simulink model "Dinamica_numerica_MPC"  (R2024b)
settings: Solver=ode4  StartTime=0.0  StopTime=Durata_sim  FixedStep=step_num  RelTol=1e-6
values from neighbouring files (symbols this model uses):
  a_c0 = 6771    [Propagation_outofplane_transfer.m]
  B_c = C_Dc*S_c/mass_c    (= 0)    [Propagation_outofplane_transfer.m]
  B_d = C_Dd*S_d/mass_d    (= 1.05e-08)    [Propagation_outofplane_transfer.m]
  D = zeros(ny,3)    [final_controller_1deputy2.m]
  delta_a0 = 0    [Propagation_outofplane_transfer.m]
  delta_B = (B_d-B_c)/B_d    (= 1)    [Propagation_outofplane_transfer.m]
  delta_e_x0 = 0    [Propagation_outofplane_transfer.m]
  delta_e_y0 = 0.2/a_c0    (= 2.95377344558e-05)    [Propagation_outofplane_transfer.m]
  delta_i_x0 = 0    [Propagation_outofplane_transfer.m]
  delta_i_y0 = 0.18/a_c0    (= 2.65839610102e-05)    [Propagation_outofplane_transfer.m]
  delta_lambda0 = 0    [Propagation_outofplane_transfer.m]
  e_c0 = 0.001    [Propagation_outofplane_transfer.m]
  i_c0 = 97.05 * pi/180    (= 1.69384203906)    [Propagation_outofplane_transfer.m]
  J_2 = 1.08263e-3    (= 0.00108263)    [Propagation_outofplane_transfer.m]
  M_c0 = 0 * pi/180    (= 0)    [Propagation_outofplane_transfer.m]
  mu = 3.986e5    (= 398600)    [Propagation_outofplane_transfer.m]
  OM_c0 = 30 * pi/180    (= 0.523598775598)    [Propagation_outofplane_transfer.m]
  om_c0 = 90 * pi/180    (= 1.57079632679)    [Propagation_outofplane_transfer.m]
  R_E = 6378    [Propagation_outofplane_transfer.m]
  rho = 1.05259630795205e-3    (= 0.00105259630795)    [Propagation_outofplane_transfer.m]
  ROE_T = [delta_aT,delta_lambdaT,delta_e_xT,delta_e_yT, delta_i_xT, delta_i_yT, delta_B]'    [Propagation_outofplane_transfer.m]
  S_c = 0.1*(1e-3)^2    (= 1e-07)    [Propagation_outofplane_transfer.m]
  S_d = 0.1*(1e-3)^2    (= 1e-07)    [Propagation_outofplane_transfer.m]
  T_orbit = 2*pi/n_c0    [Propagation_outofplane_transfer.m]
  Ts = 100    [Propagation_outofplane_transfer.m]
  u_max = max_thrust/mass_d    (= 3.25e-08)    [Propagation_outofplane_transfer.m]    (also in final_controller_1deputy2.m = 0.0325)
  u_min = min_thrust/mass_d    (= 1.75e-08)    [Propagation_outofplane_transfer.m]    (also in final_controller_1deputy2.m = 0.0175)
undefined symbols (not defined in the file or in its folder): final_controller_1deputy2, inputs4JB2008, JB2008, M_0, OMEGA_c0, omega_c0
libraries: spsMeanLib x6, simulink x3, simulink_extras x2
(part 2 of 4)

== matlab function Dinamica_numerica_MPC/Linearized ROE computing ==
  settings: updateMethod=DISCRETE
  data: ROE input; J_2 input; rho input; A output; OE_c input; B_c input; B_d input; B output
function [A,B] = matrices_comput(ROE, J_2, rho, OE_c, B_c, B_d)
%%%%%%%%%%%%%%%%%%%%%%%%%%%%%%%%%%%%%%%%%%%%%%%%%%%%%%%%%%%%%%%%%%%%%%
% DOCUMENTATION:
% The following function propagate the Relative Orbital Elements (ROE)
% of a Deputy satellite wrt a Chief satellite with known chief OE.
% The orbit dynamics is expressed in linearized form such that the
% dynamics of chief-deputy system can be expressed by the following:
% -     dx = (A_kep + A_J2 + A_drag) * x + B * u
% where A_kep is the State Transition Matrix (STM) representing the EoM
% of a keplerian two-body system, A_J2 is the STM embedding the J2
% effect, and A_drag is the STM that take into account the approximated
% drag model. Note that the perturbation STM are time-varying matricies, thus the model
% can be updated with a certain externally defined period
% 
% INPUTS:
% - x       -> ROE of Deputy satellite wrt Chief
% - u       -> Input thrust dor the Deputy satellite
% - trg     -> Trigger signal for STM update
% - pert_flg-> Perturbation flags: (1) J2, (2) Drag
% - OEc     -> Chief orbit element organized
% 
% OUTPUTS:
% - dx      -> ROE derivate
% 
% REFEREBCES:           %TO BE ADDED
% []
% []
% []

%%%%%%%%%%%%%%%%%%%%%%%%%%%%%%%%%%%%%%%%%%%%%%%%%%%%%%%%%%%%%%%%%%%%%%


mu  = 3.986e5;
R_E = 6378;

a_c  = OE_c(1);
e_c  = OE_c(2);
i_c  = OE_c(3);

i_c = mod(i_c, 2*pi);        % assicura che i sia tra 0 e 2π
if i_c > pi
    i_c = 2*pi - i_c;             % lo porta nel range [0, π]
end

OM_c = OE_c(4);
OM_c = mod(OM_c, 2*pi);
om_c = OE_c(5);
om_c = mod(om_c, 2*pi);
M_c  = OE_c(6);
M_c = mod(M_c, 2*pi);





% nu_c= mean2true(M_c,e_c);
% Io invece farei:
nu_c = Tempo_inverso_aggiustato(M_c, a_c, e_c);
n_c = sqrt(mu/a_c^3);
u_c = om_c + M_c;
p_c   = a_c*(1-e_c^2);
v_c = sqrt(mu/p_c)*sqrt(2*(1+e_c*cos(nu_c))-(1-e_c^2));

% Keplerian EoM STM

A_kep = zeros(7);
A_kep(2,1) = -3/2 * n_c;


eta  = sqrt(1-e_c^2);
k_J2 = 3/4*J_2*R_E^2*sqrt(mu)/(a_c^3.5*eta^4);
e_xc  = e_c*cos(om_c);
e_yc  = e_c*sin(om_c);
E    = 1 + eta;
F    = 4 + 3*eta;
G    = 1/eta^2;
P    = 3*cos(i_c)^2 - 1;
Q    = 5*cos(i_c)^2 - 1;
S    = sin(2*i_c);
T    = sin(i_c)^2;

%%%%%%%%%%%%%%%%%%%%%%%%%%%%%%%%%%%%%%%%%%%%%%%%%%%%%%%%%%%%%%%%%%%%%%%%%%%%%%%%%%%%%%%%%%%%%%%%%%%%%%%%%%%%%%%%%%%%%%%%%%%
% J2 plant matrix computation

% Versione del paper di Guffanti (e anche tesi di Belloni, tranne per un
% errore di copiatura, secondo me, che ho aggiustato)
%(è quella che sto usando al momento)
A_J2 = k_J2.*[zeros(1,7);
              -7/2*E*P, 0, e_xc*G*F*P, e_yc*G*F*P, -F*S, 0, 0;
              7/2*e_yc*Q, 0, -4*e_xc*e_yc*G*Q, -(1+4*G*e_yc^2)*Q, 5*e_yc*S, 0, 0;
              -7/2*e_xc*Q, 0, (1+4*G*e_xc^2)*Q, 4*e_xc*e_yc*G*Q, -5*e_xc*S, 0, 0;
              zeros(1,7);
              7/2*S, 0, -4*e_xc*G*S, -4*e_yc*G*S, 2*T, 0, 0;
              zeros(1,7)];


delta_a = ROE(1);
delta_lambda = ROE(2);
delta_e_x = ROE(3);
delta_e_y=ROE(4);
delta_i_x=ROE(5);
delta_i_y=ROE(6);

%%%%%%%%%%%%%%%%%%%%%%%%%%%%%%%%%%%%%%%%%%%%%%%%%%%%%%%%%%%%%%%%%%%%%%%%%%%%%%%%%%%%%%%%%%%%%%%%%%%%%%%%%%%%%%%%%%%%%%%%%%%%%%%%%%%%%%%%%%%%%%%%%%%%%%%%%%%%%%%%%%%%%%%%%%%%%%%%%

% Drag plant matrix


a_d   = a_c*(delta_a+1);
e_xd = e_xc+delta_e_x;
e_yd = e_yc+delta_e_y;
e_d = sqrt(e_xd^2+e_yd^2);
om_d  = atan2(e_yd,e_xd);
om_d = mod(om_d, 2*pi);
i_d = i_c + delta_i_x;
i_d = mod(i_d, 2*pi);        % assicura che i sia tra 0 e 2π
if i_d > pi
    i_d = 2*pi - i_d;             % lo porta nel range [0, π]
end

OM_d = OM_c + delta_i_y/sin(i_c);
OM_d = mod(OM_d, 2*pi);
u_d = u_c - delta_i_y/tan(i_c) + delta_lambda;
u_d = mod(u_d, 2*pi);
M_d = u_d - om_d;
M_d = mod(M_d, 2*pi);



nu_d = Tempo_inverso_aggiustato(M_d, a_d, e_d);
p_d   = a_d*(1-e_d^2);
v_d = sqrt(mu/p_d)*sqrt(2*(1+e_d*cos(nu_d))-(1-e_d^2));
b_d = a_d*sqrt(1-e_d^2); % semiasse minore dell'orbita del deputy
r_d = p_d/(1+e_d*cos(nu_d));

A_drag = zeros(7,7);
delta_M = M_d - M_c;
delta_e = e_d - e_c;
delta_om = om_d - om_c;
delta_i = i_d - i_c;
delta_OM = OM_d - OM_c;

u_drag = 0.5*B_d*rho*v_d^2; % accelerazione dovuta alla resistenza in valore assoluto



%-----------------------------------------------------------------------------------------

% Quella che ho ricavato io NON NINEARIZZANDO, considerando anche delta_lambda_dot, è:
% (è quella che sto usando al momento e che ho usato per ottenere i risultati mostrati a Thales)
% NON CAMBIA NULLA A LIVELLO DI RISULTATI SE USI QUELLA MESSA NELLA TESI,
% PER QUESTO AL MOMENTO USO QUESTA.

delta_B = (B_d-B_c)/B_d; % definizione usata nella tesi di Belloni
A_drag(1:4,7) = - u_drag.*[2*a_d^2 * v_d/(mu*a_c);
                           2/(e_d*v_d)*sin(nu_d)*(1-b_d/a_d*(1+e_d^2*r_d/p_d));
                           2/v_d*((e_d+cos(nu_d))*cos(om_d)-sin(nu_d)*sin(om_d));
                           2/v_d*((e_d+cos(nu_d))*sin(om_d)+sin(nu_d)*cos(om_d))];



%------------------------------------------------------------------------------
% versione linearizzata con definizione di delta_B di Guffanti (cioè quella
% che ho inserito nella tesi)
% 

% delta_B = B_d - B_c; % definizione del paper di Guffanti
% A_drag(1,1) = 0;
% A_drag(1,2) = 0;
% A_drag(1,3) = 0;
% A_drag(1,4) = 0;
% A_drag(1,5) = 0;
% A_drag(1,6) = 0;
% A_drag(1,7) = -(a_c*rho*v_c^3)/mu;
% A_drag(2,1) = 0;
% A_drag(2,2) = 0;
% A_drag(2,3) = 0;
% A_drag(2,4) = 0;
% A_drag(2,5) = 0;
% A_drag(2,6) = 0;
% A_drag(2,7) = 0;
% A_drag(3,1) = 0;
% A_drag(3,2) = 0;
% A_drag(3,3) = 0;
% A_drag(3,4) = 0;
% A_drag(3,5) = 0;
% A_drag(3,6) = 0;
% A_drag(3,7) = rho*v_c*(sin(nu_c)*sin(om_c) - cos(om_c)*(e_c + cos(nu_c)));
% A_drag(4,1) = 0;
% A_drag(4,2) = 0;
% A_drag(4,3) = 0;
% A_drag(4,4) = 0;
% A_drag(4,5) = 0;
% A_drag(4,6) = 0;
% A_drag(4,7) = -rho*v_c*(cos(om_c)*sin(nu_c) + sin(om_c)*(e_c + cos(nu_c)));
% A_drag(5,1) = 0;
% A_drag(5,2) = 0;
% A_drag(5,3) = 0;
% A_drag(5,4) = 0;
% A_drag(5,5) = 0;
% A_drag(5,6) = 0;
% A_drag(5,7) = 0;
% A_drag(6,1) = 0;
% A_drag(6,2) = 0;
% A_drag(6,3) = 0;
% A_drag(6,4) = 0;
% A_drag(6,5) = 0;
% A_drag(6,6) = 0;
% A_drag(6,7) = 0;
% A_drag(7,1) = 0;
% A_drag(7,2) = 0;
% A_drag(7,3) = 0;
% A_drag(7,4) = 0;
% A_drag(7,5) = 0;
% A_drag(7,6) = 0;
% A_drag(7,7) = 0;


%------------------------------------------------------------------------
% versione linearizzata con definizione di delta_B di Koenig

% delta_B = (B_d-B_c)/B_c; % definizione di Koenig
% A_drag(1,1) = ((B_c*a_c*rho*(delta_B + 1)*(-mu/(a_c*(e_xc^2 + e_yc^2 - 1)))^(1/2)*(2*cos(u_c - atan2(e_yc, e_xc) + (13*sin(3*u_c - 3*atan2(e_yc, e_xc))*(e_xc^2 + e_yc^2)^(3/2))/12 + sin(u_c - atan2(e_yc, e_xc))*(2*(e_xc^2 + e_yc^2)^(1/2) - (e_xc^2 + e_yc^2)^(3/2)/4) + sin(2*u_c - 2*atan2(e_yc, e_xc))*((5*e_xc^2)/4 + (5*e_yc^2)/4))*(e_xc^2 + e_yc^2)^(1/2) + e_xc^2 + e_yc^2 + 1)^(3/2))/(e_xc^2 + e_yc^2 - 1) + (B_c*mu*rho*(delta_B + 1)*(2*cos(u_c - atan2(e_yc, e_xc) + (13*sin(3*u_c - 3*atan2(e_yc, e_xc))*(e_xc^2 + e_yc^2)^(3/2))/12 + sin(u_c - atan2(e_yc, e_xc))*(2*(e_xc^2 + e_yc^2)^(1/2) - (e_xc^2 + e_yc^2)^(3/2)/4) + sin(2*u_c - 2*atan2(e_yc, e_xc))*((5*e_xc^2)/4 + (5*e_yc^2)/4))*(e_xc^2 + e_yc^2)^(1/2) + e_xc^2 + e_yc^2 + 1)^(3/2))/(2*(-mu/(a_c*(e_xc^2 + e_yc^2 - 1)))^(1/2)*(e_xc^2 + e_yc^2 - 1)^2))/a_c - (B_c*rho*(-mu/(a_c*(e_c^2 - 1)))^(1/2)*(e_c^2 + 2*e_c*cos(M_c + (5*e_c^2*sin(2*M_c))/4 + (13*e_c^3*sin(3*M_c))/12 + sin(M_c)*(2*e_c - e_c^3/4)) + 1)^(3/2))/(e_c^2 - 1);
% A_drag(1,2) = -(3*B_c*rho*sin(u_c - atan2(e_yc, e_xc) + (13*sin(3*u_c - 3*atan2(e_yc, e_xc))*(e_xc^2 + e_yc^2)^(3/2))/12 + sin(u_c - atan2(e_yc, e_xc))*(2*(e_xc^2 + e_yc^2)^(1/2) - (e_xc^2 + e_yc^2)^(3/2)/4) + sin(2*u_c - 2*atan2(e_yc, e_xc))*((5*e_xc^2)/4 + (5*e_yc^2)/4))*(delta_B + 1)*(e_xc^2 + e_yc^2)^(1/2)*(-mu/(a_c*(e_xc^2 + e_yc^2 - 1)))^(1/2)*(2*cos(u_c - atan2(e_yc, e_xc) + (13*sin(3*u_c - 3*atan2(e_yc, e_xc))*(e_xc^2 + e_yc^2)^(3/2))/12 + sin(u_c - atan2(e_yc, e_xc))*(2*(e_xc^2 + e_yc^2)^(1/2) - (e_xc^2 + e_yc^2)^(3/2)/4) + sin(2*u_c - 2*atan2(e_yc, e_xc))*((5*e_xc^2)/4 + (5*e_yc^2)/4))*(e_xc^2 + e_yc^2)^(1/2) + e_xc^2 + e_yc^2 + 1)^(1/2)*((13*cos(3*u_c - 3*atan2(e_yc, e_xc))*(e_xc^2 + e_yc^2)^(3/2))/4 + cos(u_c - atan2(e_yc, e_xc))*(2*(e_xc^2 + e_yc^2)^(1/2) - (e_xc^2 + e_yc^2)^(3/2)/4) + 2*cos(2*u_c - 2*atan2(e_yc, e_xc))*((5*e_xc^2)/4 + (5*e_yc^2)/4) + 1))/(e_xc^2 + e_yc^2 - 1);
% A_drag(1,3) = ((3*B_c*a_c*rho*(delta_B + 1)*(2*e_xc + (2*e_xc*cos(u_c - atan2(e_yc, e_xc) + (13*sin(3*u_c - 3*atan2(e_yc, e_xc))*(e_xc^2 + e_yc^2)^(3/2))/12 + sin(u_c - atan2(e_yc, e_xc))*(2*(e_xc^2 + e_yc^2)^(1/2) - (e_xc^2 + e_yc^2)^(3/2)/4) + sin(2*u_c - 2*atan2(e_yc, e_xc))*((5*e_xc^2)/4 + (5*e_yc^2)/4)))/(e_xc^2 + e_yc^2)^(1/2) - 2*sin(u_c - atan2(e_yc, e_xc) + (13*sin(3*u_c - 3*atan2(e_yc, e_xc))*(e_xc^2 + e_yc^2)^(3/2))/12 + sin(u_c - atan2(e_yc, e_xc))*(2*(e_xc^2 + e_yc^2)^(1/2) - (e_xc^2 + e_yc^2)^(3/2)/4) + sin(2*u_c - 2*atan2(e_yc, e_xc))*((5*e_xc^2)/4 + (5*e_yc^2)/4))*(e_xc^2 + e_yc^2)^(1/2)*(e_yc/(e_xc^2 + e_yc^2) + sin(u_c - atan2(e_yc, e_xc))*((2*e_xc)/(e_xc^2 + e_yc^2)^(1/2) - (3*e_xc*(e_xc^2 + e_yc^2)^(1/2))/4) + (5*e_xc*sin(2*u_c - 2*atan2(e_yc, e_xc)))/2 + (13*e_yc*cos(3*u_c - 3*atan2(e_yc, e_xc))*(e_xc^2 + e_yc^2)^(1/2))/4 + (13*e_xc*sin(3*u_c - 3*atan2(e_yc, e_xc))*(e_xc^2 + e_yc^2)^(1/2))/4 + (e_yc*cos(u_c - atan2(e_yc, e_xc))*(2*(e_xc^2 + e_yc^2)^(1/2) - (e_xc^2 + e_yc^2)^(3/2)/4))/(e_xc^2 + e_yc^2) + (2*e_yc*cos(2*u_c - 2*atan2(e_yc, e_xc))*((5*e_xc^2)/4 + (5*e_yc^2)/4))/(e_xc^2 + e_yc^2)))*(-mu/(a_c*(e_xc^2 + e_yc^2 - 1)))^(1/2)*(2*cos(u_c - atan2(e_yc, e_xc) + (13*sin(3*u_c - 3*atan2(e_yc, e_xc))*(e_xc^2 + e_yc^2)^(3/2))/12 + sin(u_c - atan2(e_yc, e_xc))*(2*(e_xc^2 + e_yc^2)^(1/2) - (e_xc^2 + e_yc^2)^(3/2)/4) + sin(2*u_c - 2*atan2(e_yc, e_xc))*((5*e_xc^2)/4 + (5*e_yc^2)/4))*(e_xc^2 + e_yc^2)^(1/2) + e_xc^2 + e_yc^2 + 1)^(1/2))/(2*(e_xc^2 + e_yc^2 - 1)) - (2*B_c*a_c*e_xc*rho*(delta_B + 1)*(-mu/(a_c*(e_xc^2 + e_yc^2 - 1)))^(1/2)*(2*cos(u_c - atan2(e_yc, e_xc) + (13*sin(3*u_c - 3*atan2(e_yc, e_xc))*(e_xc^2 + e_yc^2)^(3/2))/12 + sin(u_c - atan2(e_yc, e_xc))*(2*(e_xc^2 + e_yc^2)^(1/2) - (e_xc^2 + e_yc^2)^(3/2)/4) + sin(2*u_c - 2*atan2(e_yc, e_xc))*((5*e_xc^2)/4 + (5*e_yc^2)/4))*(e_xc^2 + e_yc^2)^(1/2) + e_xc^2 + e_yc^2 + 1)^(3/2))/(e_xc^2 + e_yc^2 - 1)^2 + (B_c*e_xc*mu*rho*(delta_B + 1)*(2*cos(u_c - atan2(e_yc, e_xc) + (13*sin(3*u_c - 3*atan2(e_yc, e_xc))*(e_xc^2 + e_yc^2)^(3/2))/12 + sin(u_c - atan2(e_yc, e_xc))*(2*(e_xc^2 + e_yc^2)^(1/2) - (e_xc^2 + e_yc^2)^(3/2)/4) + sin(2*u_c - 2*atan2(e_yc, e_xc))*((5*e_xc^2)/4 + (5*e_yc^2)/4))*(e_xc^2 + e_yc^2)^(1/2) + e_xc^2 + e_yc^2 + 1)^(3/2))/((-mu/(a_c*(e_xc^2 + e_yc^2 - 1)))^(1/2)*(e_xc^2 + e_yc^2 - 1)^3))/a_c;
% A_drag(1,4) = ((3*B_c*a_c*rho*(delta_B + 1)*(2*e_yc + (2*e_yc*cos(u_c - atan2(e_yc, e_xc) + (13*sin(3*u_c - 3*atan2(e_yc, e_xc))*(e_xc^2 + e_yc^2)^(3/2))/12 + sin(u_c - atan2(e_yc, e_xc))*(2*(e_xc^2 + e_yc^2)^(1/2) - (e_xc^2 + e_yc^2)^(3/2)/4) + sin(2*u_c - 2*atan2(e_yc, e_xc))*((5*e_xc^2)/4 + (5*e_yc^2)/4)))/(e_xc^2 + e_yc^2)^(1/2) + 2*sin(u_c - atan2(e_yc, e_xc) + (13*sin(3*u_c - 3*atan2(e_yc, e_xc))*(e_xc^2 + e_yc^2)^(3/2))/12 + sin(u_c - atan2(e_yc, e_xc))*(2*(e_xc^2 + e_yc^2)^(1/2) - (e_xc^2 + e_yc^2)^(3/2)/4) + sin(2*u_c - 2*atan2(e_yc, e_xc))*((5*e_xc^2)/4 + (5*e_yc^2)/4))*(e_xc^2 + e_yc^2)^(1/2)*(e_xc/(e_xc^2 + e_yc^2) - sin(u_c - atan2(e_yc, e_xc))*((2*e_yc)/(e_xc^2 + e_yc^2)^(1/2) - (3*e_yc*(e_xc^2 + e_yc^2)^(1/2))/4) - (5*e_yc*sin(2*u_c - 2*atan2(e_yc, e_xc)))/2 + (13*e_xc*cos(3*u_c - 3*atan2(e_yc, e_xc))*(e_xc^2 + e_yc^2)^(1/2))/4 - (13*e_yc*sin(3*u_c - 3*atan2(e_yc, e_xc))*(e_xc^2 + e_yc^2)^(1/2))/4 + (e_xc*cos(u_c - atan2(e_yc, e_xc))*(2*(e_xc^2 + e_yc^2)^(1/2) - (e_xc^2 + e_yc^2)^(3/2)/4))/(e_xc^2 + e_yc^2) + (2*e_xc*cos(2*u_c - 2*atan2(e_yc, e_xc))*((5*e_xc^2)/4 + (5*e_yc^2)/4))/(e_xc^2 + e_yc^2)))*(-mu/(a_c*(e_xc^2 + e_yc^2 - 1)))^(1/2)*(2*cos(u_c - atan2(e_yc, e_xc) + (13*sin(3*u_c - 3*atan2(e_yc, e_xc))*(e_xc^2 + e_yc^2)^(3/2))/12 + sin(u_c - atan2(e_yc, e_xc))*(2*(e_xc^2 + e_yc^2)^(1/2) - (e_xc^2 + e_yc^2)^(3/2)/4) + sin(2*u_c - 2*atan2(e_yc, e_xc))*((5*e_xc^2)/4 + (5*e_yc^2)/4))*(e_xc^2 + e_yc^2)^(1/2) + e_xc^2 + e_yc^2 + 1)^(1/2))/(2*(e_xc^2 + e_yc^2 - 1)) - (2*B_c*a_c*e_yc*rho*(delta_B + 1)*(-mu/(a_c*(e_xc^2 + e_yc^2 - 1)))^(1/2)*(2*cos(u_c - atan2(e_yc, e_xc) + (13*sin(3*u_c - 3*atan2(e_yc, e_xc))*(e_xc^2 + e_yc^2)^(3/2))/12 + sin(u_c - atan2(e_yc, e_xc))*(2*(e_xc^2 + e_yc^2)^(1/2) - (e_xc^2 + e_yc^2)^(3/2)/4) + sin(2*u_c - 2*atan2(e_yc, e_xc))*((5*e_xc^2)/4 + (5*e_yc^2)/4))*(e_xc^2 + e_yc^2)^(1/2) + e_xc^2 + e_yc^2 + 1)^(3/2))/(e_xc^2 + e_yc^2 - 1)^2 + (B_c*e_yc*mu*rho*(delta_B + 1)*(2*cos(u_c - atan2(e_yc, e_xc) + (13*sin(3*u_c - 3*atan2(e_yc, e_xc))*(e_xc^2 + e_yc^2)^(3/2))/12 + sin(u_c - atan2(e_yc, e_xc))*(2*(e_xc^2 + e_yc^2)^(1/2) - (e_xc^2 + e_yc^2)^(3/2)/4) + sin(2*u_c - 2*atan2(e_yc, e_xc))*((5*e_xc^2)/4 + (5*e_yc^2)/4))*(e_xc^2 + e_yc^2)^(1/2) + e_xc^2 + e_yc^2 + 1)^(3/2))/((-mu/(a_c*(e_xc^2 + e_yc^2 - 1)))^(1/2)*(e_xc^2 + e_yc^2 - 1)^3))/a_c;
% A_drag(1,5) = 0;
% A_drag(1,6) = (3*B_c*rho*sin(u_c - atan2(e_yc, e_xc) + (13*sin(3*u_c - 3*atan2(e_yc, e_xc))*(e_xc^2 + e_yc^2)^(3/2))/12 + sin(u_c - atan2(e_yc, e_xc))*(2*(e_xc^2 + e_yc^2)^(1/2) - (e_xc^2 + e_yc^2)^(3/2)/4) + sin(2*u_c - 2*atan2(e_yc, e_xc))*((5*e_xc^2)/4 + (5*e_yc^2)/4))*(delta_B + 1)*(e_xc^2 + e_yc^2)^(1/2)*(-mu/(a_c*(e_xc^2 + e_yc^2 - 1)))^(1/2)*(2*cos(u_c - atan2(e_yc, e_xc) + (13*sin(3*u_c - 3*atan2(e_yc, e_xc))*(e_xc^2 + e_yc^2)^(3/2))/12 + sin(u_c - atan2(e_yc, e_xc))*(2*(e_xc^2 + e_yc^2)^(1/2) - (e_xc^2 + e_yc^2)^(3/2)/4) + sin(2*u_c - 2*atan2(e_yc, e_xc))*((5*e_xc^2)/4 + (5*e_yc^2)/4))*(e_xc^2 + e_yc^2)^(1/2) + e_xc^2 + e_yc^2 + 1)^(1/2)*(1/tan(i_c) + (2*cos(2*u_c - 2*atan2(e_yc, e_xc))*((5*e_xc^2)/4 + (5*e_yc^2)/4))/tan(i_c) + (13*cos(3*u_c - 3*atan2(e_yc, e_xc))*(e_xc^2 + e_yc^2)^(3/2))/(4*tan(i_c)) + (cos(u_c - atan2(e_yc, e_xc))*(2*(e_xc^2 + e_yc^2)^(1/2) - (e_xc^2 + e_yc^2)^(3/2)/4))/tan(i_c)))/(e_xc^2 + e_yc^2 - 1);
% A_drag(1,7) = (B_c*rho*(-mu/(a_c*(e_xc^2 + e_yc^2 - 1)))^(1/2)*(2*cos(u_c - atan2(e_yc, e_xc) + (13*sin(3*u_c - 3*atan2(e_yc, e_xc))*(e_xc^2 + e_yc^2)^(3/2))/12 + sin(u_c - atan2(e_yc, e_xc))*(2*(e_xc^2 + e_yc^2)^(1/2) - (e_xc^2 + e_yc^2)^(3/2)/4) + sin(2*u_c - 2*atan2(e_yc, e_xc))*((5*e_xc^2)/4 + (5*e_yc^2)/4))*(e_xc^2 + e_yc^2)^(1/2) + e_xc^2 + e_yc^2 + 1)^(3/2))/(e_xc^2 + e_yc^2 - 1);
% A_drag(2,1) = (B_c*mu^2*rho*sin(u_c - atan2(e_yc, e_xc) + (13*sin(3*u_c - 3*atan2(e_yc, e_xc))*(e_xc^2 + e_yc^2)^(3/2))/12 + sin(u_c - atan2(e_yc, e_xc))*(2*(e_xc^2 + e_yc^2)^(1/2) - (e_xc^2 + e_yc^2)^(3/2)/4) + sin(2*u_c - 2*atan2(e_yc, e_xc))*((5*e_xc^2)/4 + (5*e_yc^2)/4))*(delta_B + 1)*((e_xc^2 + e_yc^2)/(cos(u_c - atan2(e_yc, e_xc) + (13*sin(3*u_c - 3*atan2(e_yc, e_xc))*(e_xc^2 + e_yc^2)^(3/2))/12 + sin(u_c - atan2(e_yc, e_xc))*(2*(e_xc^2 + e_yc^2)^(1/2) - (e_xc^2 + e_yc^2)^(3/2)/4) + sin(2*u_c - 2*atan2(e_yc, e_xc))*((5*e_xc^2)/4 + (5*e_yc^2)/4))*(e_xc^2 + e_yc^2)^(1/2) + 1) + 1)*(2*cos(u_c - atan2(e_yc, e_xc) + (13*sin(3*u_c - 3*atan2(e_yc, e_xc))*(e_xc^2 + e_yc^2)^(3/2))/12 + sin(u_c - atan2(e_yc, e_xc))*(2*(e_xc^2 + e_yc^2)^(1/2) - (e_xc^2 + e_yc^2)^(3/2)/4) + sin(2*u_c - 2*atan2(e_yc, e_xc))*((5*e_xc^2)/4 + (5*e_yc^2)/4))*(e_xc^2 + e_yc^2)^(1/2) + e_xc^2 + e_yc^2 + 1)^(1/2))/(2*a_c^2*(e_xc^2 + e_yc^2)^(1/2)*(-mu/(a_c*(e_xc^2 + e_yc^2 - 1)))^(3/2)*(1 - e_yc^2 - e_xc^2)^(3/2)) - (B_c*mu^2*rho*sin(u_c - atan2(e_yc, e_xc) + (13*sin(3*u_c - 3*atan2(e_yc, e_xc))*(e_xc^2 + e_yc^2)^(3/2))/12 + sin(u_c - atan2(e_yc, e_xc))*(2*(e_xc^2 + e_yc^2)^(1/2) - (e_xc^2 + e_yc^2)^(3/2)/4) + sin(2*u_c - 2*atan2(e_yc, e_xc))*((5*e_xc^2)/4 + (5*e_yc^2)/4))*(delta_B + 1)*(2*cos(u_c - atan2(e_yc, e_xc) + (13*sin(3*u_c - 3*atan2(e_yc, e_xc))*(e_xc^2 + e_yc^2)^(3/2))/12 + sin(u_c - atan2(e_yc, e_xc))*(2*(e_xc^2 + e_yc^2)^(1/2) - (e_xc^2 + e_yc^2)^(3/2)/4) + sin(2*u_c - 2*atan2(e_yc, e_xc))*((5*e_xc^2)/4 + (5*e_yc^2)/4))*(e_xc^2 + e_yc^2)^(1/2) + e_xc^2 + e_yc^2 + 1)^(1/2))/(2*a_c^2*(e_xc^2 + e_yc^2)^(1/2)*(-mu/(a_c*(e_xc^2 + e_yc^2 - 1)))^(3/2)*(e_xc^2 + e_yc^2 - 1)^2) - (B_c*mu*rho*sin(u_c - atan2(e_yc, e_xc) + (13*sin(3*u_c - 3*atan2(e_yc, e_xc))*(e_xc^2 + e_yc^2)^(3/2))/12 + sin(u_c - atan2(e_yc, e_xc))*(2*(e_xc^2 + e_yc^2)^(1/2) - (e_xc^2 + e_yc^2)^(3/2)/4) + sin(2*u_c - 2*atan2(e_yc, e_xc))*((5*e_xc^2)/4 + (5*e_yc^2)/4))*(delta_B + 1)*(2*cos(u_c - atan2(e_yc, e_xc) + (13*sin(3*u_c - 3*atan2(e_yc, e_xc))*(e_xc^2 + e_yc^2)^(3/2))/12 + sin(u_c - atan2(e_yc, e_xc))*(2*(e_xc^2 + e_yc^2)^(1/2) - (e_xc^2 + e_yc^2)^(3/2)/4) + sin(2*u_c - 2*atan2(e_yc, e_xc))*((5*e_xc^2)/4 + (5*e_yc^2)/4))*(e_xc^2 + e_yc^2)^(1/2) + e_xc^2 + e_yc^2 + 1)^(1/2))/(a_c*(e_xc^2 + e_yc^2)^(1/2)*(-mu/(a_c*(e_xc^2 + e_yc^2 - 1)))^(1/2)*(e_xc^2 + e_yc^2 - 1)) - (B_c*mu*rho*sin(u_c - atan2(e_yc, e_xc) + (13*sin(3*u_c - 3*atan2(e_yc, e_xc))*(e_xc^2 + e_yc^2)^(3/2))/12 + sin(u_c - atan2(e_yc, e_xc))*(2*(e_xc^2 + e_yc^2)^(1/2) - (e_xc^2 + e_yc^2)^(3/2)/4) + sin(2*u_c - 2*atan2(e_yc, e_xc))*((5*e_xc^2)/4 + (5*e_yc^2)/4))*(delta_B + 1)*((e_xc^2 + e_yc^2)/(cos(u_c - atan2(e_yc, e_xc) + (13*sin(3*u_c - 3*atan2(e_yc, e_xc))*(e_xc^2 + e_yc^2)^(3/2))/12 + sin(u_c - atan2(e_yc, e_xc))*(2*(e_xc^2 + e_yc^2)^(1/2) - (e_xc^2 + e_yc^2)^(3/2)/4) + sin(2*u_c - 2*atan2(e_yc, e_xc))*((5*e_xc^2)/4 + (5*e_yc^2)/4))*(e_xc^2 + e_yc^2)^(1/2) + 1) + 1)*(2*cos(u_c - atan2(e_yc, e_xc) + (13*sin(3*u_c - 3*atan2(e_yc, e_xc))*(e_xc^2 + e_yc^2)^(3/2))/12 + sin(u_c - atan2(e_yc, e_xc))*(2*(e_xc^2 + e_yc^2)^(1/2) - (e_xc^2 + e_yc^2)^(3/2)/4) + sin(2*u_c - 2*atan2(e_yc, e_xc))*((5*e_xc^2)/4 + (5*e_yc^2)/4))*(e_xc^2 + e_yc^2)^(1/2) + e_xc^2 + e_yc^2 + 1)^(1/2))/(a_c*(e_xc^2 + e_yc^2)^(1/2)*(-mu/(a_c*(e_xc^2 + e_yc^2 - 1)))^(1/2)*(1 - e_yc^2 - e_xc^2)^(1/2));
% A_drag(2,2) = (B_c*mu*rho*sin(u_c - atan2(e_yc, e_xc) + (13*sin(3*u_c - 3*atan2(e_yc, e_xc))*(e_xc^2 + e_yc^2)^(3/2))/12 + sin(u_c - atan2(e_yc, e_xc))*(2*(e_xc^2 + e_yc^2)^(1/2) - (e_xc^2 + e_yc^2)^(3/2)/4) + sin(2*u_c - 2*atan2(e_yc, e_xc))*((5*e_xc^2)/4 + (5*e_yc^2)/4))^2*(delta_B + 1)*((13*cos(3*u_c - 3*atan2(e_yc, e_xc))*(e_xc^2 + e_yc^2)^(3/2))/4 + cos(u_c - atan2(e_yc, e_xc))*(2*(e_xc^2 + e_yc^2)^(1/2) - (e_xc^2 + e_yc^2)^(3/2)/4) + 2*cos(2*u_c - 2*atan2(e_yc, e_xc))*((5*e_xc^2)/4 + (5*e_yc^2)/4) + 1))/(a_c*(e_c^2 - 1)*(-mu/(a_c*(e_c^2 - 1)))^(1/2)*(2*e_c*cos(u_c - atan2(e_yc, e_xc) + (13*sin(3*u_c - 3*atan2(e_yc, e_xc))*(e_xc^2 + e_yc^2)^(3/2))/12 + sin(u_c - atan2(e_yc, e_xc))*(2*(e_xc^2 + e_yc^2)^(1/2) - (e_xc^2 + e_yc^2)^(3/2)/4) + sin(2*u_c - 2*atan2(e_yc, e_xc))*((5*e_xc^2)/4 + (5*e_yc^2)/4)) + e_c^2 + 1)^(1/2)) - (B_c*mu*rho*sin(u_c - atan2(e_yc, e_xc) + (13*sin(3*u_c - 3*atan2(e_yc, e_xc))*(e_xc^2 + e_yc^2)^(3/2))/12 + sin(u_c - atan2(e_yc, e_xc))*(2*(e_xc^2 + e_yc^2)^(1/2) - (e_xc^2 + e_yc^2)^(3/2)/4) + sin(2*u_c - 2*atan2(e_yc, e_xc))*((5*e_xc^2)/4 + (5*e_yc^2)/4))^2*(delta_B + 1)*((13*cos(3*u_c - 3*atan2(e_yc, e_xc))*(e_xc^2 + e_yc^2)^(3/2))/4 + cos(u_c - atan2(e_yc, e_xc))*(2*(e_xc^2 + e_yc^2)^(1/2) - (e_xc^2 + e_yc^2)^(3/2)/4) + 2*cos(2*u_c - 2*atan2(e_yc, e_xc))*((5*e_xc^2)/4 + (5*e_yc^2)/4) + 1))/(a_c*(-mu/(a_c*(e_xc^2 + e_yc^2 - 1)))^(1/2)*(e_xc^2 + e_yc^2 - 1)*(2*cos(u_c - atan2(e_yc, e_xc) + (13*sin(3*u_c - 3*atan2(e_yc, e_xc))*(e_xc^2 + e_yc^2)^(3/2))/12 + sin(u_c - atan2(e_yc, e_xc))*(2*(e_xc^2 + e_yc^2)^(1/2) - (e_xc^2 + e_yc^2)^(3/2)/4) + sin(2*u_c - 2*atan2(e_yc, e_xc))*((5*e_xc^2)/4 + (5*e_yc^2)/4))*(e_xc^2 + e_yc^2)^(1/2) + e_xc^2 + e_yc^2 + 1)^(1/2)) - (B_c*mu*rho*sin(u_c - atan2(e_yc, e_xc) + (13*sin(3*u_c - 3*atan2(e_yc, e_xc))*(e_xc^2 + e_yc^2)^(3/2))/12 + sin(u_c - atan2(e_yc, e_xc))*(2*(e_xc^2 + e_yc^2)^(1/2) - (e_xc^2 + e_yc^2)^(3/2)/4) + sin(2*u_c - 2*atan2(e_yc, e_xc))*((5*e_xc^2)/4 + (5*e_yc^2)/4))^2*(delta_B + 1)*((e_xc^2 + e_yc^2)/(cos(u_c - atan2(e_yc, e_xc) + (13*sin(3*u_c - 3*atan2(e_yc, e_xc))*(e_xc^2 + e_yc^2)^(3/2))/12 + sin(u_c - atan2(e_yc, e_xc))*(2*(e_xc^2 + e_yc^2)^(1/2) - (e_xc^2 + e_yc^2)^(3/2)/4) + sin(2*u_c - 2*atan2(e_yc, e_xc))*((5*e_xc^2)/4 + (5*e_yc^2)/4))*(e_xc^2 + e_yc^2)^(1/2) + 1) + 1)*((13*cos(3*u_c - 3*atan2(e_yc, e_xc))*(e_xc^2 + e_yc^2)^(3/2))/4 + cos(u_c - atan2(e_yc, e_xc))*(2*(e_xc^2 + e_yc^2)^(1/2) - (e_xc^2 + e_yc^2)^(3/2)/4) + 2*cos(2*u_c - 2*atan2(e_yc, e_xc))*((5*e_xc^2)/4 + (5*e_yc^2)/4) + 1))/(a_c*(-mu/(a_c*(e_xc^2 + e_yc^2 - 1)))^(1/2)*(1 - e_yc^2 - e_xc^2)^(1/2)*(2*cos(u_c - atan2(e_yc, e_xc) + (13*sin(3*u_c - 3*atan2(e_yc, e_xc))*(e_xc^2 + e_yc^2)^(3/2))/12 + sin(u_c - atan2(e_yc, e_xc))*(2*(e_xc^2 + e_yc^2)^(1/2) - (e_xc^2 + e_yc^2)^(3/2)/4) + sin(2*u_c - 2*atan2(e_yc, e_xc))*((5*e_xc^2)/4 + (5*e_yc^2)/4))*(e_xc^2 + e_yc^2)^(1/2) + e_xc^2 + e_yc^2 + 1)^(1/2)) + (B_c*mu*rho*cos(u_c - atan2(e_yc, e_xc) + (13*sin(3*u_c - 3*atan2(e_yc, e_xc))*(e_xc^2 + e_yc^2)^(3/2))/12 + sin(u_c - atan2(e_yc, e_xc))*(2*(e_xc^2 + e_yc^2)^(1/2) - (e_xc^2 + e_yc^2)^(3/2)/4) + sin(2*u_c - 2*atan2(e_yc, e_xc))*((5*e_xc^2)/4 + (5*e_yc^2)/4))*(delta_B + 1)*(2*cos(u_c - atan2(e_yc, e_xc) + (13*sin(3*u_c - 3*atan2(e_yc, e_xc))*(e_xc^2 + e_yc^2)^(3/2))/12 + sin(u_c - atan2(e_yc, e_xc))*(2*(e_xc^2 + e_yc^2)^(1/2) - (e_xc^2 + e_yc^2)^(3/2)/4) + sin(2*u_c - 2*atan2(e_yc, e_xc))*((5*e_xc^2)/4 + (5*e_yc^2)/4))*(e_xc^2 + e_yc^2)^(1/2) + e_xc^2 + e_yc^2 + 1)^(1/2)*((13*cos(3*u_c - 3*atan2(e_yc, e_xc))*(e_xc^2 + e_yc^2)^(3/2))/4 + cos(u_c - atan2(e_yc, e_xc))*(2*(e_xc^2 + e_yc^2)^(1/2) - (e_xc^2 + e_yc^2)^(3/2)/4) + 2*cos(2*u_c - 2*atan2(e_yc, e_xc))*((5*e_xc^2)/4 + (5*e_yc^2)/4) + 1))/(a_c*(e_xc^2 + e_yc^2)^(1/2)*(-mu/(a_c*(e_xc^2 + e_yc^2 - 1)))^(1/2)*(e_xc^2 + e_yc^2 - 1)) + (B_c*mu*rho*sin(u_c - atan2(e_yc, e_xc) + (13*sin(3*u_c - 3*atan2(e_yc, e_xc))*(e_xc^2 + e_yc^2)^(3/2))/12 + sin(u_c - atan2(e_yc, e_xc))*(2*(e_xc^2 + e_yc^2)^(1/2) - (e_xc^2 + e_yc^2)^(3/2)/4) + sin(2*u_c - 2*atan2(e_yc, e_xc))*((5*e_xc^2)/4 + (5*e_yc^2)/4))^2*(e_c^2/(e_c*cos(u_c - atan2(e_yc, e_xc) + (13*sin(3*u_c - 3*atan2(e_yc, e_xc))*(e_xc^2 + e_yc^2)^(3/2))/12 + sin(u_c - atan2(e_yc, e_xc))*(2*(e_xc^2 + e_yc^2)^(1/2) - (e_xc^2 + e_yc^2)^(3/2)/4) + sin(2*u_c - 2*atan2(e_yc, e_xc))*((5*e_xc^2)/4 + (5*e_yc^2)/4)) + 1) + 1)*(delta_B + 1)*((13*cos(3*u_c - 3*atan2(e_yc, e_xc))*(e_xc^2 + e_yc^2)^(3/2))/4 + cos(u_c - atan2(e_yc, e_xc))*(2*(e_xc^2 + e_yc^2)^(1/2) - (e_xc^2 + e_yc^2)^(3/2)/4) + 2*cos(2*u_c - 2*atan2(e_yc, e_xc))*((5*e_xc^2)/4 + (5*e_yc^2)/4) + 1))/(a_c*(1 - e_c^2)^(1/2)*(-mu/(a_c*(e_c^2 - 1)))^(1/2)*(2*e_c*cos(u_c - atan2(e_yc, e_xc) + (13*sin(3*u_c - 3*atan2(e_yc, e_xc))*(e_xc^2 + e_yc^2)^(3/2))/12 + sin(u_c - atan2(e_yc, e_xc))*(2*(e_xc^2 + e_yc^2)^(1/2) - (e_xc^2 + e_yc^2)^(3/2)/4) + sin(2*u_c - 2*atan2(e_yc, e_xc))*((5*e_xc^2)/4 + (5*e_yc^2)/4)) + e_c^2 + 1)^(1/2)) - (B_c*mu*rho*cos(u_c - atan2(e_yc, e_xc) + (13*sin(3*u_c - 3*atan2(e_yc, e_xc))*(e_xc^2 + e_yc^2)^(3/2))/12 + sin(u_c - atan2(e_yc, e_xc))*(2*(e_xc^2 + e_yc^2)^(1/2) - (e_xc^2 + e_yc^2)^(3/2)/4) + sin(2*u_c - 2*atan2(e_yc, e_xc))*((5*e_xc^2)/4 + (5*e_yc^2)/4))*(delta_B + 1)*(2*e_c*cos(u_c - atan2(e_yc, e_xc) + (13*sin(3*u_c - 3*atan2(e_yc, e_xc))*(e_xc^2 + e_yc^2)^(3/2))/12 + sin(u_c - atan2(e_yc, e_xc))*(2*(e_xc^2 + e_yc^2)^(1/2) - (e_xc^2 + e_yc^2)^(3/2)/4) + sin(2*u_c - 2*atan2(e_yc, e_xc))*((5*e_xc^2)/4 + (5*e_yc^2)/4)) + e_c^2 + 1)^(1/2)*((13*cos(3*u_c - 3*atan2(e_yc, e_xc))*(e_xc^2 + e_yc^2)^(3/2))/4 + cos(u_c - atan2(e_yc, e_xc))*(2*(e_xc^2 + e_yc^2)^(1/2) - (e_xc^2 + e_yc^2)^(3/2)/4) + 2*cos(2*u_c - 2*atan2(e_yc, e_xc))*((5*e_xc^2)/4 + (5*e_yc^2)/4) + 1))/(a_c*e_c*(e_c^2 - 1)*(-mu/(a_c*(e_c^2 - 1)))^(1/2)) + (B_c*mu*rho*cos(u_c - atan2(e_yc, e_xc) + (13*sin(3*u_c - 3*atan2(e_yc, e_xc))*(e_xc^2 + e_yc^2)^(3/2))/12 + sin(u_c - atan2(e_yc, e_xc))*(2*(e_xc^2 + e_yc^2)^(1/2) - (e_xc^2 + e_yc^2)^(3/2)/4) + sin(2*u_c - 2*atan2(e_yc, e_xc))*((5*e_xc^2)/4 + (5*e_yc^2)/4))*(delta_B + 1)*((e_xc^2 + e_yc^2)/(cos(u_c - atan2(e_yc, e_xc) + (13*sin(3*u_c - 3*atan2(e_yc, e_xc))*(e_xc^2 + e_yc^2)^(3/2))/12 + sin(u_c - atan2(e_yc, e_xc))*(2*(e_xc^2 + e_yc^2)^(1/2) - (e_xc^2 + e_yc^2)^(3/2)/4) + sin(2*u_c - 2*atan2(e_yc, e_xc))*((5*e_xc^2)/4 + (5*e_yc^2)/4))*(e_xc^2 + e_yc^2)^(1/2) + 1) + 1)*(2*cos(u_c - atan2(e_yc, e_xc) + (13*sin(3*u_c - 3*atan2(e_yc, e_xc))*(e_xc^2 + e_yc^2)^(3/2))/12 + sin(u_c - atan2(e_yc, e_xc))*(2*(e_xc^2 + e_yc^2)^(1/2) - (e_xc^2 + e_yc^2)^(3/2)/4) + sin(2*u_c - 2*atan2(e_yc, e_xc))*((5*e_xc^2)/4 + (5*e_yc^2)/4))*(e_xc^2 + e_yc^2)^(1/2) + e_xc^2 + e_yc^2 + 1)^(1/2)*((13*cos(3*u_c - 3*atan2(e_yc, e_xc))*(e_xc^2 + e_yc^2)^(3/2))/4 + cos(u_c - atan2(e_yc, e_xc))*(2*(e_xc^2 + e_yc^2)^(1/2) - (e_xc^2 + e_yc^2)^(3/2)/4) + 2*cos(2*u_c - 2*atan2(e_yc, e_xc))*((5*e_xc^2)/4 + (5*e_yc^2)/4) + 1))/(a_c*(e_xc^2 + e_yc^2)^(1/2)*(-mu/(a_c*(e_xc^2 + e_yc^2 - 1)))^(1/2)*(1 - e_yc^2 - e_xc^2)^(1/2)) + (B_c*mu*rho*sin(u_c - atan2(e_yc, e_xc) + (13*sin(3*u_c - 3*atan2(e_yc, e_xc))*(e_xc^2 + e_yc^2)^(3/2))/12 + sin(u_c - atan2(e_yc, e_xc))*(2*(e_xc^2 + e_yc^2)^(1/2) - (e_xc^2 + e_yc^2)^(3/2)/4) + sin(2*u_c - 2*atan2(e_yc, e_xc))*((5*e_xc^2)/4 + (5*e_yc^2)/4))^2*(delta_B + 1)*(e_xc^2 + e_yc^2)*(2*cos(u_c - atan2(e_yc, e_xc) + (13*sin(3*u_c - 3*atan2(e_yc, e_xc))*(e_xc^2 + e_yc^2)^(3/2))/12 + sin(u_c - atan2(e_yc, e_xc))*(2*(e_xc^2 + e_yc^2)^(1/2) - (e_xc^2 + e_yc^2)^(3/2)/4) + sin(2*u_c - 2*atan2(e_yc, e_xc))*((5*e_xc^2)/4 + (5*e_yc^2)/4))*(e_xc^2 + e_yc^2)^(1/2) + e_xc^2 + e_yc^2 + 1)^(1/2)*((13*cos(3*u_c - 3*atan2(e_yc, e_xc))*(e_xc^2 + e_yc^2)^(3/2))/4 + cos(u_c - atan2(e_yc, e_xc))*(2*(e_xc^2 + e_yc^2)^(1/2) - (e_xc^2 + e_yc^2)^(3/2)/4) + 2*cos(2*u_c - 2*atan2(e_yc, e_xc))*((5*e_xc^2)/4 + (5*e_yc^2)/4) + 1))/(a_c*(cos(u_c - atan2(e_yc, e_xc) + (13*sin(3*u_c - 3*atan2(e_yc, e_xc))*(e_xc^2 + e_yc^2)^(3/2))/12 + sin(u_c - atan2(e_yc, e_xc))*(2*(e_xc^2 + e_yc^2)^(1/2) - (e_xc^2 + e_yc^2)^(3/2)/4) + sin(2*u_c - 2*atan2(e_yc, e_xc))*((5*e_xc^2)/4 + (5*e_yc^2)/4))*(e_xc^2 + e_yc^2)^(1/2) + 1)^2*(-mu/(a_c*(e_xc^2 + e_yc^2 - 1)))^(1/2)*(1 - e_yc^2 - e_xc^2)^(1/2)) - (B_c*e_c^2*mu*rho*sin(u_c - atan2(e_yc, e_xc) + (13*sin(3*u_c - 3*atan2(e_yc, e_xc))*(e_xc^2 + e_yc^2)^(3/2))/12 + sin(u_c - atan2(e_yc, e_xc))*(2*(e_xc^2 + e_yc^2)^(1/2) - (e_xc^2 + e_yc^2)^(3/2)/4) + sin(2*u_c - 2*atan2(e_yc, e_xc))*((5*e_xc^2)/4 + (5*e_yc^2)/4))^2*(delta_B + 1)*(2*e_c*cos(u_c - atan2(e_yc, e_xc) + (13*sin(3*u_c - 3*atan2(e_yc, e_xc))*(e_xc^2 + e_yc^2)^(3/2))/12 + sin(u_c - atan2(e_yc, e_xc))*(2*(e_xc^2 + e_yc^2)^(1/2) - (e_xc^2 + e_yc^2)^(3/2)/4) + sin(2*u_c - 2*atan2(e_yc, e_xc))*((5*e_xc^2)/4 + (5*e_yc^2)/4)) + e_c^2 + 1)^(1/2)*((13*cos(3*u_c - 3*atan2(e_yc, e_xc))*(e_xc^2 + e_yc^2)^(3/2))/4 + cos(u_c - atan2(e_yc, e_xc))*(2*(e_xc^2 + e_yc^2)^(1/2) - (e_xc^2 + e_yc^2)^(3/2)/4) + 2*cos(2*u_c - 2*atan2(e_yc, e_xc))*((5*e_xc^2)/4 + (5*e_yc^2)/4) + 1))/(a_c*(1 - e_c^2)^(1/2)*(e_c*cos(u_c - atan2(e_yc, e_xc) + (13*sin(3*u_c - 3*atan2(e_yc, e_xc))*(e_xc^2 + e_yc^2)^(3/2))/12 + sin(u_c - atan2(e_yc, e_xc))*(2*(e_xc^2 + e_yc^2)^(1/2) - (e_xc^2 + e_yc^2)^(3/2)/4) + sin(2*u_c - 2*atan2(e_yc, e_xc))*((5*e_xc^2)/4 + (5*e_yc^2)/4)) + 1)^2*(-mu/(a_c*(e_c^2 - 1)))^(1/2)) - (B_c*mu*rho*cos(u_c - atan2(e_yc, e_xc) + (13*sin(3*u_c - 3*atan2(e_yc, e_xc))*(e_xc^2 + e_yc^2)^(3/2))/12 + sin(u_c - atan2(e_yc, e_xc))*(2*(e_xc^2 + e_yc^2)^(1/2) - (e_xc^2 + e_yc^2)^(3/2)/4) + sin(2*u_c - 2*atan2(e_yc, e_xc))*((5*e_xc^2)/4 + (5*e_yc^2)/4))*(e_c^2/(e_c*cos(u_c - atan2(e_yc, e_xc) + (13*sin(3*u_c - 3*atan2(e_yc, e_xc))*(e_xc^2 + e_yc^2)^(3/2))/12 + sin(u_c - atan2(e_yc, e_xc))*(2*(e_xc^2 + e_yc^2)^(1/2) - (e_xc^2 + e_yc^2)^(3/2)/4) + sin(2*u_c - 2*atan2(e_yc, e_xc))*((5*e_xc^2)/4 + (5*e_yc^2)/4)) + 1) + 1)*(delta_B + 1)*(2*e_c*cos(u_c - atan2(e_yc, e_xc) + (13*sin(3*u_c - 3*atan2(e_yc, e_xc))*(e_xc^2 + e_yc^2)^(3/2))/12 + sin(u_c - atan2(e_yc, e_xc))*(2*(e_xc^2 + e_yc^2)^(1/2) - (e_xc^2 + e_yc^2)^(3/2)/4) + sin(2*u_c - 2*atan2(e_yc, e_xc))*((5*e_xc^2)/4 + (5*e_yc^2)/4)) + e_c^2 + 1)^(1/2)*((13*cos(3*u_c - 3*atan2(e_yc, e_xc))*(e_xc^2 + e_yc^2)^(3/2))/4 + cos(u_c - atan2(e_yc, e_xc))*(2*(e_xc^2 + e_yc^2)^(1/2) - (e_xc^2 + e_yc^2)^(3/2)/4) + 2*cos(2*u_c - 2*atan2(e_yc, e_xc))*((5*e_xc^2)/4 + (5*e_yc^2)/4) + 1))/(a_c*e_c*(1 - e_c^2)^(1/2)*(-mu/(a_c*(e_c^2 - 1)))^(1/2));
% A_drag(2,3) = (B_c*mu*rho*sin(u_c - atan2(e_yc, e_xc) + (13*sin(3*u_c - 3*atan2(e_yc, e_xc))*(e_xc^2 + e_yc^2)^(3/2))/12 + sin(u_c - atan2(e_yc, e_xc))*(2*(e_xc^2 + e_yc^2)^(1/2) - (e_xc^2 + e_yc^2)^(3/2)/4) + sin(2*u_c - 2*atan2(e_yc, e_xc))*((5*e_xc^2)/4 + (5*e_yc^2)/4))^2*(delta_B + 1)*(e_yc/(e_xc^2 + e_yc^2) + sin(u_c - atan2(e_yc, e_xc))*((2*e_xc)/(e_xc^2 + e_yc^2)^(1/2) - (3*e_xc*(e_xc^2 + e_yc^2)^(1/2))/4) + (5*e_xc*sin(2*u_c - 2*atan2(e_yc, e_xc)))/2 + (13*e_yc*cos(3*u_c - 3*atan2(e_yc, e_xc))*(e_xc^2 + e_yc^2)^(1/2))/4 + (13*e_xc*sin(3*u_c - 3*atan2(e_yc, e_xc))*(e_xc^2 + e_yc^2)^(1/2))/4 + (e_yc*cos(u_c - atan2(e_yc, e_xc))*(2*(e_xc^2 + e_yc^2)^(1/2) - (e_xc^2 + e_yc^2)^(3/2)/4))/(e_xc^2 + e_yc^2) + (2*e_yc*cos(2*u_c - 2*atan2(e_yc, e_xc))*((5*e_xc^2)/4 + (5*e_yc^2)/4))/(e_xc^2 + e_yc^2)))/(a_c*(e_c^2 - 1)*(-mu/(a_c*(e_c^2 - 1)))^(1/2)*(2*e_c*cos(u_c - atan2(e_yc, e_xc) + (13*sin(3*u_c - 3*atan2(e_yc, e_xc))*(e_xc^2 + e_yc^2)^(3/2))/12 + sin(u_c - atan2(e_yc, e_xc))*(2*(e_xc^2 + e_yc^2)^(1/2) - (e_xc^2 + e_yc^2)^(3/2)/4) + sin(2*u_c - 2*atan2(e_yc, e_xc))*((5*e_xc^2)/4 + (5*e_yc^2)/4)) + e_c^2 + 1)^(1/2)) - (B_c*e_xc*mu^2*rho*sin(u_c - atan2(e_yc, e_xc) + (13*sin(3*u_c - 3*atan2(e_yc, e_xc))*(e_xc^2 + e_yc^2)^(3/2))/12 + sin(u_c - atan2(e_yc, e_xc))*(2*(e_xc^2 + e_yc^2)^(1/2) - (e_xc^2 + e_yc^2)^(3/2)/4) + sin(2*u_c - 2*atan2(e_yc, e_xc))*((5*e_xc^2)/4 + (5*e_yc^2)/4))*(delta_B + 1)*(2*cos(u_c - atan2(e_yc, e_xc) + (13*sin(3*u_c - 3*atan2(e_yc, e_xc))*(e_xc^2 + e_yc^2)^(3/2))/12 + sin(u_c - atan2(e_yc, e_xc))*(2*(e_xc^2 + e_yc^2)^(1/2) - (e_xc^2 + e_yc^2)^(3/2)/4) + sin(2*u_c - 2*atan2(e_yc, e_xc))*((5*e_xc^2)/4 + (5*e_yc^2)/4))*(e_xc^2 + e_yc^2)^(1/2) + e_xc^2 + e_yc^2 + 1)^(1/2))/(a_c^2*(e_xc^2 + e_yc^2)^(1/2)*(-mu/(a_c*(e_xc^2 + e_yc^2 - 1)))^(3/2)*(e_xc^2 + e_yc^2 - 1)^3) + (B_c*mu*rho*cos(u_c - atan2(e_yc, e_xc) + (13*sin(3*u_c - 3*atan2(e_yc, e_xc))*(e_xc^2 + e_yc^2)^(3/2))/12 + sin(u_c - atan2(e_yc, e_xc))*(2*(e_xc^2 + e_yc^2)^(1/2) - (e_xc^2 + e_yc^2)^(3/2)/4) + sin(2*u_c - 2*atan2(e_yc, e_xc))*((5*e_xc^2)/4 + (5*e_yc^2)/4))*(delta_B + 1)*(2*cos(u_c - atan2(e_yc, e_xc) + (13*sin(3*u_c - 3*atan2(e_yc, e_xc))*(e_xc^2 + e_yc^2)^(3/2))/12 + sin(u_c - atan2(e_yc, e_xc))*(2*(e_xc^2 + e_yc^2)^(1/2) - (e_xc^2 + e_yc^2)^(3/2)/4) + sin(2*u_c - 2*atan2(e_yc, e_xc))*((5*e_xc^2)/4 + (5*e_yc^2)/4))*(e_xc^2 + e_yc^2)^(1/2) + e_xc^2 + e_yc^2 + 1)^(1/2)*(e_yc/(e_xc^2 + e_yc^2) + sin(u_c - atan2(e_yc, e_xc))*((2*e_xc)/(e_xc^2 + e_yc^2)^(1/2) - (3*e_xc*(e_xc^2 + e_yc^2)^(1/2))/4) + (5*e_xc*sin(2*u_c - 2*atan2(e_yc, e_xc)))/2 + (13*e_yc*cos(3*u_c - 3*atan2(e_yc, e_xc))*(e_xc^2 + e_yc^2)^(1/2))/4 + (13*e_xc*sin(3*u_c - 3*atan2(e_yc, e_xc))*(e_xc^2 + e_yc^2)^(1/2))/4 + (e_yc*cos(u_c - atan2(e_yc, e_xc))*(2*(e_xc^2 + e_yc^2)^(1/2) - (e_xc^2 + e_yc^2)^(3/2)/4))/(e_xc^2 + e_yc^2) + (2*e_yc*cos(2*u_c - 2*atan2(e_yc, e_xc))*((5*e_xc^2)/4 + (5*e_yc^2)/4))/(e_xc^2 + e_yc^2)))/(a_c*(e_xc^2 + e_yc^2)^(1/2)*(-mu/(a_c*(e_xc^2 + e_yc^2 - 1)))^(1/2)*(e_xc^2 + e_yc^2 - 1)) + (B_c*mu*rho*sin(u_c - atan2(e_yc, e_xc) + (13*sin(3*u_c - 3*atan2(e_yc, e_xc))*(e_xc^2 + e_yc^2)^(3/2))/12 + sin(u_c - atan2(e_yc, e_xc))*(2*(e_xc^2 + e_yc^2)^(1/2) - (e_xc^2 + e_yc^2)^(3/2)/4) + sin(2*u_c - 2*atan2(e_yc, e_xc))*((5*e_xc^2)/4 + (5*e_yc^2)/4))*((2*e_xc)/(cos(u_c - atan2(e_yc, e_xc) + (13*sin(3*u_c - 3*atan2(e_yc, e_xc))*(e_xc^2 + e_yc^2)^(3/2))/12 + sin(u_c - atan2(e_yc, e_xc))*(2*(e_xc^2 + e_yc^2)^(1/2) - (e_xc^2 + e_yc^2)^(3/2)/4) + sin(2*u_c - 2*atan2(e_yc, e_xc))*((5*e_xc^2)/4 + (5*e_yc^2)/4))*(e_xc^2 + e_yc^2)^(1/2) + 1) - ((e_xc^2 + e_yc^2)*((e_xc*cos(u_c - atan2(e_yc, e_xc) + (13*sin(3*u_c - 3*atan2(e_yc, e_xc))*(e_xc^2 + e_yc^2)^(3/2))/12 + sin(u_c - atan2(e_yc, e_xc))*(2*(e_xc^2 + e_yc^2)^(1/2) - (e_xc^2 + e_yc^2)^(3/2)/4) + sin(2*u_c - 2*atan2(e_yc, e_xc))*((5*e_xc^2)/4 + (5*e_yc^2)/4)))/(e_xc^2 + e_yc^2)^(1/2) - sin(u_c - atan2(e_yc, e_xc) + (13*sin(3*u_c - 3*atan2(e_yc, e_xc))*(e_xc^2 + e_yc^2)^(3/2))/12 + sin(u_c - atan2(e_yc, e_xc))*(2*(e_xc^2 + e_yc^2)^(1/2) - (e_xc^2 + e_yc^2)^(3/2)/4) + sin(2*u_c - 2*atan2(e_yc, e_xc))*((5*e_xc^2)/4 + (5*e_yc^2)/4))*(e_xc^2 + e_yc^2)^(1/2)*(e_yc/(e_xc^2 + e_yc^2) + sin(u_c - atan2(e_yc, e_xc))*((2*e_xc)/(e_xc^2 + e_yc^2)^(1/2) - (3*e_xc*(e_xc^2 + e_yc^2)^(1/2))/4) + (5*e_xc*sin(2*u_c - 2*atan2(e_yc, e_xc)))/2 + (13*e_yc*cos(3*u_c - 3*atan2(e_yc, e_xc))*(e_xc^2 + e_yc^2)^(1/2))/4 + (13*e_xc*sin(3*u_c - 3*atan2(e_yc, e_xc))*(e_xc^2 + e_yc^2)^(1/2))/4 + (e_yc*cos(u_c - atan2(e_yc, e_xc))*(2*(e_xc^2 + e_yc^2)^(1/2) - (e_xc^2 + e_yc^2)^(3/2)/4))/(e_xc^2 + e_yc^2) + (2*e_yc*cos(2*u_c - 2*atan2(e_yc, e_xc))*((5*e_xc^2)/4 + (5*e_yc^2)/4))/(e_xc^2 + e_yc^2))))/(cos(u_c - atan2(e_yc, e_xc) + (13*sin(3*u_c - 3*atan2(e_yc, e_xc))*(e_xc^2 + e_yc^2)^(3/2))/12 + sin(u_c - atan2(e_yc, e_xc))*(2*(e_xc^2 + e_yc^2)^(1/2) - (e_xc^2 + e_yc^2)^(3/2)/4) + sin(2*u_c - 2*atan2(e_yc, e_xc))*((5*e_xc^2)/4 + (5*e_yc^2)/4))*(e_xc^2 + e_yc^2)^(1/2) + 1)^2)*(delta_B + 1)*(2*cos(u_c - atan2(e_yc, e_xc) + (13*sin(3*u_c - 3*atan2(e_yc, e_xc))*(e_xc^2 + e_yc^2)^(3/2))/12 + sin(u_c - atan2(e_yc, e_xc))*(2*(e_xc^2 + e_yc^2)^(1/2) - (e_xc^2 + e_yc^2)^(3/2)/4) + sin(2*u_c - 2*atan2(e_yc, e_xc))*((5*e_xc^2)/4 + (5*e_yc^2)/4))*(e_xc^2 + e_yc^2)^(1/2) + e_xc^2 + e_yc^2 + 1)^(1/2))/(a_c*(e_xc^2 + e_yc^2)^(1/2)*(-mu/(a_c*(e_xc^2 + e_yc^2 - 1)))^(1/2)*(1 - e_yc^2 - e_xc^2)^(1/2)) + (B_c*mu*rho*sin(u_c - atan2(e_yc, e_xc) + (13*sin(3*u_c - 3*atan2(e_yc, e_xc))*(e_xc^2 + e_yc^2)^(3/2))/12 + sin(u_c - atan2(e_yc, e_xc))*(2*(e_xc^2 + e_yc^2)^(1/2) - (e_xc^2 + e_yc^2)^(3/2)/4) + sin(2*u_c - 2*atan2(e_yc, e_xc))*((5*e_xc^2)/4 + (5*e_yc^2)/4))^2*(e_c^2/(e_c*cos(u_c - atan2(e_yc, e_xc) + (13*sin(3*u_c - 3*atan2(e_yc, e_xc))*(e_xc^2 + e_yc^2)^(3/2))/12 + sin(u_c - atan2(e_yc, e_xc))*(2*(e_xc^2 + e_yc^2)^(1/2) - (e_xc^2 + e_yc^2)^(3/2)/4) + sin(2*u_c - 2*atan2(e_yc, e_xc))*((5*e_xc^2)/4 + (5*e_yc^2)/4)) + 1) + 1)*(delta_B + 1)*(e_yc/(e_xc^2 + e_yc^2) + sin(u_c - atan2(e_yc, e_xc))*((2*e_xc)/(e_xc^2 + e_yc^2)^(1/2) - (3*e_xc*(e_xc^2 + e_yc^2)^(1/2))/4) + (5*e_xc*sin(2*u_c - 2*atan2(e_yc, e_xc)))/2 + (13*e_yc*cos(3*u_c - 3*atan2(e_yc, e_xc))*(e_xc^2 + e_yc^2)^(1/2))/4 + (13*e_xc*sin(3*u_c - 3*atan2(e_yc, e_xc))*(e_xc^2 + e_yc^2)^(1/2))/4 + (e_yc*cos(u_c - atan2(e_yc, e_xc))*(2*(e_xc^2 + e_yc^2)^(1/2) - (e_xc^2 + e_yc^2)^(3/2)/4))/(e_xc^2 + e_yc^2) + (2*e_yc*cos(2*u_c - 2*atan2(e_yc, e_xc))*((5*e_xc^2)/4 + (5*e_yc^2)/4))/(e_xc^2 + e_yc^2)))/(a_c*(1 - e_c^2)^(1/2)*(-mu/(a_c*(e_c^2 - 1)))^(1/2)*(2*e_c*cos(u_c - atan2(e_yc, e_xc) + (13*sin(3*u_c - 3*atan2(e_yc, e_xc))*(e_xc^2 + e_yc^2)^(3/2))/12 + sin(u_c - atan2(e_yc, e_xc))*(2*(e_xc^2 + e_yc^2)^(1/2) - (e_xc^2 + e_yc^2)^(3/2)/4) + sin(2*u_c - 2*atan2(e_yc, e_xc))*((5*e_xc^2)/4 + (5*e_yc^2)/4)) + e_c^2 + 1)^(1/2)) - (2*B_c*e_xc*mu*rho*sin(u_c - atan2(e_yc, e_xc) + (13*sin(3*u_c - 3*atan2(e_yc, e_xc))*(e_xc^2 + e_yc^2)^(3/2))/12 + sin(u_c - atan2(e_yc, e_xc))*(2*(e_xc^2 + e_yc^2)^(1/2) - (e_xc^2 + e_yc^2)^(3/2)/4) + sin(2*u_c - 2*atan2(e_yc, e_xc))*((5*e_xc^2)/4 + (5*e_yc^2)/4))*(delta_B + 1)*(2*cos(u_c - atan2(e_yc, e_xc) + (13*sin(3*u_c - 3*atan2(e_yc, e_xc))*(e_xc^2 + e_yc^2)^(3/2))/12 + sin(u_c - atan2(e_yc, e_xc))*(2*(e_xc^2 + e_yc^2)^(1/2) - (e_xc^2 + e_yc^2)^(3/2)/4) + sin(2*u_c - 2*atan2(e_yc, e_xc))*((5*e_xc^2)/4 + (5*e_yc^2)/4))*(e_xc^2 + e_yc^2)^(1/2) + e_xc^2 + e_yc^2 + 1)^(1/2))/(a_c*(e_xc^2 + e_yc^2)^(1/2)*(-mu/(a_c*(e_xc^2 + e_yc^2 - 1)))^(1/2)*(e_xc^2 + e_yc^2 - 1)^2) - (B_c*e_xc*mu*rho*sin(u_c - atan2(e_yc, e_xc) + (13*sin(3*u_c - 3*atan2(e_yc, e_xc))*(e_xc^2 + e_yc^2)^(3/2))/12 + sin(u_c - atan2(e_yc, e_xc))*(2*(e_xc^2 + e_yc^2)^(1/2) - (e_xc^2 + e_yc^2)^(3/2)/4) + sin(2*u_c - 2*atan2(e_yc, e_xc))*((5*e_xc^2)/4 + (5*e_yc^2)/4))*(delta_B + 1)*(2*cos(u_c - atan2(e_yc, e_xc) + (13*sin(3*u_c - 3*atan2(e_yc, e_xc))*(e_xc^2 + e_yc^2)^(3/2))/12 + sin(u_c - atan2(e_yc, e_xc))*(2*(e_xc^2 + e_yc^2)^(1/2) - (e_xc^2 + e_yc^2)^(3/2)/4) + sin(2*u_c - 2*atan2(e_yc, e_xc))*((5*e_xc^2)/4 + (5*e_yc^2)/4))*(e_xc^2 + e_yc^2)^(1/2) + e_xc^2 + e_yc^2 + 1)^(1/2))/(a_c*(e_xc^2 + e_yc^2)^(3/2)*(-mu/(a_c*(e_xc^2 + e_yc^2 - 1)))^(1/2)*(e_xc^2 + e_yc^2 - 1)) - (B_c*mu*rho*cos(u_c - atan2(e_yc, e_xc) + (13*sin(3*u_c - 3*atan2(e_yc, e_xc))*(e_xc^2 + e_yc^2)^(3/2))/12 + sin(u_c - atan2(e_yc, e_xc))*(2*(e_xc^2 + e_yc^2)^(1/2) - (e_xc^2 + e_yc^2)^(3/2)/4) + sin(2*u_c - 2*atan2(e_yc, e_xc))*((5*e_xc^2)/4 + (5*e_yc^2)/4))*(delta_B + 1)*(2*e_c*cos(u_c - atan2(e_yc, e_xc) + (13*sin(3*u_c - 3*atan2(e_yc, e_xc))*(e_xc^2 + e_yc^2)^(3/2))/12 + sin(u_c - atan2(e_yc, e_xc))*(2*(e_xc^2 + e_yc^2)^(1/2) - (e_xc^2 + e_yc^2)^(3/2)/4) + sin(2*u_c - 2*atan2(e_yc, e_xc))*((5*e_xc^2)/4 + (5*e_yc^2)/4)) + e_c^2 + 1)^(1/2)*(e_yc/(e_xc^2 + e_yc^2) + sin(u_c - atan2(e_yc, e_xc))*((2*e_xc)/(e_xc^2 + e_yc^2)^(1/2) - (3*e_xc*(e_xc^2 + e_yc^2)^(1/2))/4) + (5*e_xc*sin(2*u_c - 2*atan2(e_yc, e_xc)))/2 + (13*e_yc*cos(3*u_c - 3*atan2(e_yc, e_xc))*(e_xc^2 + e_yc^2)^(1/2))/4 + (13*e_xc*sin(3*u_c - 3*atan2(e_yc, e_xc))*(e_xc^2 + e_yc^2)^(1/2))/4 + (e_yc*cos(u_c - atan2(e_yc, e_xc))*(2*(e_xc^2 + e_yc^2)^(1/2) - (e_xc^2 + e_yc^2)^(3/2)/4))/(e_xc^2 + e_yc^2) + (2*e_yc*cos(2*u_c - 2*atan2(e_yc, e_xc))*((5*e_xc^2)/4 + (5*e_yc^2)/4))/(e_xc^2 + e_yc^2)))/(a_c*e_c*(e_c^2 - 1)*(-mu/(a_c*(e_c^2 - 1)))^(1/2)) + (B_c*mu*rho*sin(u_c - atan2(e_yc, e_xc) + (13*sin(3*u_c - 3*atan2(e_yc, e_xc))*(e_xc^2 + e_yc^2)^(3/2))/12 + sin(u_c - atan2(e_yc, e_xc))*(2*(e_xc^2 + e_yc^2)^(1/2) - (e_xc^2 + e_yc^2)^(3/2)/4) + sin(2*u_c - 2*atan2(e_yc, e_xc))*((5*e_xc^2)/4 + (5*e_yc^2)/4))*(delta_B + 1)*(2*e_xc + (2*e_xc*cos(u_c - atan2(e_yc, e_xc) + (13*sin(3*u_c - 3*atan2(e_yc, e_xc))*(e_xc^2 + e_yc^2)^(3/2))/12 + sin(u_c - atan2(e_yc, e_xc))*(2*(e_xc^2 + e_yc^2)^(1/2) - (e_xc^2 + e_yc^2)^(3/2)/4) + sin(2*u_c - 2*atan2(e_yc, e_xc))*((5*e_xc^2)/4 + (5*e_yc^2)/4)))/(e_xc^2 + e_yc^2)^(1/2) - 2*sin(u_c - atan2(e_yc, e_xc) + (13*sin(3*u_c - 3*atan2(e_yc, e_xc))*(e_xc^2 + e_yc^2)^(3/2))/12 + sin(u_c - atan2(e_yc, e_xc))*(2*(e_xc^2 + e_yc^2)^(1/2) - (e_xc^2 + e_yc^2)^(3/2)/4) + sin(2*u_c - 2*atan2(e_yc, e_xc))*((5*e_xc^2)/4 + (5*e_yc^2)/4))*(e_xc^2 + e_yc^2)^(1/2)*(e_yc/(e_xc^2 + e_yc^2) + sin(u_c - atan2(e_yc, e_xc))*((2*e_xc)/(e_xc^2 + e_yc^2)^(1/2) - (3*e_xc*(e_xc^2 + e_yc^2)^(1/2))/4) + (5*e_xc*sin(2*u_c - 2*atan2(e_yc, e_xc)))/2 + (13*e_yc*cos(3*u_c - 3*atan2(e_yc, e_xc))*(e_xc^2 + e_yc^2)^(1/2))/4 + (13*e_xc*sin(3*u_c - 3*atan2(e_yc, e_xc))*(e_xc^2 + e_yc^2)^(1/2))/4 + (e_yc*cos(u_c - atan2(e_yc, e_xc))*(2*(e_xc^2 + e_yc^2)^(1/2) - (e_xc^2 + e_yc^2)^(3/2)/4))/(e_xc^2 + e_yc^2) + (2*e_yc*cos(2*u_c - 2*atan2(e_yc, e_xc))*((5*e_xc^2)/4 + (5*e_yc^2)/4))/(e_xc^2 + e_yc^2))))/(2*a_c*(e_xc^2 + e_yc^2)^(1/2)*(-mu/(a_c*(e_xc^2 + e_yc^2 - 1)))^(1/2)*(e_xc^2 + e_yc^2 - 1)*(2*cos(u_c - atan2(e_yc, e_xc) + (13*sin(3*u_c - 3*atan2(e_yc, e_xc))*(e_xc^2 + e_yc^2)^(3/2))/12 + sin(u_c - atan2(e_yc, e_xc))*(2*(e_xc^2 + e_yc^2)^(1/2) - (e_xc^2 + e_yc^2)^(3/2)/4) + sin(2*u_c - 2*atan2(e_yc, e_xc))*((5*e_xc^2)/4 + (5*e_yc^2)/4))*(e_xc^2 + e_yc^2)^(1/2) + e_xc^2 + e_yc^2 + 1)^(1/2)) + (B_c*mu*rho*cos(u_c - atan2(e_yc, e_xc) + (13*sin(3*u_c - 3*atan2(e_yc, e_xc))*(e_xc^2 + e_yc^2)^(3/2))/12 + sin(u_c - atan2(e_yc, e_xc))*(2*(e_xc^2 + e_yc^2)^(1/2) - (e_xc^2 + e_yc^2)^(3/2)/4) + sin(2*u_c - 2*atan2(e_yc, e_xc))*((5*e_xc^2)/4 + (5*e_yc^2)/4))*(delta_B + 1)*((e_xc^2 + e_yc^2)/(cos(u_c - atan2(e_yc, e_xc) + (13*sin(3*u_c - 3*atan2(e_yc, e_xc))*(e_xc^2 + e_yc^2)^(3/2))/12 + sin(u_c - atan2(e_yc, e_xc))*(2*(e_xc^2 + e_yc^2)^(1/2) - (e_xc^2 + e_yc^2)^(3/2)/4) + sin(2*u_c - 2*atan2(e_yc, e_xc))*((5*e_xc^2)/4 + (5*e_yc^2)/4))*(e_xc^2 + e_yc^2)^(1/2) + 1) + 1)*(2*cos(u_c - atan2(e_yc, e_xc) + (13*sin(3*u_c - 3*atan2(e_yc, e_xc))*(e_xc^2 + e_yc^2)^(3/2))/12 + sin(u_c - atan2(e_yc, e_xc))*(2*(e_xc^2 + e_yc^2)^(1/2) - (e_xc^2 + e_yc^2)^(3/2)/4) + sin(2*u_c - 2*atan2(e_yc, e_xc))*((5*e_xc^2)/4 + (5*e_yc^2)/4))*(e_xc^2 + e_yc^2)^(1/2) + e_xc^2 + e_yc^2 + 1)^(1/2)*(e_yc/(e_xc^2 + e_yc^2) + sin(u_c - atan2(e_yc, e_xc))*((2*e_xc)/(e_xc^2 + e_yc^2)^(1/2) - (3*e_xc*(e_xc^2 + e_yc^2)^(1/2))/4) + (5*e_xc*sin(2*u_c - 2*atan2(e_yc, e_xc)))/2 + (13*e_yc*cos(3*u_c - 3*atan2(e_yc, e_xc))*(e_xc^2 + e_yc^2)^(1/2))/4 + (13*e_xc*sin(3*u_c - 3*atan2(e_yc, e_xc))*(e_xc^2 + e_yc^2)^(1/2))/4 + (e_yc*cos(u_c - atan2(e_yc, e_xc))*(2*(e_xc^2 + e_yc^2)^(1/2) - (e_xc^2 + e_yc^2)^(3/2)/4))/(e_xc^2 + e_yc^2) + (2*e_yc*cos(2*u_c - 2*atan2(e_yc, e_xc))*((5*e_xc^2)/4 + (5*e_yc^2)/4))/(e_xc^2 + e_yc^2)))/(a_c*(e_xc^2 + e_yc^2)^(1/2)*(-mu/(a_c*(e_xc^2 + e_yc^2 - 1)))^(1/2)*(1 - e_yc^2 - e_xc^2)^(1/2)) + (B_c*e_xc*mu*rho*sin(u_c - atan2(e_yc, e_xc) + (13*sin(3*u_c - 3*atan2(e_yc, e_xc))*(e_xc^2 + e_yc^2)^(3/2))/12 + sin(u_c - atan2(e_yc, e_xc))*(2*(e_xc^2 + e_yc^2)^(1/2) - (e_xc^2 + e_yc^2)^(3/2)/4) + sin(2*u_c - 2*atan2(e_yc, e_xc))*((5*e_xc^2)/4 + (5*e_yc^2)/4))*(delta_B + 1)*((e_xc^2 + e_yc^2)/(cos(u_c - atan2(e_yc, e_xc) + (13*sin(3*u_c - 3*atan2(e_yc, e_xc))*(e_xc^2 + e_yc^2)^(3/2))/12 + sin(u_c - atan2(e_yc, e_xc))*(2*(e_xc^2 + e_yc^2)^(1/2) - (e_xc^2 + e_yc^2)^(3/2)/4) + sin(2*u_c - 2*atan2(e_yc, e_xc))*((5*e_xc^2)/4 + (5*e_yc^2)/4))*(e_xc^2 + e_yc^2)^(1/2) + 1) + 1)*(2*cos(u_c - atan2(e_yc, e_xc) + (13*sin(3*u_c - 3*atan2(e_yc, e_xc))*(e_xc^2 + e_yc^2)^(3/2))/12 + sin(u_c - atan2(e_yc, e_xc))*(2*(e_xc^2 + e_yc^2)^(1/2) - (e_xc^2 + e_yc^2)^(3/2)/4) + sin(2*u_c - 2*atan2(e_yc, e_xc))*((5*e_xc^2)/4 + (5*e_yc^2)/4))*(e_xc^2 + e_yc^2)^(1/2) + e_xc^2 + e_yc^2 + 1)^(1/2))/(a_c*(e_xc^2 + e_yc^2)^(1/2)*(-mu/(a_c*(e_xc^2 + e_yc^2 - 1)))^(1/2)*(1 - e_yc^2 - e_xc^2)^(3/2)) - (B_c*e_xc*mu*rho*sin(u_c - atan2(e_yc, e_xc) + (13*sin(3*u_c - 3*atan2(e_yc, e_xc))*(e_xc^2 + e_yc^2)^(3/2))/12 + sin(u_c - atan2(e_yc, e_xc))*(2*(e_xc^2 + e_yc^2)^(1/2) - (e_xc^2 + e_yc^2)^(3/2)/4) + sin(2*u_c - 2*atan2(e_yc, e_xc))*((5*e_xc^2)/4 + (5*e_yc^2)/4))*(delta_B + 1)*((e_xc^2 + e_yc^2)/(cos(u_c - atan2(e_yc, e_xc) + (13*sin(3*u_c - 3*atan2(e_yc, e_xc))*(e_xc^2 + e_yc^2)^(3/2))/12 + sin(u_c - atan2(e_yc, e_xc))*(2*(e_xc^2 + e_yc^2)^(1/2) - (e_xc^2 + e_yc^2)^(3/2)/4) + sin(2*u_c - 2*atan2(e_yc, e_xc))*((5*e_xc^2)/4 + (5*e_yc^2)/4))*(e_xc^2 + e_yc^2)^(1/2) + 1) + 1)*(2*cos(u_c - atan2(e_yc, e_xc) + (13*sin(3*u_c - 3*atan2(e_yc, e_xc))*(e_xc^2 + e_yc^2)^(3/2))/12 + sin(u_c - atan2(e_yc, e_xc))*(2*(e_xc^2 + e_yc^2)^(1/2) - (e_xc^2 + e_yc^2)^(3/2)/4) + sin(2*u_c - 2*atan2(e_yc, e_xc))*((5*e_xc^2)/4 + (5*e_yc^2)/4))*(e_xc^2 + e_yc^2)^(1/2) + e_xc^2 + e_yc^2 + 1)^(1/2))/(a_c*(e_xc^2 + e_yc^2)^(3/2)*(-mu/(a_c*(e_xc^2 + e_yc^2 - 1)))^(1/2)*(1 - e_yc^2 - e_xc^2)^(1/2)) + (B_c*mu*rho*sin(u_c - atan2(e_yc, e_xc) + (13*sin(3*u_c - 3*atan2(e_yc, e_xc))*(e_xc^2 + e_yc^2)^(3/2))/12 + sin(u_c - atan2(e_yc, e_xc))*(2*(e_xc^2 + e_yc^2)^(1/2) - (e_xc^2 + e_yc^2)^(3/2)/4) + sin(2*u_c - 2*atan2(e_yc, e_xc))*((5*e_xc^2)/4 + (5*e_yc^2)/4))*(delta_B + 1)*((e_xc^2 + e_yc^2)/(cos(u_c - atan2(e_yc, e_xc) + (13*sin(3*u_c - 3*atan2(e_yc, e_xc))*(e_xc^2 + e_yc^2)^(3/2))/12 + sin(u_c - atan2(e_yc, e_xc))*(2*(e_xc^2 + e_yc^2)^(1/2) - (e_xc^2 + e_yc^2)^(3/2)/4) + sin(2*u_c - 2*atan2(e_yc, e_xc))*((5*e_xc^2)/4 + (5*e_yc^2)/4))*(e_xc^2 + e_yc^2)^(1/2) + 1) + 1)*(2*e_xc + (2*e_xc*cos(u_c - atan2(e_yc, e_xc) + (13*sin(3*u_c - 3*atan2(e_yc, e_xc))*(e_xc^2 + e_yc^2)^(3/2))/12 + sin(u_c - atan2(e_yc, e_xc))*(2*(e_xc^2 + e_yc^2)^(1/2) - (e_xc^2 + e_yc^2)^(3/2)/4) + sin(2*u_c - 2*atan2(e_yc, e_xc))*((5*e_xc^2)/4 + (5*e_yc^2)/4)))/(e_xc^2 + e_yc^2)^(1/2) - 2*sin(u_c - atan2(e_yc, e_xc) + (13*sin(3*u_c - 3*atan2(e_yc, e_xc))*(e_xc^2 + e_yc^2)^(3/2))/12 + sin(u_c - atan2(e_yc, e_xc))*(2*(e_xc^2 + e_yc^2)^(1/2) - (e_xc^2 + e_yc^2)^(3/2)/4) + sin(2*u_c - 2*atan2(e_yc, e_xc))*((5*e_xc^2)/4 + (5*e_yc^2)/4))*(e_xc^2 + e_yc^2)^(1/2)*(e_yc/(e_xc^2 + e_yc^2) + sin(u_c - atan2(e_yc, e_xc))*((2*e_xc)/(e_xc^2 + e_yc^2)^(1/2) - (3*e_xc*(e_xc^2 + e_yc^2)^(1/2))/4) + (5*e_xc*sin(2*u_c - 2*atan2(e_yc, e_xc)))/2 + (13*e_yc*cos(3*u_c - 3*atan2(e_yc, e_xc))*(e_xc^2 + e_yc^2)^(1/2))/4 + (13*e_xc*sin(3*u_c - 3*atan2(e_yc, e_xc))*(e_xc^2 + e_yc^2)^(1/2))/4 + (e_yc*cos(u_c - atan2(e_yc, e_xc))*(2*(e_xc^2 + e_yc^2)^(1/2) - (e_xc^2 + e_yc^2)^(3/2)/4))/(e_xc^2 + e_yc^2) + (2*e_yc*cos(2*u_c - 2*atan2(e_yc, e_xc))*((5*e_xc^2)/4 + (5*e_yc^2)/4))/(e_xc^2 + e_yc^2))))/(2*a_c*(e_xc^2 + e_yc^2)^(1/2)*(-mu/(a_c*(e_xc^2 + e_yc^2 - 1)))^(1/2)*(1 - e_yc^2 - e_xc^2)^(1/2)*(2*cos(u_c - atan2(e_yc, e_xc) + (13*sin(3*u_c - 3*atan2(e_yc, e_xc))*(e_xc^2 + e_yc^2)^(3/2))/12 + sin(u_c - atan2(e_yc, e_xc))*(2*(e_xc^2 + e_yc^2)^(1/2) - (e_xc^2 + e_yc^2)^(3/2)/4) + sin(2*u_c - 2*atan2(e_yc, e_xc))*((5*e_xc^2)/4 + (5*e_yc^2)/4))*(e_xc^2 + e_yc^2)^(1/2) + e_xc^2 + e_yc^2 + 1)^(1/2)) - (B_c*e_xc*mu^2*rho*sin(u_c - atan2(e_yc, e_xc) + (13*sin(3*u_c - 3*atan2(e_yc, e_xc))*(e_xc^2 + e_yc^2)^(3/2))/12 + sin(u_c - atan2(e_yc, e_xc))*(2*(e_xc^2 + e_yc^2)^(1/2) - (e_xc^2 + e_yc^2)^(3/2)/4) + sin(2*u_c - 2*atan2(e_yc, e_xc))*((5*e_xc^2)/4 + (5*e_yc^2)/4))*(delta_B + 1)*((e_xc^2 + e_yc^2)/(cos(u_c - atan2(e_yc, e_xc) + (13*sin(3*u_c - 3*atan2(e_yc, e_xc))*(e_xc^2 + e_yc^2)^(3/2))/12 + sin(u_c - atan2(e_yc, e_xc))*(2*(e_xc^2 + e_yc^2)^(1/2) - (e_xc^2 + e_yc^2)^(3/2)/4) + sin(2*u_c - 2*atan2(e_yc, e_xc))*((5*e_xc^2)/4 + (5*e_yc^2)/4))*(e_xc^2 + e_yc^2)^(1/2) + 1) + 1)*(2*cos(u_c - atan2(e_yc, e_xc) + (13*sin(3*u_c - 3*atan2(e_yc, e_xc))*(e_xc^2 + e_yc^2)^(3/2))/12 + sin(u_c - atan2(e_yc, e_xc))*(2*(e_xc^2 + e_yc^2)^(1/2) - (e_xc^2 + e_yc^2)^(3/2)/4) + sin(2*u_c - 2*atan2(e_yc, e_xc))*((5*e_xc^2)/4 + (5*e_yc^2)/4))*(e_xc^2 + e_yc^2)^(1/2) + e_xc^2 + e_yc^2 + 1)^(1/2))/(a_c^2*(e_xc^2 + e_yc^2)^(1/2)*(-mu/(a_c*(e_xc^2 + e_yc^2 - 1)))^(3/2)*(1 - e_yc^2 - e_xc^2)^(5/2)) - (B_c*e_c^2*mu*rho*sin(u_c - atan2(e_yc, e_xc) + (13*sin(3*u_c - 3*atan2(e_yc, e_xc))*(e_xc^2 + e_yc^2)^(3/2))/12 + sin(u_c - atan2(e_yc, e_xc))*(2*(e_xc^2 + e_yc^2)^(1/2) - (e_xc^2 + e_yc^2)^(3/2)/4) + sin(2*u_c - 2*atan2(e_yc, e_xc))*((5*e_xc^2)/4 + (5*e_yc^2)/4))^2*(delta_B + 1)*(2*e_c*cos(u_c - atan2(e_yc, e_xc) + (13*sin(3*u_c - 3*atan2(e_yc, e_xc))*(e_xc^2 + e_yc^2)^(3/2))/12 + sin(u_c - atan2(e_yc, e_xc))*(2*(e_xc^2 + e_yc^2)^(1/2) - (e_xc^2 + e_yc^2)^(3/2)/4) + sin(2*u_c - 2*atan2(e_yc, e_xc))*((5*e_xc^2)/4 + (5*e_yc^2)/4)) + e_c^2 + 1)^(1/2)*(e_yc/(e_xc^2 + e_yc^2) + sin(u_c - atan2(e_yc, e_xc))*((2*e_xc)/(e_xc^2 + e_yc^2)^(1/2) - (3*e_xc*(e_xc^2 + e_yc^2)^(1/2))/4) + (5*e_xc*sin(2*u_c - 2*atan2(e_yc, e_xc)))/2 + (13*e_yc*cos(3*u_c - 3*atan2(e_yc, e_xc))*(e_xc^2 + e_yc^2)^(1/2))/4 + (13*e_xc*sin(3*u_c - 3*atan2(e_yc, e_xc))*(e_xc^2 + e_yc^2)^(1/2))/4 + (e_yc*cos(u_c - atan2(e_yc, e_xc))*(2*(e_xc^2 + e_yc^2)^(1/2) - (e_xc^2 + e_yc^2)^(3/2)/4))/(e_xc^2 + e_yc^2) + (2*e_yc*cos(2*u_c - 2*atan2(e_yc, e_xc))*((5*e_xc^2)/4 + (5*e_yc^2)/4))/(e_xc^2 + e_yc^2)))/(a_c*(1 - e_c^2)^(1/2)*(e_c*cos(u_c - atan2(e_yc, e_xc) + (13*sin(3*u_c - 3*atan2(e_yc, e_xc))*(e_xc^2 + e_yc^2)^(3/2))/12 + sin(u_c - atan2(e_yc, e_xc))*(2*(e_xc^2 + e_yc^2)^(1/2) - (e_xc^2 + e_yc^2)^(3/2)/4) + sin(2*u_c - 2*atan2(e_yc, e_xc))*((5*e_xc^2)/4 + (5*e_yc^2)/4)) + 1)^2*(-mu/(a_c*(e_c^2 - 1)))^(1/2)) - (B_c*mu*rho*cos(u_c - atan2(e_yc, e_xc) + (13*sin(3*u_c - 3*atan2(e_yc, e_xc))*(e_xc^2 + e_yc^2)^(3/2))/12 + sin(u_c - atan2(e_yc, e_xc))*(2*(e_xc^2 + e_yc^2)^(1/2) - (e_xc^2 + e_yc^2)^(3/2)/4) + sin(2*u_c - 2*atan2(e_yc, e_xc))*((5*e_xc^2)/4 + (5*e_yc^2)/4))*(e_c^2/(e_c*cos(u_c - atan2(e_yc, e_xc) + (13*sin(3*u_c - 3*atan2(e_yc, e_xc))*(e_xc^2 + e_yc^2)^(3/2))/12 + sin(u_c - atan2(e_yc, e_xc))*(2*(e_xc^2 + e_yc^2)^(1/2) - (e_xc^2 + e_yc^2)^(3/2)/4) + sin(2*u_c - 2*atan2(e_yc, e_xc))*((5*e_xc^2)/4 + (5*e_yc^2)/4)) + 1) + 1)*(delta_B + 1)*(2*e_c*cos(u_c - atan2(e_yc, e_xc) + (13*sin(3*u_c - 3*atan2(e_yc, e_xc))*(e_xc^2 + e_yc^2)^(3/2))/12 + sin(u_c - atan2(e_yc, e_xc))*(2*(e_xc^2 + e_yc^2)^(1/2) - (e_xc^2 + e_yc^2)^(3/2)/4) + sin(2*u_c - 2*atan2(e_yc, e_xc))*((5*e_xc^2)/4 + (5*e_yc^2)/4)) + e_c^2 + 1)^(1/2)*(e_yc/(e_xc^2 + e_yc^2) + sin(u_c - atan2(e_yc, e_xc))*((2*e_xc)/(e_xc^2 + e_yc^2)^(1/2) - (3*e_xc*(e_xc^2 + e_yc^2)^(1/2))/4) + (5*e_xc*sin(2*u_c - 2*atan2(e_yc, e_xc)))/2 + (13*e_yc*cos(3*u_c - 3*atan2(e_yc, e_xc))*(e_xc^2 + e_yc^2)^(1/2))/4 + (13*e_xc*sin(3*u_c - 3*atan2(e_yc, e_xc))*(e_xc^2 + e_yc^2)^(1/2))/4 + (e_yc*cos(u_c - atan2(e_yc, e_xc))*(2*(e_xc^2 + e_yc^2)^(1/2) - (e_xc^2 + e_yc^2)^(3/2)/4))/(e_xc^2 + e_yc^2) + (2*e_yc*cos(2*u_c - 2*atan2(e_yc, e_xc))*((5*e_xc^2)/4 + (5*e_yc^2)/4))/(e_xc^2 + e_yc^2)))/(a_c*e_c*(1 - e_c^2)^(1/2)*(-mu/(a_c*(e_c^2 - 1)))^(1/2));
% A_drag(2,4) = (B_c*mu*rho*sin(u_c - atan2(e_yc, e_xc) + (13*sin(3*u_c - 3*atan2(e_yc, e_xc))*(e_xc^2 + e_yc^2)^(3/2))/12 + sin(u_c - atan2(e_yc, e_xc))*(2*(e_xc^2 + e_yc^2)^(1/2) - (e_xc^2 + e_yc^2)^(3/2)/4) + sin(2*u_c - 2*atan2(e_yc, e_xc))*((5*e_xc^2)/4 + (5*e_yc^2)/4))*((2*e_yc)/(cos(u_c - atan2(e_yc, e_xc) + (13*sin(3*u_c - 3*atan2(e_yc, e_xc))*(e_xc^2 + e_yc^2)^(3/2))/12 + sin(u_c - atan2(e_yc, e_xc))*(2*(e_xc^2 + e_yc^2)^(1/2) - (e_xc^2 + e_yc^2)^(3/2)/4) + sin(2*u_c - 2*atan2(e_yc, e_xc))*((5*e_xc^2)/4 + (5*e_yc^2)/4))*(e_xc^2 + e_yc^2)^(1/2) + 1) - ((e_xc^2 + e_yc^2)*((e_yc*cos(u_c - atan2(e_yc, e_xc) + (13*sin(3*u_c - 3*atan2(e_yc, e_xc))*(e_xc^2 + e_yc^2)^(3/2))/12 + sin(u_c - atan2(e_yc, e_xc))*(2*(e_xc^2 + e_yc^2)^(1/2) - (e_xc^2 + e_yc^2)^(3/2)/4) + sin(2*u_c - 2*atan2(e_yc, e_xc))*((5*e_xc^2)/4 + (5*e_yc^2)/4)))/(e_xc^2 + e_yc^2)^(1/2) + sin(u_c - atan2(e_yc, e_xc) + (13*sin(3*u_c - 3*atan2(e_yc, e_xc))*(e_xc^2 + e_yc^2)^(3/2))/12 + sin(u_c - atan2(e_yc, e_xc))*(2*(e_xc^2 + e_yc^2)^(1/2) - (e_xc^2 + e_yc^2)^(3/2)/4) + sin(2*u_c - 2*atan2(e_yc, e_xc))*((5*e_xc^2)/4 + (5*e_yc^2)/4))*(e_xc^2 + e_yc^2)^(1/2)*(e_xc/(e_xc^2 + e_yc^2) - sin(u_c - atan2(e_yc, e_xc))*((2*e_yc)/(e_xc^2 + e_yc^2)^(1/2) - (3*e_yc*(e_xc^2 + e_yc^2)^(1/2))/4) - (5*e_yc*sin(2*u_c - 2*atan2(e_yc, e_xc)))/2 + (13*e_xc*cos(3*u_c - 3*atan2(e_yc, e_xc))*(e_xc^2 + e_yc^2)^(1/2))/4 - (13*e_yc*sin(3*u_c - 3*atan2(e_yc, e_xc))*(e_xc^2 + e_yc^2)^(1/2))/4 + (e_xc*cos(u_c - atan2(e_yc, e_xc))*(2*(e_xc^2 + e_yc^2)^(1/2) - (e_xc^2 + e_yc^2)^(3/2)/4))/(e_xc^2 + e_yc^2) + (2*e_xc*cos(2*u_c - 2*atan2(e_yc, e_xc))*((5*e_xc^2)/4 + (5*e_yc^2)/4))/(e_xc^2 + e_yc^2))))/(cos(u_c - atan2(e_yc, e_xc) + (13*sin(3*u_c - 3*atan2(e_yc, e_xc))*(e_xc^2 + e_yc^2)^(3/2))/12 + sin(u_c - atan2(e_yc, e_xc))*(2*(e_xc^2 + e_yc^2)^(1/2) - (e_xc^2 + e_yc^2)^(3/2)/4) + sin(2*u_c - 2*atan2(e_yc, e_xc))*((5*e_xc^2)/4 + (5*e_yc^2)/4))*(e_xc^2 + e_yc^2)^(1/2) + 1)^2)*(delta_B + 1)*(2*cos(u_c - atan2(e_yc, e_xc) + (13*sin(3*u_c - 3*atan2(e_yc, e_xc))*(e_xc^2 + e_yc^2)^(3/2))/12 + sin(u_c - atan2(e_yc, e_xc))*(2*(e_xc^2 + e_yc^2)^(1/2) - (e_xc^2 + e_yc^2)^(3/2)/4) + sin(2*u_c - 2*atan2(e_yc, e_xc))*((5*e_xc^2)/4 + (5*e_yc^2)/4))*(e_xc^2 + e_yc^2)^(1/2) + e_xc^2 + e_yc^2 + 1)^(1/2))/(a_c*(e_xc^2 + e_yc^2)^(1/2)*(-mu/(a_c*(e_xc^2 + e_yc^2 - 1)))^(1/2)*(1 - e_yc^2 - e_xc^2)^(1/2)) - (B_c*e_yc*mu^2*rho*sin(u_c - atan2(e_yc, e_xc) + (13*sin(3*u_c - 3*atan2(e_yc, e_xc))*(e_xc^2 + e_yc^2)^(3/2))/12 + sin(u_c - atan2(e_yc, e_xc))*(2*(e_xc^2 + e_yc^2)^(1/2) - (e_xc^2 + e_yc^2)^(3/2)/4) + sin(2*u_c - 2*atan2(e_yc, e_xc))*((5*e_xc^2)/4 + (5*e_yc^2)/4))*(delta_B + 1)*(2*cos(u_c - atan2(e_yc, e_xc) + (13*sin(3*u_c - 3*atan2(e_yc, e_xc))*(e_xc^2 + e_yc^2)^(3/2))/12 + sin(u_c - atan2(e_yc, e_xc))*(2*(e_xc^2 + e_yc^2)^(1/2) - (e_xc^2 + e_yc^2)^(3/2)/4) + sin(2*u_c - 2*atan2(e_yc, e_xc))*((5*e_xc^2)/4 + (5*e_yc^2)/4))*(e_xc^2 + e_yc^2)^(1/2) + e_xc^2 + e_yc^2 + 1)^(1/2))/(a_c^2*(e_xc^2 + e_yc^2)^(1/2)*(-mu/(a_c*(e_xc^2 + e_yc^2 - 1)))^(3/2)*(e_xc^2 + e_yc^2 - 1)^3) - (B_c*mu*rho*cos(u_c - atan2(e_yc, e_xc) + (13*sin(3*u_c - 3*atan2(e_yc, e_xc))*(e_xc^2 + e_yc^2)^(3/2))/12 + sin(u_c - atan2(e_yc, e_xc))*(2*(e_xc^2 + e_yc^2)^(1/2) - (e_xc^2 + e_yc^2)^(3/2)/4) + sin(2*u_c - 2*atan2(e_yc, e_xc))*((5*e_xc^2)/4 + (5*e_yc^2)/4))*(delta_B + 1)*(2*cos(u_c - atan2(e_yc, e_xc) + (13*sin(3*u_c - 3*atan2(e_yc, e_xc))*(e_xc^2 + e_yc^2)^(3/2))/12 + sin(u_c - atan2(e_yc, e_xc))*(2*(e_xc^2 + e_yc^2)^(1/2) - (e_xc^2 + e_yc^2)^(3/2)/4) + sin(2*u_c - 2*atan2(e_yc, e_xc))*((5*e_xc^2)/4 + (5*e_yc^2)/4))*(e_xc^2 + e_yc^2)^(1/2) + e_xc^2 + e_yc^2 + 1)^(1/2)*(e_xc/(e_xc^2 + e_yc^2) - sin(u_c - atan2(e_yc, e_xc))*((2*e_yc)/(e_xc^2 + e_yc^2)^(1/2) - (3*e_yc*(e_xc^2 + e_yc^2)^(1/2))/4) - (5*e_yc*sin(2*u_c - 2*atan2(e_yc, e_xc)))/2 + (13*e_xc*cos(3*u_c - 3*atan2(e_yc, e_xc))*(e_xc^2 + e_yc^2)^(1/2))/4 - (13*e_yc*sin(3*u_c - 3*atan2(e_yc, e_xc))*(e_xc^2 + e_yc^2)^(1/2))/4 + (e_xc*cos(u_c - atan2(e_yc, e_xc))*(2*(e_xc^2 + e_yc^2)^(1/2) - (e_xc^2 + e_yc^2)^(3/2)/4))/(e_xc^2 + e_yc^2) + (2*e_xc*cos(2*u_c - 2*atan2(e_yc, e_xc))*((5*e_xc^2)/4 + (5*e_yc^2)/4))/(e_xc^2 + e_yc^2)))/(a_c*(e_xc^2 + e_yc^2)^(1/2)*(-mu/(a_c*(e_xc^2 + e_yc^2 - 1)))^(1/2)*(e_xc^2 + e_yc^2 - 1)) - (B_c*mu*rho*sin(u_c - atan2(e_yc, e_xc) + (13*sin(3*u_c - 3*atan2(e_yc, e_xc))*(e_xc^2 + e_yc^2)^(3/2))/12 + sin(u_c - atan2(e_yc, e_xc))*(2*(e_xc^2 + e_yc^2)^(1/2) - (e_xc^2 + e_yc^2)^(3/2)/4) + sin(2*u_c - 2*atan2(e_yc, e_xc))*((5*e_xc^2)/4 + (5*e_yc^2)/4))^2*(delta_B + 1)*(e_xc/(e_xc^2 + e_yc^2) - sin(u_c - atan2(e_yc, e_xc))*((2*e_yc)/(e_xc^2 + e_yc^2)^(1/2) - (3*e_yc*(e_xc^2 + e_yc^2)^(1/2))/4) - (5*e_yc*sin(2*u_c - 2*atan2(e_yc, e_xc)))/2 + (13*e_xc*cos(3*u_c - 3*atan2(e_yc, e_xc))*(e_xc^2 + e_yc^2)^(1/2))/4 - (13*e_yc*sin(3*u_c - 3*atan2(e_yc, e_xc))*(e_xc^2 + e_yc^2)^(1/2))/4 + (e_xc*cos(u_c - atan2(e_yc, e_xc))*(2*(e_xc^2 + e_yc^2)^(1/2) - (e_xc^2 + e_yc^2)^(3/2)/4))/(e_xc^2 + e_yc^2) + (2*e_xc*cos(2*u_c - 2*atan2(e_yc, e_xc))*((5*e_xc^2)/4 + (5*e_yc^2)/4))/(e_xc^2 + e_yc^2)))/(a_c*(e_c^2 - 1)*(-mu/(a_c*(e_c^2 - 1)))^(1/2)*(2*e_c*cos(u_c - atan2(e_yc, e_xc) + (13*sin(3*u_c - 3*atan2(e_yc, e_xc))*(e_xc^2 + e_yc^2)^(3/2))/12 + sin(u_c - atan2(e_yc, e_xc))*(2*(e_xc^2 + e_yc^2)^(1/2) - (e_xc^2 + e_yc^2)^(3/2)/4) + sin(2*u_c - 2*atan2(e_yc, e_xc))*((5*e_xc^2)/4 + (5*e_yc^2)/4)) + e_c^2 + 1)^(1/2)) - (B_c*mu*rho*sin(u_c - atan2(e_yc, e_xc) + (13*sin(3*u_c - 3*atan2(e_yc, e_xc))*(e_xc^2 + e_yc^2)^(3/2))/12 + sin(u_c - atan2(e_yc, e_xc))*(2*(e_xc^2 + e_yc^2)^(1/2) - (e_xc^2 + e_yc^2)^(3/2)/4) + sin(2*u_c - 2*atan2(e_yc, e_xc))*((5*e_xc^2)/4 + (5*e_yc^2)/4))^2*(e_c^2/(e_c*cos(u_c - atan2(e_yc, e_xc) + (13*sin(3*u_c - 3*atan2(e_yc, e_xc))*(e_xc^2 + e_yc^2)^(3/2))/12 + sin(u_c - atan2(e_yc, e_xc))*(2*(e_xc^2 + e_yc^2)^(1/2) - (e_xc^2 + e_yc^2)^(3/2)/4) + sin(2*u_c - 2*atan2(e_yc, e_xc))*((5*e_xc^2)/4 + (5*e_yc^2)/4)) + 1) + 1)*(delta_B + 1)*(e_xc/(e_xc^2 + e_yc^2) - sin(u_c - atan2(e_yc, e_xc))*((2*e_yc)/(e_xc^2 + e_yc^2)^(1/2) - (3*e_yc*(e_xc^2 + e_yc^2)^(1/2))/4) - (5*e_yc*sin(2*u_c - 2*atan2(e_yc, e_xc)))/2 + (13*e_xc*cos(3*u_c - 3*atan2(e_yc, e_xc))*(e_xc^2 + e_yc^2)^(1/2))/4 - (13*e_yc*sin(3*u_c - 3*atan2(e_yc, e_xc))*(e_xc^2 + e_yc^2)^(1/2))/4 + (e_xc*cos(u_c - atan2(e_yc, e_xc))*(2*(e_xc^2 + e_yc^2)^(1/2) - (e_xc^2 + e_yc^2)^(3/2)/4))/(e_xc^2 + e_yc^2) + (2*e_xc*cos(2*u_c - 2*atan2(e_yc, e_xc))*((5*e_xc^2)/4 + (5*e_yc^2)/4))/(e_xc^2 + e_yc^2)))/(a_c*(1 - e_c^2)^(1/2)*(-mu/(a_c*(e_c^2 - 1)))^(1/2)*(2*e_c*cos(u_c - atan2(e_yc, e_xc) + (13*sin(3*u_c - 3*atan2(e_yc, e_xc))*(e_xc^2 + e_yc^2)^(3/2))/12 + sin(u_c - atan2(e_yc, e_xc))*(2*(e_xc^2 + e_yc^2)^(1/2) - (e_xc^2 + e_yc^2)^(3/2)/4) + sin(2*u_c - 2*atan2(e_yc, e_xc))*((5*e_xc^2)/4 + (5*e_yc^2)/4)) + e_c^2 + 1)^(1/2)) - (2*B_c*e_yc*mu*rho*sin(u_c - atan2(e_yc, e_xc) + (13*sin(3*u_c - 3*atan2(e_yc, e_xc))*(e_xc^2 + e_yc^2)^(3/2))/12 + sin(u_c - atan2(e_yc, e_xc))*(2*(e_xc^2 + e_yc^2)^(1/2) - (e_xc^2 + e_yc^2)^(3/2)/4) + sin(2*u_c - 2*atan2(e_yc, e_xc))*((5*e_xc^2)/4 + (5*e_yc^2)/4))*(delta_B + 1)*(2*cos(u_c - atan2(e_yc, e_xc) + (13*sin(3*u_c - 3*atan2(e_yc, e_xc))*(e_xc^2 + e_yc^2)^(3/2))/12 + sin(u_c - atan2(e_yc, e_xc))*(2*(e_xc^2 + e_yc^2)^(1/2) - (e_xc^2 + e_yc^2)^(3/2)/4) + sin(2*u_c - 2*atan2(e_yc, e_xc))*((5*e_xc^2)/4 + (5*e_yc^2)/4))*(e_xc^2 + e_yc^2)^(1/2) + e_xc^2 + e_yc^2 + 1)^(1/2))/(a_c*(e_xc^2 + e_yc^2)^(1/2)*(-mu/(a_c*(e_xc^2 + e_yc^2 - 1)))^(1/2)*(e_xc^2 + e_yc^2 - 1)^2) - (B_c*e_yc*mu*rho*sin(u_c - atan2(e_yc, e_xc) + (13*sin(3*u_c - 3*atan2(e_yc, e_xc))*(e_xc^2 + e_yc^2)^(3/2))/12 + sin(u_c - atan2(e_yc, e_xc))*(2*(e_xc^2 + e_yc^2)^(1/2) - (e_xc^2 + e_yc^2)^(3/2)/4) + sin(2*u_c - 2*atan2(e_yc, e_xc))*((5*e_xc^2)/4 + (5*e_yc^2)/4))*(delta_B + 1)*(2*cos(u_c - atan2(e_yc, e_xc) + (13*sin(3*u_c - 3*atan2(e_yc, e_xc))*(e_xc^2 + e_yc^2)^(3/2))/12 + sin(u_c - atan2(e_yc, e_xc))*(2*(e_xc^2 + e_yc^2)^(1/2) - (e_xc^2 + e_yc^2)^(3/2)/4) + sin(2*u_c - 2*atan2(e_yc, e_xc))*((5*e_xc^2)/4 + (5*e_yc^2)/4))*(e_xc^2 + e_yc^2)^(1/2) + e_xc^2 + e_yc^2 + 1)^(1/2))/(a_c*(e_xc^2 + e_yc^2)^(3/2)*(-mu/(a_c*(e_xc^2 + e_yc^2 - 1)))^(1/2)*(e_xc^2 + e_yc^2 - 1)) + (B_c*mu*rho*cos(u_c - atan2(e_yc, e_xc) + (13*sin(3*u_c - 3*atan2(e_yc, e_xc))*(e_xc^2 + e_yc^2)^(3/2))/12 + sin(u_c - atan2(e_yc, e_xc))*(2*(e_xc^2 + e_yc^2)^(1/2) - (e_xc^2 + e_yc^2)^(3/2)/4) + sin(2*u_c - 2*atan2(e_yc, e_xc))*((5*e_xc^2)/4 + (5*e_yc^2)/4))*(delta_B + 1)*(2*e_c*cos(u_c - atan2(e_yc, e_xc) + (13*sin(3*u_c - 3*atan2(e_yc, e_xc))*(e_xc^2 + e_yc^2)^(3/2))/12 + sin(u_c - atan2(e_yc, e_xc))*(2*(e_xc^2 + e_yc^2)^(1/2) - (e_xc^2 + e_yc^2)^(3/2)/4) + sin(2*u_c - 2*atan2(e_yc, e_xc))*((5*e_xc^2)/4 + (5*e_yc^2)/4)) + e_c^2 + 1)^(1/2)*(e_xc/(e_xc^2 + e_yc^2) - sin(u_c - atan2(e_yc, e_xc))*((2*e_yc)/(e_xc^2 + e_yc^2)^(1/2) - (3*e_yc*(e_xc^2 + e_yc^2)^(1/2))/4) - (5*e_yc*sin(2*u_c - 2*atan2(e_yc, e_xc)))/2 + (13*e_xc*cos(3*u_c - 3*atan2(e_yc, e_xc))*(e_xc^2 + e_yc^2)^(1/2))/4 - (13*e_yc*sin(3*u_c - 3*atan2(e_yc, e_xc))*(e_xc^2 + e_yc^2)^(1/2))/4 + (e_xc*cos(u_c - atan2(e_yc, e_xc))*(2*(e_xc^2 + e_yc^2)^(1/2) - (e_xc^2 + e_yc^2)^(3/2)/4))/(e_xc^2 + e_yc^2) + (2*e_xc*cos(2*u_c - 2*atan2(e_yc, e_xc))*((5*e_xc^2)/4 + (5*e_yc^2)/4))/(e_xc^2 + e_yc^2)))/(a_c*e_c*(e_c^2 - 1)*(-mu/(a_c*(e_c^2 - 1)))^(1/2)) + (B_c*mu*rho*sin(u_c - atan2(e_yc, e_xc) + (13*sin(3*u_c - 3*atan2(e_yc, e_xc))*(e_xc^2 + e_yc^2)^(3/2))/12 + sin(u_c - atan2(e_yc, e_xc))*(2*(e_xc^2 + e_yc^2)^(1/2) - (e_xc^2 + e_yc^2)^(3/2)/4) + sin(2*u_c - 2*atan2(e_yc, e_xc))*((5*e_xc^2)/4 + (5*e_yc^2)/4))*(delta_B + 1)*(2*e_yc + (2*e_yc*cos(u_c - atan2(e_yc, e_xc) + (13*sin(3*u_c - 3*atan2(e_yc, e_xc))*(e_xc^2 + e_yc^2)^(3/2))/12 + sin(u_c - atan2(e_yc, e_xc))*(2*(e_xc^2 + e_yc^2)^(1/2) - (e_xc^2 + e_yc^2)^(3/2)/4) + sin(2*u_c - 2*atan2(e_yc, e_xc))*((5*e_xc^2)/4 + (5*e_yc^2)/4)))/(e_xc^2 + e_yc^2)^(1/2) + 2*sin(u_c - atan2(e_yc, e_xc) + (13*sin(3*u_c - 3*atan2(e_yc, e_xc))*(e_xc^2 + e_yc^2)^(3/2))/12 + sin(u_c - atan2(e_yc, e_xc))*(2*(e_xc^2 + e_yc^2)^(1/2) - (e_xc^2 + e_yc^2)^(3/2)/4) + sin(2*u_c - 2*atan2(e_yc, e_xc))*((5*e_xc^2)/4 + (5*e_yc^2)/4))*(e_xc^2 + e_yc^2)^(1/2)*(e_xc/(e_xc^2 + e_yc^2) - sin(u_c - atan2(e_yc, e_xc))*((2*e_yc)/(e_xc^2 + e_yc^2)^(1/2) - (3*e_yc*(e_xc^2 + e_yc^2)^(1/2))/4) - (5*e_yc*sin(2*u_c - 2*atan2(e_yc, e_xc)))/2 + (13*e_xc*cos(3*u_c - 3*atan2(e_yc, e_xc))*(e_xc^2 + e_yc^2)^(1/2))/4 - (13*e_yc*sin(3*u_c - 3*atan2(e_yc, e_xc))*(e_xc^2 + e_yc^2)^(1/2))/4 + (e_xc*cos(u_c - atan2(e_yc, e_xc))*(2*(e_xc^2 + e_yc^2)^(1/2) - (e_xc^2 + e_yc^2)^(3/2)/4))/(e_xc^2 + e_yc^2) + (2*e_xc*cos(2*u_c - 2*atan2(e_yc, e_xc))*((5*e_xc^2)/4 + (5*e_yc^2)/4))/(e_xc^2 + e_yc^2))))/(2*a_c*(e_xc^2 + e_yc^2)^(1/2)*(-mu/(a_c*(e_xc^2 + e_yc^2 - 1)))^(1/2)*(e_xc^2 + e_yc^2 - 1)*(2*cos(u_c - atan2(e_yc, e_xc) + (13*sin(3*u_c - 3*atan2(e_yc, e_xc))*(e_xc^2 + e_yc^2)^(3/2))/12 + sin(u_c - atan2(e_yc, e_xc))*(2*(e_xc^2 + e_yc^2)^(1/2) - (e_xc^2 + e_yc^2)^(3/2)/4) + sin(2*u_c - 2*atan2(e_yc, e_xc))*((5*e_xc^2)/4 + (5*e_yc^2)/4))*(e_xc^2 + e_yc^2)^(1/2) + e_xc^2 + e_yc^2 + 1)^(1/2)) - (B_c*mu*rho*cos(u_c - atan2(e_yc, e_xc) + (13*sin(3*u_c - 3*atan2(e_yc, e_xc))*(e_xc^2 + e_yc^2)^(3/2))/12 + sin(u_c - atan2(e_yc, e_xc))*(2*(e_xc^2 + e_yc^2)^(1/2) - (e_xc^2 + e_yc^2)^(3/2)/4) + sin(2*u_c - 2*atan2(e_yc, e_xc))*((5*e_xc^2)/4 + (5*e_yc^2)/4))*(delta_B + 1)*((e_xc^2 + e_yc^2)/(cos(u_c - atan2(e_yc, e_xc) + (13*sin(3*u_c - 3*atan2(e_yc, e_xc))*(e_xc^2 + e_yc^2)^(3/2))/12 + sin(u_c - atan2(e_yc, e_xc))*(2*(e_xc^2 + e_yc^2)^(1/2) - (e_xc^2 + e_yc^2)^(3/2)/4) + sin(2*u_c - 2*atan2(e_yc, e_xc))*((5*e_xc^2)/4 + (5*e_yc^2)/4))*(e_xc^2 + e_yc^2)^(1/2) + 1) + 1)*(2*cos(u_c - atan2(e_yc, e_xc) + (13*sin(3*u_c - 3*atan2(e_yc, e_xc))*(e_xc^2 + e_yc^2)^(3/2))/12 + sin(u_c - atan2(e_yc, e_xc))*(2*(e_xc^2 + e_yc^2)^(1/2) - (e_xc^2 + e_yc^2)^(3/2)/4) + sin(2*u_c - 2*atan2(e_yc, e_xc))*((5*e_xc^2)/4 + (5*e_yc^2)/4))*(e_xc^2 + e_yc^2)^(1/2) + e_xc^2 + e_yc^2 + 1)^(1/2)*(e_xc/(e_xc^2 + e_yc^2) - sin(u_c - atan2(e_yc, e_xc))*((2*e_yc)/(e_xc^2 + e_yc^2)^(1/2) - (3*e_yc*(e_xc^2 + e_yc^2)^(1/2))/4) - (5*e_yc*sin(2*u_c - 2*atan2(e_yc, e_xc)))/2 + (13*e_xc*cos(3*u_c - 3*atan2(e_yc, e_xc))*(e_xc^2 + e_yc^2)^(1/2))/4 - (13*e_yc*sin(3*u_c - 3*atan2(e_yc, e_xc))*(e_xc^2 + e_yc^2)^(1/2))/4 + (e_xc*cos(u_c - atan2(e_yc, e_xc))*(2*(e_xc^2 + e_yc^2)^(1/2) - (e_xc^2 + e_yc^2)^(3/2)/4))/(e_xc^2 + e_yc^2) + (2*e_xc*cos(2*u_c - 2*atan2(e_yc, e_xc))*((5*e_xc^2)/4 + (5*e_yc^2)/4))/(e_xc^2 + e_yc^2)))/(a_c*(e_xc^2 + e_yc^2)^(1/2)*(-mu/(a_c*(e_xc^2 + e_yc^2 - 1)))^(1/2)*(1 - e_yc^2 - e_xc^2)^(1/2)) + (B_c*e_yc*mu*rho*sin(u_c - atan2(e_yc, e_xc) + (13*sin(3*u_c - 3*atan2(e_yc, e_xc))*(e_xc^2 + e_yc^2)^(3/2))/12 + sin(u_c - atan2(e_yc, e_xc))*(2*(e_xc^2 + e_yc^2)^(1/2) - (e_xc^2 + e_yc^2)^(3/2)/4) + sin(2*u_c - 2*atan2(e_yc, e_xc))*((5*e_xc^2)/4 + (5*e_yc^2)/4))*(delta_B + 1)*((e_xc^2 + e_yc^2)/(cos(u_c - atan2(e_yc, e_xc) + (13*sin(3*u_c - 3*atan2(e_yc, e_xc))*(e_xc^2 + e_yc^2)^(3/2))/12 + sin(u_c - atan2(e_yc, e_xc))*(2*(e_xc^2 + e_yc^2)^(1/2) - (e_xc^2 + e_yc^2)^(3/2)/4) + sin(2*u_c - 2*atan2(e_yc, e_xc))*((5*e_xc^2)/4 + (5*e_yc^2)/4))*(e_xc^2 + e_yc^2)^(1/2) + 1) + 1)*(2*cos(u_c - atan2(e_yc, e_xc) + (13*sin(3*u_c - 3*atan2(e_yc, e_xc))*(e_xc^2 + e_yc^2)^(3/2))/12 + sin(u_c - atan2(e_yc, e_xc))*(2*(e_xc^2 + e_yc^2)^(1/2) - (e_xc^2 + e_yc^2)^(3/2)/4) + sin(2*u_c - 2*atan2(e_yc, e_xc))*((5*e_xc^2)/4 + (5*e_yc^2)/4))*(e_xc^2 + e_yc^2)^(1/2) + e_xc^2 + e_yc^2 + 1)^(1/2))/(a_c*(e_xc^2 + e_yc^2)^(1/2)*(-mu/(a_c*(e_xc^2 + e_yc^2 - 1)))^(1/2)*(1 - e_yc^2 - e_xc^2)^(3/2)) - (B_c*e_yc*mu*rho*sin(u_c - atan2(e_yc, e_xc) + (13*sin(3*u_c - 3*atan2(e_yc, e_xc))*(e_xc^2 + e_yc^2)^(3/2))/12 + sin(u_c - atan2(e_yc, e_xc))*(2*(e_xc^2 + e_yc^2)^(1/2) - (e_xc^2 + e_yc^2)^(3/2)/4) + sin(2*u_c - 2*atan2(e_yc, e_xc))*((5*e_xc^2)/4 + (5*e_yc^2)/4))*(delta_B + 1)*((e_xc^2 + e_yc^2)/(cos(u_c - atan2(e_yc, e_xc) + (13*sin(3*u_c - 3*atan2(e_yc, e_xc))*(e_xc^2 + e_yc^2)^(3/2))/12 + sin(u_c - atan2(e_yc, e_xc))*(2*(e_xc^2 + e_yc^2)^(1/2) - (e_xc^2 + e_yc^2)^(3/2)/4) + sin(2*u_c - 2*atan2(e_yc, e_xc))*((5*e_xc^2)/4 + (5*e_yc^2)/4))*(e_xc^2 + e_yc^2)^(1/2) + 1) + 1)*(2*cos(u_c - atan2(e_yc, e_xc) + (13*sin(3*u_c - 3*atan2(e_yc, e_xc))*(e_xc^2 + e_yc^2)^(3/2))/12 + sin(u_c - atan2(e_yc, e_xc))*(2*(e_xc^2 + e_yc^2)^(1/2) - (e_xc^2 + e_yc^2)^(3/2)/4) + sin(2*u_c - 2*atan2(e_yc, e_xc))*((5*e_xc^2)/4 + (5*e_yc^2)/4))*(e_xc^2 + e_yc^2)^(1/2) + e_xc^2 + e_yc^2 + 1)^(1/2))/(a_c*(e_xc^2 + e_yc^2)^(3/2)*(-mu/(a_c*(e_xc^2 + e_yc^2 - 1)))^(1/2)*(1 - e_yc^2 - e_xc^2)^(1/2)) + (B_c*mu*rho*sin(u_c - atan2(e_yc, e_xc) + (13*sin(3*u_c - 3*atan2(e_yc, e_xc))*(e_xc^2 + e_yc^2)^(3/2))/12 + sin(u_c - atan2(e_yc, e_xc))*(2*(e_xc^2 + e_yc^2)^(1/2) - (e_xc^2 + e_yc^2)^(3/2)/4) + sin(2*u_c - 2*atan2(e_yc, e_xc))*((5*e_xc^2)/4 + (5*e_yc^2)/4))*(delta_B + 1)*((e_xc^2 + e_yc^2)/(cos(u_c - atan2(e_yc, e_xc) + (13*sin(3*u_c - 3*atan2(e_yc, e_xc))*(e_xc^2 + e_yc^2)^(3/2))/12 + sin(u_c - atan2(e_yc, e_xc))*(2*(e_xc^2 + e_yc^2)^(1/2) - (e_xc^2 + e_yc^2)^(3/2)/4) + sin(2*u_c - 2*atan2(e_yc, e_xc))*((5*e_xc^2)/4 + (5*e_yc^2)/4))*(e_xc^2 + e_yc^2)^(1/2) + 1) + 1)*(2*e_yc + (2*e_yc*cos(u_c - atan2(e_yc, e_xc) + (13*sin(3*u_c - 3*atan2(e_yc, e_xc))*(e_xc^2 + e_yc^2)^(3/2))/12 + sin(u_c - atan2(e_yc, e_xc))*(2*(e_xc^2 + e_yc^2)^(1/2) - (e_xc^2 + e_yc^2)^(3/2)/4) + sin(2*u_c - 2*atan2(e_yc, e_xc))*((5*e_xc^2)/4 + (5*e_yc^2)/4)))/(e_xc^2 + e_yc^2)^(1/2) + 2*sin(u_c - atan2(e_yc, e_xc) + (13*sin(3*u_c - 3*atan2(e_yc, e_xc))*(e_xc^2 + e_yc^2)^(3/2))/12 + sin(u_c - atan2(e_yc, e_xc))*(2*(e_xc^2 + e_yc^2)^(1/2) - (e_xc^2 + e_yc^2)^(3/2)/4) + sin(2*u_c - 2*atan2(e_yc, e_xc))*((5*e_xc^2)/4 + (5*e_yc^2)/4))*(e_xc^2 + e_yc^2)^(1/2)*(e_xc/(e_xc^2 + e_yc^2) - sin(u_c - atan2(e_yc, e_xc))*((2*e_yc)/(e_xc^2 + e_yc^2)^(1/2) - (3*e_yc*(e_xc^2 + e_yc^2)^(1/2))/4) - (5*e_yc*sin(2*u_c - 2*atan2(e_yc, e_xc)))/2 + (13*e_xc*cos(3*u_c - 3*atan2(e_yc, e_xc))*(e_xc^2 + e_yc^2)^(1/2))/4 - (13*e_yc*sin(3*u_c - 3*atan2(e_yc, e_xc))*(e_xc^2 + e_yc^2)^(1/2))/4 + (e_xc*cos(u_c - atan2(e_yc, e_xc))*(2*(e_xc^2 + e_yc^2)^(1/2) - (e_xc^2 + e_yc^2)^(3/2)/4))/(e_xc^2 + e_yc^2) + (2*e_xc*cos(2*u_c - 2*atan2(e_yc, e_xc))*((5*e_xc^2)/4 + (5*e_yc^2)/4))/(e_xc^2 + e_yc^2))))/(2*a_c*(e_xc^2 + e_yc^2)^(1/2)*(-mu/(a_c*(e_xc^2 + e_yc^2 - 1)))^(1/2)*(1 - e_yc^2 - e_xc^2)^(1/2)*(2*cos(u_c - atan2(e_yc, e_xc) + (13*sin(3*u_c - 3*atan2(e_yc, e_xc))*(e_xc^2 + e_yc^2)^(3/2))/12 + sin(u_c - atan2(e_yc, e_xc))*(2*(e_xc^2 + e_yc^2)^(1/2) - (e_xc^2 + e_yc^2)^(3/2)/4) + sin(2*u_c - 2*atan2(e_yc, e_xc))*((5*e_xc^2)/4 + (5*e_yc^2)/4))*(e_xc^2 + e_yc^2)^(1/2) + e_xc^2 + e_yc^2 + 1)^(1/2)) - (B_c*e_yc*mu^2*rho*sin(u_c - atan2(e_yc, e_xc) + (13*sin(3*u_c - 3*atan2(e_yc, e_xc))*(e_xc^2 + e_yc^2)^(3/2))/12 + sin(u_c - atan2(e_yc, e_xc))*(2*(e_xc^2 + e_yc^2)^(1/2) - (e_xc^2 + e_yc^2)^(3/2)/4) + sin(2*u_c - 2*atan2(e_yc, e_xc))*((5*e_xc^2)/4 + (5*e_yc^2)/4))*(delta_B + 1)*((e_xc^2 + e_yc^2)/(cos(u_c - atan2(e_yc, e_xc) + (13*sin(3*u_c - 3*atan2(e_yc, e_xc))*(e_xc^2 + e_yc^2)^(3/2))/12 + sin(u_c - atan2(e_yc, e_xc))*(2*(e_xc^2 + e_yc^2)^(1/2) - (e_xc^2 + e_yc^2)^(3/2)/4) + sin(2*u_c - 2*atan2(e_yc, e_xc))*((5*e_xc^2)/4 + (5*e_yc^2)/4))*(e_xc^2 + e_yc^2)^(1/2) + 1) + 1)*(2*cos(u_c - atan2(e_yc, e_xc) + (13*sin(3*u_c - 3*atan2(e_yc, e_xc))*(e_xc^2 + e_yc^2)^(3/2))/12 + sin(u_c - atan2(e_yc, e_xc))*(2*(e_xc^2 + e_yc^2)^(1/2) - (e_xc^2 + e_yc^2)^(3/2)/4) + sin(2*u_c - 2*atan2(e_yc, e_xc))*((5*e_xc^2)/4 + (5*e_yc^2)/4))*(e_xc^2 + e_yc^2)^(1/2) + e_xc^2 + e_yc^2 + 1)^(1/2))/(a_c^2*(e_xc^2 + e_yc^2)^(1/2)*(-mu/(a_c*(e_xc^2 + e_yc^2 - 1)))^(3/2)*(1 - e_yc^2 - e_xc^2)^(5/2)) + (B_c*e_c^2*mu*rho*sin(u_c - atan2(e_yc, e_xc) + (13*sin(3*u_c - 3*atan2(e_yc, e_xc))*(e_xc^2 + e_yc^2)^(3/2))/12 + sin(u_c - atan2(e_yc, e_xc))*(2*(e_xc^2 + e_yc^2)^(1/2) - (e_xc^2 + e_yc^2)^(3/2)/4) + sin(2*u_c - 2*atan2(e_yc, e_xc))*((5*e_xc^2)/4 + (5*e_yc^2)/4))^2*(delta_B + 1)*(2*e_c*cos(u_c - atan2(e_yc, e_xc) + (13*sin(3*u_c - 3*atan2(e_yc, e_xc))*(e_xc^2 + e_yc^2)^(3/2))/12 + sin(u_c - atan2(e_yc, e_xc))*(2*(e_xc^2 + e_yc^2)^(1/2) - (e_xc^2 + e_yc^2)^(3/2)/4) + sin(2*u_c - 2*atan2(e_yc, e_xc))*((5*e_xc^2)/4 + (5*e_yc^2)/4)) + e_c^2 + 1)^(1/2)*(e_xc/(e_xc^2 + e_yc^2) - sin(u_c - atan2(e_yc, e_xc))*((2*e_yc)/(e_xc^2 + e_yc^2)^(1/2) - (3*e_yc*(e_xc^2 + e_yc^2)^(1/2))/4) - (5*e_yc*sin(2*u_c - 2*atan2(e_yc, e_xc)))/2 + (13*e_xc*cos(3*u_c - 3*atan2(e_yc, e_xc))*(e_xc^2 + e_yc^2)^(1/2))/4 - (13*e_yc*sin(3*u_c - 3*atan2(e_yc, e_xc))*(e_xc^2 + e_yc^2)^(1/2))/4 + (e_xc*cos(u_c - atan2(e_yc, e_xc))*(2*(e_xc^2 + e_yc^2)^(1/2) - (e_xc^2 + e_yc^2)^(3/2)/4))/(e_xc^2 + e_yc^2) + (2*e_xc*cos(2*u_c - 2*atan2(e_yc, e_xc))*((5*e_xc^2)/4 + (5*e_yc^2)/4))/(e_xc^2 + e_yc^2)))/(a_c*(1 - e_c^2)^(1/2)*(e_c*cos(u_c - atan2(e_yc, e_xc) + (13*sin(3*u_c - 3*atan2(e_yc, e_xc))*(e_xc^2 + e_yc^2)^(3/2))/12 + sin(u_c - atan2(e_yc, e_xc))*(2*(e_xc^2 + e_yc^2)^(1/2) - (e_xc^2 + e_yc^2)^(3/2)/4) + sin(2*u_c - 2*atan2(e_yc, e_xc))*((5*e_xc^2)/4 + (5*e_yc^2)/4)) + 1)^2*(-mu/(a_c*(e_c^2 - 1)))^(1/2)) + (B_c*mu*rho*cos(u_c - atan2(e_yc, e_xc) + (13*sin(3*u_c - 3*atan2(e_yc, e_xc))*(e_xc^2 + e_yc^2)^(3/2))/12 + sin(u_c - atan2(e_yc, e_xc))*(2*(e_xc^2 + e_yc^2)^(1/2) - (e_xc^2 + e_yc^2)^(3/2)/4) + sin(2*u_c - 2*atan2(e_yc, e_xc))*((5*e_xc^2)/4 + (5*e_yc^2)/4))*(e_c^2/(e_c*cos(u_c - atan2(e_yc, e_xc) + (13*sin(3*u_c - 3*atan2(e_yc, e_xc))*(e_xc^2 + e_yc^2)^(3/2))/12 + sin(u_c - atan2(e_yc, e_xc))*(2*(e_xc^2 + e_yc^2)^(1/2) - (e_xc^2 + e_yc^2)^(3/2)/4) + sin(2*u_c - 2*atan2(e_yc, e_xc))*((5*e_xc^2)/4 + (5*e_yc^2)/4)) + 1) + 1)*(delta_B + 1)*(2*e_c*cos(u_c - atan2(e_yc, e_xc) + (13*sin(3*u_c - 3*atan2(e_yc, e_xc))*(e_xc^2 + e_yc^2)^(3/2))/12 + sin(u_c - atan2(e_yc, e_xc))*(2*(e_xc^2 + e_yc^2)^(1/2) - (e_xc^2 + e_yc^2)^(3/2)/4) + sin(2*u_c - 2*atan2(e_yc, e_xc))*((5*e_xc^2)/4 + (5*e_yc^2)/4)) + e_c^2 + 1)^(1/2)*(e_xc/(e_xc^2 + e_yc^2) - sin(u_c - atan2(e_yc, e_xc))*((2*e_yc)/(e_xc^2 + e_yc^2)^(1/2) - (3*e_yc*(e_xc^2 + e_yc^2)^(1/2))/4) - (5*e_yc*sin(2*u_c - 2*atan2(e_yc, e_xc)))/2 + (13*e_xc*cos(3*u_c - 3*atan2(e_yc, e_xc))*(e_xc^2 + e_yc^2)^(1/2))/4 - (13*e_yc*sin(3*u_c - 3*atan2(e_yc, e_xc))*(e_xc^2 + e_yc^2)^(1/2))/4 + (e_xc*cos(u_c - atan2(e_yc, e_xc))*(2*(e_xc^2 + e_yc^2)^(1/2) - (e_xc^2 + e_yc^2)^(3/2)/4))/(e_xc^2 + e_yc^2) + (2*e_xc*cos(2*u_c - 2*atan2(e_yc, e_xc))*((5*e_xc^2)/4 + (5*e_yc^2)/4))/(e_xc^2 + e_yc^2)))/(a_c*e_c*(1 - e_c^2)^(1/2)*(-mu/(a_c*(e_c^2 - 1)))^(1/2));
% A_drag(2,5) = 0;
% A_drag(2,6) = (B_c*mu*rho*sin(u_c - atan2(e_yc, e_xc) + (13*sin(3*u_c - 3*atan2(e_yc, e_xc))*(e_xc^2 + e_yc^2)^(3/2))/12 + sin(u_c - atan2(e_yc, e_xc))*(2*(e_xc^2 + e_yc^2)^(1/2) - (e_xc^2 + e_yc^2)^(3/2)/4) + sin(2*u_c - 2*atan2(e_yc, e_xc))*((5*e_xc^2)/4 + (5*e_yc^2)/4))^2*(delta_B + 1)*(1/tan(i_c) + (2*cos(2*u_c - 2*atan2(e_yc, e_xc))*((5*e_xc^2)/4 + (5*e_yc^2)/4))/tan(i_c) + (13*cos(3*u_c - 3*atan2(e_yc, e_xc))*(e_xc^2 + e_yc^2)^(3/2))/(4*tan(i_c)) + (cos(u_c - atan2(e_yc, e_xc))*(2*(e_xc^2 + e_yc^2)^(1/2) - (e_xc^2 + e_yc^2)^(3/2)/4))/tan(i_c)))/(a_c*(-mu/(a_c*(e_xc^2 + e_yc^2 - 1)))^(1/2)*(e_xc^2 + e_yc^2 - 1)*(2*cos(u_c - atan2(e_yc, e_xc) + (13*sin(3*u_c - 3*atan2(e_yc, e_xc))*(e_xc^2 + e_yc^2)^(3/2))/12 + sin(u_c - atan2(e_yc, e_xc))*(2*(e_xc^2 + e_yc^2)^(1/2) - (e_xc^2 + e_yc^2)^(3/2)/4) + sin(2*u_c - 2*atan2(e_yc, e_xc))*((5*e_xc^2)/4 + (5*e_yc^2)/4))*(e_xc^2 + e_yc^2)^(1/2) + e_xc^2 + e_yc^2 + 1)^(1/2)) - (B_c*mu*rho*sin(u_c - atan2(e_yc, e_xc) + (13*sin(3*u_c - 3*atan2(e_yc, e_xc))*(e_xc^2 + e_yc^2)^(3/2))/12 + sin(u_c - atan2(e_yc, e_xc))*(2*(e_xc^2 + e_yc^2)^(1/2) - (e_xc^2 + e_yc^2)^(3/2)/4) + sin(2*u_c - 2*atan2(e_yc, e_xc))*((5*e_xc^2)/4 + (5*e_yc^2)/4))^2*(delta_B + 1)*(1/tan(i_c) + (2*cos(2*u_c - 2*atan2(e_yc, e_xc))*((5*e_xc^2)/4 + (5*e_yc^2)/4))/tan(i_c) + (13*cos(3*u_c - 3*atan2(e_yc, e_xc))*(e_xc^2 + e_yc^2)^(3/2))/(4*tan(i_c)) + (cos(u_c - atan2(e_yc, e_xc))*(2*(e_xc^2 + e_yc^2)^(1/2) - (e_xc^2 + e_yc^2)^(3/2)/4))/tan(i_c)))/(a_c*(e_c^2 - 1)*(-mu/(a_c*(e_c^2 - 1)))^(1/2)*(2*e_c*cos(u_c - atan2(e_yc, e_xc) + (13*sin(3*u_c - 3*atan2(e_yc, e_xc))*(e_xc^2 + e_yc^2)^(3/2))/12 + sin(u_c - atan2(e_yc, e_xc))*(2*(e_xc^2 + e_yc^2)^(1/2) - (e_xc^2 + e_yc^2)^(3/2)/4) + sin(2*u_c - 2*atan2(e_yc, e_xc))*((5*e_xc^2)/4 + (5*e_yc^2)/4)) + e_c^2 + 1)^(1/2)) + (B_c*mu*rho*sin(u_c - atan2(e_yc, e_xc) + (13*sin(3*u_c - 3*atan2(e_yc, e_xc))*(e_xc^2 + e_yc^2)^(3/2))/12 + sin(u_c - atan2(e_yc, e_xc))*(2*(e_xc^2 + e_yc^2)^(1/2) - (e_xc^2 + e_yc^2)^(3/2)/4) + sin(2*u_c - 2*atan2(e_yc, e_xc))*((5*e_xc^2)/4 + (5*e_yc^2)/4))^2*(delta_B + 1)*((e_xc^2 + e_yc^2)/(cos(u_c - atan2(e_yc, e_xc) + (13*sin(3*u_c - 3*atan2(e_yc, e_xc))*(e_xc^2 + e_yc^2)^(3/2))/12 + sin(u_c - atan2(e_yc, e_xc))*(2*(e_xc^2 + e_yc^2)^(1/2) - (e_xc^2 + e_yc^2)^(3/2)/4) + sin(2*u_c - 2*atan2(e_yc, e_xc))*((5*e_xc^2)/4 + (5*e_yc^2)/4))*(e_xc^2 + e_yc^2)^(1/2) + 1) + 1)*(1/tan(i_c) + (2*cos(2*u_c - 2*atan2(e_yc, e_xc))*((5*e_xc^2)/4 + (5*e_yc^2)/4))/tan(i_c) + (13*cos(3*u_c - 3*atan2(e_yc, e_xc))*(e_xc^2 + e_yc^2)^(3/2))/(4*tan(i_c)) + (cos(u_c - atan2(e_yc, e_xc))*(2*(e_xc^2 + e_yc^2)^(1/2) - (e_xc^2 + e_yc^2)^(3/2)/4))/tan(i_c)))/(a_c*(-mu/(a_c*(e_xc^2 + e_yc^2 - 1)))^(1/2)*(1 - e_yc^2 - e_xc^2)^(1/2)*(2*cos(u_c - atan2(e_yc, e_xc) + (13*sin(3*u_c - 3*atan2(e_yc, e_xc))*(e_xc^2 + e_yc^2)^(3/2))/12 + sin(u_c - atan2(e_yc, e_xc))*(2*(e_xc^2 + e_yc^2)^(1/2) - (e_xc^2 + e_yc^2)^(3/2)/4) + sin(2*u_c - 2*atan2(e_yc, e_xc))*((5*e_xc^2)/4 + (5*e_yc^2)/4))*(e_xc^2 + e_yc^2)^(1/2) + e_xc^2 + e_yc^2 + 1)^(1/2)) - (B_c*mu*rho*cos(u_c - atan2(e_yc, e_xc) + (13*sin(3*u_c - 3*atan2(e_yc, e_xc))*(e_xc^2 + e_yc^2)^(3/2))/12 + sin(u_c - atan2(e_yc, e_xc))*(2*(e_xc^2 + e_yc^2)^(1/2) - (e_xc^2 + e_yc^2)^(3/2)/4) + sin(2*u_c - 2*atan2(e_yc, e_xc))*((5*e_xc^2)/4 + (5*e_yc^2)/4))*(delta_B + 1)*(2*cos(u_c - atan2(e_yc, e_xc) + (13*sin(3*u_c - 3*atan2(e_yc, e_xc))*(e_xc^2 + e_yc^2)^(3/2))/12 + sin(u_c - atan2(e_yc, e_xc))*(2*(e_xc^2 + e_yc^2)^(1/2) - (e_xc^2 + e_yc^2)^(3/2)/4) + sin(2*u_c - 2*atan2(e_yc, e_xc))*((5*e_xc^2)/4 + (5*e_yc^2)/4))*(e_xc^2 + e_yc^2)^(1/2) + e_xc^2 + e_yc^2 + 1)^(1/2)*(1/tan(i_c) + (2*cos(2*u_c - 2*atan2(e_yc, e_xc))*((5*e_xc^2)/4 + (5*e_yc^2)/4))/tan(i_c) + (13*cos(3*u_c - 3*atan2(e_yc, e_xc))*(e_xc^2 + e_yc^2)^(3/2))/(4*tan(i_c)) + (cos(u_c - atan2(e_yc, e_xc))*(2*(e_xc^2 + e_yc^2)^(1/2) - (e_xc^2 + e_yc^2)^(3/2)/4))/tan(i_c)))/(a_c*(e_xc^2 + e_yc^2)^(1/2)*(-mu/(a_c*(e_xc^2 + e_yc^2 - 1)))^(1/2)*(e_xc^2 + e_yc^2 - 1)) - (B_c*mu*rho*sin(u_c - atan2(e_yc, e_xc) + (13*sin(3*u_c - 3*atan2(e_yc, e_xc))*(e_xc^2 + e_yc^2)^(3/2))/12 + sin(u_c - atan2(e_yc, e_xc))*(2*(e_xc^2 + e_yc^2)^(1/2) - (e_xc^2 + e_yc^2)^(3/2)/4) + sin(2*u_c - 2*atan2(e_yc, e_xc))*((5*e_xc^2)/4 + (5*e_yc^2)/4))^2*(e_c^2/(e_c*cos(u_c - atan2(e_yc, e_xc) + (13*sin(3*u_c - 3*atan2(e_yc, e_xc))*(e_xc^2 + e_yc^2)^(3/2))/12 + sin(u_c - atan2(e_yc, e_xc))*(2*(e_xc^2 + e_yc^2)^(1/2) - (e_xc^2 + e_yc^2)^(3/2)/4) + sin(2*u_c - 2*atan2(e_yc, e_xc))*((5*e_xc^2)/4 + (5*e_yc^2)/4)) + 1) + 1)*(delta_B + 1)*(1/tan(i_c) + (2*cos(2*u_c - 2*atan2(e_yc, e_xc))*((5*e_xc^2)/4 + (5*e_yc^2)/4))/tan(i_c) + (13*cos(3*u_c - 3*atan2(e_yc, e_xc))*(e_xc^2 + e_yc^2)^(3/2))/(4*tan(i_c)) + (cos(u_c - atan2(e_yc, e_xc))*(2*(e_xc^2 + e_yc^2)^(1/2) - (e_xc^2 + e_yc^2)^(3/2)/4))/tan(i_c)))/(a_c*(1 - e_c^2)^(1/2)*(-mu/(a_c*(e_c^2 - 1)))^(1/2)*(2*e_c*cos(u_c - atan2(e_yc, e_xc) + (13*sin(3*u_c - 3*atan2(e_yc, e_xc))*(e_xc^2 + e_yc^2)^(3/2))/12 + sin(u_c - atan2(e_yc, e_xc))*(2*(e_xc^2 + e_yc^2)^(1/2) - (e_xc^2 + e_yc^2)^(3/2)/4) + sin(2*u_c - 2*atan2(e_yc, e_xc))*((5*e_xc^2)/4 + (5*e_yc^2)/4)) + e_c^2 + 1)^(1/2)) + (B_c*mu*rho*cos(u_c - atan2(e_yc, e_xc) + (13*sin(3*u_c - 3*atan2(e_yc, e_xc))*(e_xc^2 + e_yc^2)^(3/2))/12 + sin(u_c - atan2(e_yc, e_xc))*(2*(e_xc^2 + e_yc^2)^(1/2) - (e_xc^2 + e_yc^2)^(3/2)/4) + sin(2*u_c - 2*atan2(e_yc, e_xc))*((5*e_xc^2)/4 + (5*e_yc^2)/4))*(delta_B + 1)*(2*e_c*cos(u_c - atan2(e_yc, e_xc) + (13*sin(3*u_c - 3*atan2(e_yc, e_xc))*(e_xc^2 + e_yc^2)^(3/2))/12 + sin(u_c - atan2(e_yc, e_xc))*(2*(e_xc^2 + e_yc^2)^(1/2) - (e_xc^2 + e_yc^2)^(3/2)/4) + sin(2*u_c - 2*atan2(e_yc, e_xc))*((5*e_xc^2)/4 + (5*e_yc^2)/4)) + e_c^2 + 1)^(1/2)*(1/tan(i_c) + (2*cos(2*u_c - 2*atan2(e_yc, e_xc))*((5*e_xc^2)/4 + (5*e_yc^2)/4))/tan(i_c) + (13*cos(3*u_c - 3*atan2(e_yc, e_xc))*(e_xc^2 + e_yc^2)^(3/2))/(4*tan(i_c)) + (cos(u_c - atan2(e_yc, e_xc))*(2*(e_xc^2 + e_yc^2)^(1/2) - (e_xc^2 + e_yc^2)^(3/2)/4))/tan(i_c)))/(a_c*e_c*(e_c^2 - 1)*(-mu/(a_c*(e_c^2 - 1)))^(1/2)) - (B_c*mu*rho*cos(u_c - atan2(e_yc, e_xc) + (13*sin(3*u_c - 3*atan2(e_yc, e_xc))*(e_xc^2 + e_yc^2)^(3/2))/12 + sin(u_c - atan2(e_yc, e_xc))*(2*(e_xc^2 + e_yc^2)^(1/2) - (e_xc^2 + e_yc^2)^(3/2)/4) + sin(2*u_c - 2*atan2(e_yc, e_xc))*((5*e_xc^2)/4 + (5*e_yc^2)/4))*(delta_B + 1)*((e_xc^2 + e_yc^2)/(cos(u_c - atan2(e_yc, e_xc) + (13*sin(3*u_c - 3*atan2(e_yc, e_xc))*(e_xc^2 + e_yc^2)^(3/2))/12 + sin(u_c - atan2(e_yc, e_xc))*(2*(e_xc^2 + e_yc^2)^(1/2) - (e_xc^2 + e_yc^2)^(3/2)/4) + sin(2*u_c - 2*atan2(e_yc, e_xc))*((5*e_xc^2)/4 + (5*e_yc^2)/4))*(e_xc^2 + e_yc^2)^(1/2) + 1) + 1)*(2*cos(u_c - atan2(e_yc, e_xc) + (13*sin(3*u_c - 3*atan2(e_yc, e_xc))*(e_xc^2 + e_yc^2)^(3/2))/12 + sin(u_c - atan2(e_yc, e_xc))*(2*(e_xc^2 + e_yc^2)^(1/2) - (e_xc^2 + e_yc^2)^(3/2)/4) + sin(2*u_c - 2*atan2(e_yc, e_xc))*((5*e_xc^2)/4 + (5*e_yc^2)/4))*(e_xc^2 + e_yc^2)^(1/2) + e_xc^2 + e_yc^2 + 1)^(1/2)*(1/tan(i_c) + (2*cos(2*u_c - 2*atan2(e_yc, e_xc))*((5*e_xc^2)/4 + (5*e_yc^2)/4))/tan(i_c) + (13*cos(3*u_c - 3*atan2(e_yc, e_xc))*(e_xc^2 + e_yc^2)^(3/2))/(4*tan(i_c)) + (cos(u_c - atan2(e_yc, e_xc))*(2*(e_xc^2 + e_yc^2)^(1/2) - (e_xc^2 + e_yc^2)^(3/2)/4))/tan(i_c)))/(a_c*(e_xc^2 + e_yc^2)^(1/2)*(-mu/(a_c*(e_xc^2 + e_yc^2 - 1)))^(1/2)*(1 - e_yc^2 - e_xc^2)^(1/2)) - (B_c*mu*rho*sin(u_c - atan2(e_yc, e_xc) + (13*sin(3*u_c - 3*atan2(e_yc, e_xc))*(e_xc^2 + e_yc^2)^(3/2))/12 + sin(u_c - atan2(e_yc, e_xc))*(2*(e_xc^2 + e_yc^2)^(1/2) - (e_xc^2 + e_yc^2)^(3/2)/4) + sin(2*u_c - 2*atan2(e_yc, e_xc))*((5*e_xc^2)/4 + (5*e_yc^2)/4))^2*(delta_B + 1)*(e_xc^2 + e_yc^2)*(2*cos(u_c - atan2(e_yc, e_xc) + (13*sin(3*u_c - 3*atan2(e_yc, e_xc))*(e_xc^2 + e_yc^2)^(3/2))/12 + sin(u_c - atan2(e_yc, e_xc))*(2*(e_xc^2 + e_yc^2)^(1/2) - (e_xc^2 + e_yc^2)^(3/2)/4) + sin(2*u_c - 2*atan2(e_yc, e_xc))*((5*e_xc^2)/4 + (5*e_yc^2)/4))*(e_xc^2 + e_yc^2)^(1/2) + e_xc^2 + e_yc^2 + 1)^(1/2)*(1/tan(i_c) + (2*cos(2*u_c - 2*atan2(e_yc, e_xc))*((5*e_xc^2)/4 + (5*e_yc^2)/4))/tan(i_c) + (13*cos(3*u_c - 3*atan2(e_yc, e_xc))*(e_xc^2 + e_yc^2)^(3/2))/(4*tan(i_c)) + (cos(u_c - atan2(e_yc, e_xc))*(2*(e_xc^2 + e_yc^2)^(1/2) - (e_xc^2 + e_yc^2)^(3/2)/4))/tan(i_c)))/(a_c*(cos(u_c - atan2(e_yc, e_xc) + (13*sin(3*u_c - 3*atan2(e_yc, e_xc))*(e_xc^2 + e_yc^2)^(3/2))/12 + sin(u_c - atan2(e_yc, e_xc))*(2*(e_xc^2 + e_yc^2)^(1/2) - (e_xc^2 + e_yc^2)^(3/2)/4) + sin(2*u_c - 2*atan2(e_yc, e_xc))*((5*e_xc^2)/4 + (5*e_yc^2)/4))*(e_xc^2 + e_yc^2)^(1/2) + 1)^2*(-mu/(a_c*(e_xc^2 + e_yc^2 - 1)))^(1/2)*(1 - e_yc^2 - e_xc^2)^(1/2)) + (B_c*e_c^2*mu*rho*sin(u_c - atan2(e_yc, e_xc) + (13*sin(3*u_c - 3*atan2(e_yc, e_xc))*(e_xc^2 + e_yc^2)^(3/2))/12 + sin(u_c - atan2(e_yc, e_xc))*(2*(e_xc^2 + e_yc^2)^(1/2) - (e_xc^2 + e_yc^2)^(3/2)/4) + sin(2*u_c - 2*atan2(e_yc, e_xc))*((5*e_xc^2)/4 + (5*e_yc^2)/4))^2*(delta_B + 1)*(2*e_c*cos(u_c - atan2(e_yc, e_xc) + (13*sin(3*u_c - 3*atan2(e_yc, e_xc))*(e_xc^2 + e_yc^2)^(3/2))/12 + sin(u_c - atan2(e_yc, e_xc))*(2*(e_xc^2 + e_yc^2)^(1/2) - (e_xc^2 + e_yc^2)^(3/2)/4) + sin(2*u_c - 2*atan2(e_yc, e_xc))*((5*e_xc^2)/4 + (5*e_yc^2)/4)) + e_c^2 + 1)^(1/2)*(1/tan(i_c) + (2*cos(2*u_c - 2*atan2(e_yc, e_xc))*((5*e_xc^2)/4 + (5*e_yc^2)/4))/tan(i_c) + (13*cos(3*u_c - 3*atan2(e_yc, e_xc))*(e_xc^2 + e_yc^2)^(3/2))/(4*tan(i_c)) + (cos(u_c - atan2(e_yc, e_xc))*(2*(e_xc^2 + e_yc^2)^(1/2) - (e_xc^2 + e_yc^2)^(3/2)/4))/tan(i_c)))/(a_c*(1 - e_c^2)^(1/2)*(e_c*cos(u_c - atan2(e_yc, e_xc) + (13*sin(3*u_c - 3*atan2(e_yc, e_xc))*(e_xc^2 + e_yc^2)^(3/2))/12 + sin(u_c - atan2(e_yc, e_xc))*(2*(e_xc^2 + e_yc^2)^(1/2) - (e_xc^2 + e_yc^2)^(3/2)/4) + sin(2*u_c - 2*atan2(e_yc, e_xc))*((5*e_xc^2)/4 + (5*e_yc^2)/4)) + 1)^2*(-mu/(a_c*(e_c^2 - 1)))^(1/2)) + (B_c*mu*rho*cos(u_c - atan2(e_yc, e_xc) + (13*sin(3*u_c - 3*atan2(e_yc, e_xc))*(e_xc^2 + e_yc^2)^(3/2))/12 + sin(u_c - atan2(e_yc, e_xc))*(2*(e_xc^2 + e_yc^2)^(1/2) - (e_xc^2 + e_yc^2)^(3/2)/4) + sin(2*u_c - 2*atan2(e_yc, e_xc))*((5*e_xc^2)/4 + (5*e_yc^2)/4))*(e_c^2/(e_c*cos(u_c - atan2(e_yc, e_xc) + (13*sin(3*u_c - 3*atan2(e_yc, e_xc))*(e_xc^2 + e_yc^2)^(3/2))/12 + sin(u_c - atan2(e_yc, e_xc))*(2*(e_xc^2 + e_yc^2)^(1/2) - (e_xc^2 + e_yc^2)^(3/2)/4) + sin(2*u_c - 2*atan2(e_yc, e_xc))*((5*e_xc^2)/4 + (5*e_yc^2)/4)) + 1) + 1)*(delta_B + 1)*(2*e_c*cos(u_c - atan2(e_yc, e_xc) + (13*sin(3*u_c - 3*atan2(e_yc, e_xc))*(e_xc^2 + e_yc^2)^(3/2))/12 + sin(u_c - atan2(e_yc, e_xc))*(2*(e_xc^2 + e_yc^2)^(1/2) - (e_xc^2 + e_yc^2)^(3/2)/4) + sin(2*u_c - 2*atan2(e_yc, e_xc))*((5*e_xc^2)/4 + (5*e_yc^2)/4)) + e_c^2 + 1)^(1/2)*(1/tan(i_c) + (2*cos(2*u_c - 2*atan2(e_yc, e_xc))*((5*e_xc^2)/4 + (5*e_yc^2)/4))/tan(i_c) + (13*cos(3*u_c - 3*atan2(e_yc, e_xc))*(e_xc^2 + e_yc^2)^(3/2))/(4*tan(i_c)) + (cos(u_c - atan2(e_yc, e_xc))*(2*(e_xc^2 + e_yc^2)^(1/2) - (e_xc^2 + e_yc^2)^(3/2)/4))/tan(i_c)))/(a_c*e_c*(1 - e_c^2)^(1/2)*(-mu/(a_c*(e_c^2 - 1)))^(1/2));
% A_drag(2,7) = (B_c*mu*rho*sin(u_c - atan2(e_yc, e_xc) + (13*sin(3*u_c - 3*atan2(e_yc, e_xc))*(e_xc^2 + e_yc^2)^(3/2))/12 + sin(u_c - atan2(e_yc, e_xc))*(2*(e_xc^2 + e_yc^2)^(1/2) - (e_xc^2 + e_yc^2)^(3/2)/4) + sin(2*u_c - 2*atan2(e_yc, e_xc))*((5*e_xc^2)/4 + (5*e_yc^2)/4))*(2*cos(u_c - atan2(e_yc, e_xc) + (13*sin(3*u_c - 3*atan2(e_yc, e_xc))*(e_xc^2 + e_yc^2)^(3/2))/12 + sin(u_c - atan2(e_yc, e_xc))*(2*(e_xc^2 + e_yc^2)^(1/2) - (e_xc^2 + e_yc^2)^(3/2)/4) + sin(2*u_c - 2*atan2(e_yc, e_xc))*((5*e_xc^2)/4 + (5*e_yc^2)/4))*(e_xc^2 + e_yc^2)^(1/2) + e_xc^2 + e_yc^2 + 1)^(1/2))/(a_c*(e_xc^2 + e_yc^2)^(1/2)*(-mu/(a_c*(e_xc^2 + e_yc^2 - 1)))^(1/2)*(e_xc^2 + e_yc^2 - 1)) - (B_c*mu*rho*sin(u_c - atan2(e_yc, e_xc) + (13*sin(3*u_c - 3*atan2(e_yc, e_xc))*(e_xc^2 + e_yc^2)^(3/2))/12 + sin(u_c - atan2(e_yc, e_xc))*(2*(e_xc^2 + e_yc^2)^(1/2) - (e_xc^2 + e_yc^2)^(3/2)/4) + sin(2*u_c - 2*atan2(e_yc, e_xc))*((5*e_xc^2)/4 + (5*e_yc^2)/4))*(2*e_c*cos(u_c - atan2(e_yc, e_xc) + (13*sin(3*u_c - 3*atan2(e_yc, e_xc))*(e_xc^2 + e_yc^2)^(3/2))/12 + sin(u_c - atan2(e_yc, e_xc))*(2*(e_xc^2 + e_yc^2)^(1/2) - (e_xc^2 + e_yc^2)^(3/2)/4) + sin(2*u_c - 2*atan2(e_yc, e_xc))*((5*e_xc^2)/4 + (5*e_yc^2)/4)) + e_c^2 + 1)^(1/2))/(a_c*e_c*(e_c^2 - 1)*(-mu/(a_c*(e_c^2 - 1)))^(1/2)) - (B_c*mu*rho*sin(u_c - atan2(e_yc, e_xc) + (13*sin(3*u_c - 3*atan2(e_yc, e_xc))*(e_xc^2 + e_yc^2)^(3/2))/12 + sin(u_c - atan2(e_yc, e_xc))*(2*(e_xc^2 + e_yc^2)^(1/2) - (e_xc^2 + e_yc^2)^(3/2)/4) + sin(2*u_c - 2*atan2(e_yc, e_xc))*((5*e_xc^2)/4 + (5*e_yc^2)/4))*(e_c^2/(e_c*cos(u_c - atan2(e_yc, e_xc) + (13*sin(3*u_c - 3*atan2(e_yc, e_xc))*(e_xc^2 + e_yc^2)^(3/2))/12 + sin(u_c - atan2(e_yc, e_xc))*(2*(e_xc^2 + e_yc^2)^(1/2) - (e_xc^2 + e_yc^2)^(3/2)/4) + sin(2*u_c - 2*atan2(e_yc, e_xc))*((5*e_xc^2)/4 + (5*e_yc^2)/4)) + 1) + 1)*(2*e_c*cos(u_c - atan2(e_yc, e_xc) + (13*sin(3*u_c - 3*atan2(e_yc, e_xc))*(e_xc^2 + e_yc^2)^(3/2))/12 + sin(u_c - atan2(e_yc, e_xc))*(2*(e_xc^2 + e_yc^2)^(1/2) - (e_xc^2 + e_yc^2)^(3/2)/4) + sin(2*u_c - 2*atan2(e_yc, e_xc))*((5*e_xc^2)/4 + (5*e_yc^2)/4)) + e_c^2 + 1)^(1/2))/(a_c*e_c*(1 - e_c^2)^(1/2)*(-mu/(a_c*(e_c^2 - 1)))^(1/2)) + (B_c*mu*rho*sin(u_c - atan2(e_yc, e_xc) + (13*sin(3*u_c - 3*atan2(e_yc, e_xc))*(e_xc^2 + e_yc^2)^(3/2))/12 + sin(u_c - atan2(e_yc, e_xc))*(2*(e_xc^2 + e_yc^2)^(1/2) - (e_xc^2 + e_yc^2)^(3/2)/4) + sin(2*u_c - 2*atan2(e_yc, e_xc))*((5*e_xc^2)/4 + (5*e_yc^2)/4))*((e_xc^2 + e_yc^2)/(cos(u_c - atan2(e_yc, e_xc) + (13*sin(3*u_c - 3*atan2(e_yc, e_xc))*(e_xc^2 + e_yc^2)^(3/2))/12 + sin(u_c - atan2(e_yc, e_xc))*(2*(e_xc^2 + e_yc^2)^(1/2) - (e_xc^2 + e_yc^2)^(3/2)/4) + sin(2*u_c - 2*atan2(e_yc, e_xc))*((5*e_xc^2)/4 + (5*e_yc^2)/4))*(e_xc^2 + e_yc^2)^(1/2) + 1) + 1)*(2*cos(u_c - atan2(e_yc, e_xc) + (13*sin(3*u_c - 3*atan2(e_yc, e_xc))*(e_xc^2 + e_yc^2)^(3/2))/12 + sin(u_c - atan2(e_yc, e_xc))*(2*(e_xc^2 + e_yc^2)^(1/2) - (e_xc^2 + e_yc^2)^(3/2)/4) + sin(2*u_c - 2*atan2(e_yc, e_xc))*((5*e_xc^2)/4 + (5*e_yc^2)/4))*(e_xc^2 + e_yc^2)^(1/2) + e_xc^2 + e_yc^2 + 1)^(1/2))/(a_c*(e_xc^2 + e_yc^2)^(1/2)*(-mu/(a_c*(e_xc^2 + e_yc^2 - 1)))^(1/2)*(1 - e_yc^2 - e_xc^2)^(1/2));
% A_drag(3,1) = (B_c*e_yc*mu^2*rho*sin(u_c - atan2(e_yc, e_xc) + (13*sin(3*u_c - 3*atan2(e_yc, e_xc))*(e_xc^2 + e_yc^2)^(3/2))/12 + sin(u_c - atan2(e_yc, e_xc))*(2*(e_xc^2 + e_yc^2)^(1/2) - (e_xc^2 + e_yc^2)^(3/2)/4) + sin(2*u_c - 2*atan2(e_yc, e_xc))*((5*e_xc^2)/4 + (5*e_yc^2)/4))*(delta_B + 1)*(2*cos(u_c - atan2(e_yc, e_xc) + (13*sin(3*u_c - 3*atan2(e_yc, e_xc))*(e_xc^2 + e_yc^2)^(3/2))/12 + sin(u_c - atan2(e_yc, e_xc))*(2*(e_xc^2 + e_yc^2)^(1/2) - (e_xc^2 + e_yc^2)^(3/2)/4) + sin(2*u_c - 2*atan2(e_yc, e_xc))*((5*e_xc^2)/4 + (5*e_yc^2)/4))*(e_xc^2 + e_yc^2)^(1/2) + e_xc^2 + e_yc^2 + 1)^(1/2))/(2*a_c^2*(e_xc^2 + e_yc^2)^(1/2)*(-mu/(a_c*(e_xc^2 + e_yc^2 - 1)))^(3/2)*(e_xc^2 + e_yc^2 - 1)^2) - (B_c*e_xc*mu*rho*(cos(u_c - atan2(e_yc, e_xc) + (13*sin(3*u_c - 3*atan2(e_yc, e_xc))*(e_xc^2 + e_yc^2)^(3/2))/12 + sin(u_c - atan2(e_yc, e_xc))*(2*(e_xc^2 + e_yc^2)^(1/2) - (e_xc^2 + e_yc^2)^(3/2)/4) + sin(2*u_c - 2*atan2(e_yc, e_xc))*((5*e_xc^2)/4 + (5*e_yc^2)/4)) + (e_xc^2 + e_yc^2)^(1/2))*(delta_B + 1)*(2*cos(u_c - atan2(e_yc, e_xc) + (13*sin(3*u_c - 3*atan2(e_yc, e_xc))*(e_xc^2 + e_yc^2)^(3/2))/12 + sin(u_c - atan2(e_yc, e_xc))*(2*(e_xc^2 + e_yc^2)^(1/2) - (e_xc^2 + e_yc^2)^(3/2)/4) + sin(2*u_c - 2*atan2(e_yc, e_xc))*((5*e_xc^2)/4 + (5*e_yc^2)/4))*(e_xc^2 + e_yc^2)^(1/2) + e_xc^2 + e_yc^2 + 1)^(1/2))/(a_c*(e_xc^2 + e_yc^2)^(1/2)*(-mu/(a_c*(e_xc^2 + e_yc^2 - 1)))^(1/2)*(e_xc^2 + e_yc^2 - 1)) - (B_c*e_xc*mu^2*rho*(cos(u_c - atan2(e_yc, e_xc) + (13*sin(3*u_c - 3*atan2(e_yc, e_xc))*(e_xc^2 + e_yc^2)^(3/2))/12 + sin(u_c - atan2(e_yc, e_xc))*(2*(e_xc^2 + e_yc^2)^(1/2) - (e_xc^2 + e_yc^2)^(3/2)/4) + sin(2*u_c - 2*atan2(e_yc, e_xc))*((5*e_xc^2)/4 + (5*e_yc^2)/4)) + (e_xc^2 + e_yc^2)^(1/2))*(delta_B + 1)*(2*cos(u_c - atan2(e_yc, e_xc) + (13*sin(3*u_c - 3*atan2(e_yc, e_xc))*(e_xc^2 + e_yc^2)^(3/2))/12 + sin(u_c - atan2(e_yc, e_xc))*(2*(e_xc^2 + e_yc^2)^(1/2) - (e_xc^2 + e_yc^2)^(3/2)/4) + sin(2*u_c - 2*atan2(e_yc, e_xc))*((5*e_xc^2)/4 + (5*e_yc^2)/4))*(e_xc^2 + e_yc^2)^(1/2) + e_xc^2 + e_yc^2 + 1)^(1/2))/(2*a_c^2*(e_xc^2 + e_yc^2)^(1/2)*(-mu/(a_c*(e_xc^2 + e_yc^2 - 1)))^(3/2)*(e_xc^2 + e_yc^2 - 1)^2) + (B_c*e_yc*mu*rho*sin(u_c - atan2(e_yc, e_xc) + (13*sin(3*u_c - 3*atan2(e_yc, e_xc))*(e_xc^2 + e_yc^2)^(3/2))/12 + sin(u_c - atan2(e_yc, e_xc))*(2*(e_xc^2 + e_yc^2)^(1/2) - (e_xc^2 + e_yc^2)^(3/2)/4) + sin(2*u_c - 2*atan2(e_yc, e_xc))*((5*e_xc^2)/4 + (5*e_yc^2)/4))*(delta_B + 1)*(2*cos(u_c - atan2(e_yc, e_xc) + (13*sin(3*u_c - 3*atan2(e_yc, e_xc))*(e_xc^2 + e_yc^2)^(3/2))/12 + sin(u_c - atan2(e_yc, e_xc))*(2*(e_xc^2 + e_yc^2)^(1/2) - (e_xc^2 + e_yc^2)^(3/2)/4) + sin(2*u_c - 2*atan2(e_yc, e_xc))*((5*e_xc^2)/4 + (5*e_yc^2)/4))*(e_xc^2 + e_yc^2)^(1/2) + e_xc^2 + e_yc^2 + 1)^(1/2))/(a_c*(e_xc^2 + e_yc^2)^(1/2)*(-mu/(a_c*(e_xc^2 + e_yc^2 - 1)))^(1/2)*(e_xc^2 + e_yc^2 - 1));
% A_drag(3,2) = (B_c*e_yc*mu*rho*sin(u_c - atan2(e_yc, e_xc) + (13*sin(3*u_c - 3*atan2(e_yc, e_xc))*(e_xc^2 + e_yc^2)^(3/2))/12 + sin(u_c - atan2(e_yc, e_xc))*(2*(e_xc^2 + e_yc^2)^(1/2) - (e_xc^2 + e_yc^2)^(3/2)/4) + sin(2*u_c - 2*atan2(e_yc, e_xc))*((5*e_xc^2)/4 + (5*e_yc^2)/4))^2*(delta_B + 1)*((13*cos(3*u_c - 3*atan2(e_yc, e_xc))*(e_xc^2 + e_yc^2)^(3/2))/4 + cos(u_c - atan2(e_yc, e_xc))*(2*(e_xc^2 + e_yc^2)^(1/2) - (e_xc^2 + e_yc^2)^(3/2)/4) + 2*cos(2*u_c - 2*atan2(e_yc, e_xc))*((5*e_xc^2)/4 + (5*e_yc^2)/4) + 1))/(a_c*(-mu/(a_c*(e_xc^2 + e_yc^2 - 1)))^(1/2)*(e_xc^2 + e_yc^2 - 1)*(2*cos(u_c - atan2(e_yc, e_xc) + (13*sin(3*u_c - 3*atan2(e_yc, e_xc))*(e_xc^2 + e_yc^2)^(3/2))/12 + sin(u_c - atan2(e_yc, e_xc))*(2*(e_xc^2 + e_yc^2)^(1/2) - (e_xc^2 + e_yc^2)^(3/2)/4) + sin(2*u_c - 2*atan2(e_yc, e_xc))*((5*e_xc^2)/4 + (5*e_yc^2)/4))*(e_xc^2 + e_yc^2)^(1/2) + e_xc^2 + e_yc^2 + 1)^(1/2)) - (B_c*e_xc*mu*rho*sin(u_c - atan2(e_yc, e_xc) + (13*sin(3*u_c - 3*atan2(e_yc, e_xc))*(e_xc^2 + e_yc^2)^(3/2))/12 + sin(u_c - atan2(e_yc, e_xc))*(2*(e_xc^2 + e_yc^2)^(1/2) - (e_xc^2 + e_yc^2)^(3/2)/4) + sin(2*u_c - 2*atan2(e_yc, e_xc))*((5*e_xc^2)/4 + (5*e_yc^2)/4))*(delta_B + 1)*(2*cos(u_c - atan2(e_yc, e_xc) + (13*sin(3*u_c - 3*atan2(e_yc, e_xc))*(e_xc^2 + e_yc^2)^(3/2))/12 + sin(u_c - atan2(e_yc, e_xc))*(2*(e_xc^2 + e_yc^2)^(1/2) - (e_xc^2 + e_yc^2)^(3/2)/4) + sin(2*u_c - 2*atan2(e_yc, e_xc))*((5*e_xc^2)/4 + (5*e_yc^2)/4))*(e_xc^2 + e_yc^2)^(1/2) + e_xc^2 + e_yc^2 + 1)^(1/2)*((13*cos(3*u_c - 3*atan2(e_yc, e_xc))*(e_xc^2 + e_yc^2)^(3/2))/4 + cos(u_c - atan2(e_yc, e_xc))*(2*(e_xc^2 + e_yc^2)^(1/2) - (e_xc^2 + e_yc^2)^(3/2)/4) + 2*cos(2*u_c - 2*atan2(e_yc, e_xc))*((5*e_xc^2)/4 + (5*e_yc^2)/4) + 1))/(a_c*(e_xc^2 + e_yc^2)^(1/2)*(-mu/(a_c*(e_xc^2 + e_yc^2 - 1)))^(1/2)*(e_xc^2 + e_yc^2 - 1)) - (B_c*e_xc*mu*rho*sin(u_c - atan2(e_yc, e_xc) + (13*sin(3*u_c - 3*atan2(e_yc, e_xc))*(e_xc^2 + e_yc^2)^(3/2))/12 + sin(u_c - atan2(e_yc, e_xc))*(2*(e_xc^2 + e_yc^2)^(1/2) - (e_xc^2 + e_yc^2)^(3/2)/4) + sin(2*u_c - 2*atan2(e_yc, e_xc))*((5*e_xc^2)/4 + (5*e_yc^2)/4))*(cos(u_c - atan2(e_yc, e_xc) + (13*sin(3*u_c - 3*atan2(e_yc, e_xc))*(e_xc^2 + e_yc^2)^(3/2))/12 + sin(u_c - atan2(e_yc, e_xc))*(2*(e_xc^2 + e_yc^2)^(1/2) - (e_xc^2 + e_yc^2)^(3/2)/4) + sin(2*u_c - 2*atan2(e_yc, e_xc))*((5*e_xc^2)/4 + (5*e_yc^2)/4)) + (e_xc^2 + e_yc^2)^(1/2))*(delta_B + 1)*((13*cos(3*u_c - 3*atan2(e_yc, e_xc))*(e_xc^2 + e_yc^2)^(3/2))/4 + cos(u_c - atan2(e_yc, e_xc))*(2*(e_xc^2 + e_yc^2)^(1/2) - (e_xc^2 + e_yc^2)^(3/2)/4) + 2*cos(2*u_c - 2*atan2(e_yc, e_xc))*((5*e_xc^2)/4 + (5*e_yc^2)/4) + 1))/(a_c*(-mu/(a_c*(e_xc^2 + e_yc^2 - 1)))^(1/2)*(e_xc^2 + e_yc^2 - 1)*(2*cos(u_c - atan2(e_yc, e_xc) + (13*sin(3*u_c - 3*atan2(e_yc, e_xc))*(e_xc^2 + e_yc^2)^(3/2))/12 + sin(u_c - atan2(e_yc, e_xc))*(2*(e_xc^2 + e_yc^2)^(1/2) - (e_xc^2 + e_yc^2)^(3/2)/4) + sin(2*u_c - 2*atan2(e_yc, e_xc))*((5*e_xc^2)/4 + (5*e_yc^2)/4))*(e_xc^2 + e_yc^2)^(1/2) + e_xc^2 + e_yc^2 + 1)^(1/2)) - (B_c*e_yc*mu*rho*cos(u_c - atan2(e_yc, e_xc) + (13*sin(3*u_c - 3*atan2(e_yc, e_xc))*(e_xc^2 + e_yc^2)^(3/2))/12 + sin(u_c - atan2(e_yc, e_xc))*(2*(e_xc^2 + e_yc^2)^(1/2) - (e_xc^2 + e_yc^2)^(3/2)/4) + sin(2*u_c - 2*atan2(e_yc, e_xc))*((5*e_xc^2)/4 + (5*e_yc^2)/4))*(delta_B + 1)*(2*cos(u_c - atan2(e_yc, e_xc) + (13*sin(3*u_c - 3*atan2(e_yc, e_xc))*(e_xc^2 + e_yc^2)^(3/2))/12 + sin(u_c - atan2(e_yc, e_xc))*(2*(e_xc^2 + e_yc^2)^(1/2) - (e_xc^2 + e_yc^2)^(3/2)/4) + sin(2*u_c - 2*atan2(e_yc, e_xc))*((5*e_xc^2)/4 + (5*e_yc^2)/4))*(e_xc^2 + e_yc^2)^(1/2) + e_xc^2 + e_yc^2 + 1)^(1/2)*((13*cos(3*u_c - 3*atan2(e_yc, e_xc))*(e_xc^2 + e_yc^2)^(3/2))/4 + cos(u_c - atan2(e_yc, e_xc))*(2*(e_xc^2 + e_yc^2)^(1/2) - (e_xc^2 + e_yc^2)^(3/2)/4) + 2*cos(2*u_c - 2*atan2(e_yc, e_xc))*((5*e_xc^2)/4 + (5*e_yc^2)/4) + 1))/(a_c*(e_xc^2 + e_yc^2)^(1/2)*(-mu/(a_c*(e_xc^2 + e_yc^2 - 1)))^(1/2)*(e_xc^2 + e_yc^2 - 1));
% A_drag(3,3) = (B_c*mu*rho*(cos(u_c - atan2(e_yc, e_xc) + (13*sin(3*u_c - 3*atan2(e_yc, e_xc))*(e_xc^2 + e_yc^2)^(3/2))/12 + sin(u_c - atan2(e_yc, e_xc))*(2*(e_xc^2 + e_yc^2)^(1/2) - (e_xc^2 + e_yc^2)^(3/2)/4) + sin(2*u_c - 2*atan2(e_yc, e_xc))*((5*e_xc^2)/4 + (5*e_yc^2)/4)) + (e_xc^2 + e_yc^2)^(1/2))*(delta_B + 1)*(2*cos(u_c - atan2(e_yc, e_xc) + (13*sin(3*u_c - 3*atan2(e_yc, e_xc))*(e_xc^2 + e_yc^2)^(3/2))/12 + sin(u_c - atan2(e_yc, e_xc))*(2*(e_xc^2 + e_yc^2)^(1/2) - (e_xc^2 + e_yc^2)^(3/2)/4) + sin(2*u_c - 2*atan2(e_yc, e_xc))*((5*e_xc^2)/4 + (5*e_yc^2)/4))*(e_xc^2 + e_yc^2)^(1/2) + e_xc^2 + e_yc^2 + 1)^(1/2))/(a_c*(e_xc^2 + e_yc^2)^(1/2)*(-mu/(a_c*(e_xc^2 + e_yc^2 - 1)))^(1/2)*(e_xc^2 + e_yc^2 - 1)) - (2*B_c*e_xc^2*mu*rho*(cos(u_c - atan2(e_yc, e_xc) + (13*sin(3*u_c - 3*atan2(e_yc, e_xc))*(e_xc^2 + e_yc^2)^(3/2))/12 + sin(u_c - atan2(e_yc, e_xc))*(2*(e_xc^2 + e_yc^2)^(1/2) - (e_xc^2 + e_yc^2)^(3/2)/4) + sin(2*u_c - 2*atan2(e_yc, e_xc))*((5*e_xc^2)/4 + (5*e_yc^2)/4)) + (e_xc^2 + e_yc^2)^(1/2))*(delta_B + 1)*(2*cos(u_c - atan2(e_yc, e_xc) + (13*sin(3*u_c - 3*atan2(e_yc, e_xc))*(e_xc^2 + e_yc^2)^(3/2))/12 + sin(u_c - atan2(e_yc, e_xc))*(2*(e_xc^2 + e_yc^2)^(1/2) - (e_xc^2 + e_yc^2)^(3/2)/4) + sin(2*u_c - 2*atan2(e_yc, e_xc))*((5*e_xc^2)/4 + (5*e_yc^2)/4))*(e_xc^2 + e_yc^2)^(1/2) + e_xc^2 + e_yc^2 + 1)^(1/2))/(a_c*(e_xc^2 + e_yc^2)^(1/2)*(-mu/(a_c*(e_xc^2 + e_yc^2 - 1)))^(1/2)*(e_xc^2 + e_yc^2 - 1)^2) - (B_c*e_xc^2*mu*rho*(cos(u_c - atan2(e_yc, e_xc) + (13*sin(3*u_c - 3*atan2(e_yc, e_xc))*(e_xc^2 + e_yc^2)^(3/2))/12 + sin(u_c - atan2(e_yc, e_xc))*(2*(e_xc^2 + e_yc^2)^(1/2) - (e_xc^2 + e_yc^2)^(3/2)/4) + sin(2*u_c - 2*atan2(e_yc, e_xc))*((5*e_xc^2)/4 + (5*e_yc^2)/4)) + (e_xc^2 + e_yc^2)^(1/2))*(delta_B + 1)*(2*cos(u_c - atan2(e_yc, e_xc) + (13*sin(3*u_c - 3*atan2(e_yc, e_xc))*(e_xc^2 + e_yc^2)^(3/2))/12 + sin(u_c - atan2(e_yc, e_xc))*(2*(e_xc^2 + e_yc^2)^(1/2) - (e_xc^2 + e_yc^2)^(3/2)/4) + sin(2*u_c - 2*atan2(e_yc, e_xc))*((5*e_xc^2)/4 + (5*e_yc^2)/4))*(e_xc^2 + e_yc^2)^(1/2) + e_xc^2 + e_yc^2 + 1)^(1/2))/(a_c*(e_xc^2 + e_yc^2)^(3/2)*(-mu/(a_c*(e_xc^2 + e_yc^2 - 1)))^(1/2)*(e_xc^2 + e_yc^2 - 1)) + (B_c*e_xc*mu*rho*(delta_B + 1)*(e_xc/(e_xc^2 + e_yc^2)^(1/2) - sin(u_c - atan2(e_yc, e_xc) + (13*sin(3*u_c - 3*atan2(e_yc, e_xc))*(e_xc^2 + e_yc^2)^(3/2))/12 + sin(u_c - atan2(e_yc, e_xc))*(2*(e_xc^2 + e_yc^2)^(1/2) - (e_xc^2 + e_yc^2)^(3/2)/4) + sin(2*u_c - 2*atan2(e_yc, e_xc))*((5*e_xc^2)/4 + (5*e_yc^2)/4))*(e_yc/(e_xc^2 + e_yc^2) + sin(u_c - atan2(e_yc, e_xc))*((2*e_xc)/(e_xc^2 + e_yc^2)^(1/2) - (3*e_xc*(e_xc^2 + e_yc^2)^(1/2))/4) + (5*e_xc*sin(2*u_c - 2*atan2(e_yc, e_xc)))/2 + (13*e_yc*cos(3*u_c - 3*atan2(e_yc, e_xc))*(e_xc^2 + e_yc^2)^(1/2))/4 + (13*e_xc*sin(3*u_c - 3*atan2(e_yc, e_xc))*(e_xc^2 + e_yc^2)^(1/2))/4 + (e_yc*cos(u_c - atan2(e_yc, e_xc))*(2*(e_xc^2 + e_yc^2)^(1/2) - (e_xc^2 + e_yc^2)^(3/2)/4))/(e_xc^2 + e_yc^2) + (2*e_yc*cos(2*u_c - 2*atan2(e_yc, e_xc))*((5*e_xc^2)/4 + (5*e_yc^2)/4))/(e_xc^2 + e_yc^2)))*(2*cos(u_c - atan2(e_yc, e_xc) + (13*sin(3*u_c - 3*atan2(e_yc, e_xc))*(e_xc^2 + e_yc^2)^(3/2))/12 + sin(u_c - atan2(e_yc, e_xc))*(2*(e_xc^2 + e_yc^2)^(1/2) - (e_xc^2 + e_yc^2)^(3/2)/4) + sin(2*u_c - 2*atan2(e_yc, e_xc))*((5*e_xc^2)/4 + (5*e_yc^2)/4))*(e_xc^2 + e_yc^2)^(1/2) + e_xc^2 + e_yc^2 + 1)^(1/2))/(a_c*(e_xc^2 + e_yc^2)^(1/2)*(-mu/(a_c*(e_xc^2 + e_yc^2 - 1)))^(1/2)*(e_xc^2 + e_yc^2 - 1)) - (B_c*e_xc^2*mu^2*rho*(cos(u_c - atan2(e_yc, e_xc) + (13*sin(3*u_c - 3*atan2(e_yc, e_xc))*(e_xc^2 + e_yc^2)^(3/2))/12 + sin(u_c - atan2(e_yc, e_xc))*(2*(e_xc^2 + e_yc^2)^(1/2) - (e_xc^2 + e_yc^2)^(3/2)/4) + sin(2*u_c - 2*atan2(e_yc, e_xc))*((5*e_xc^2)/4 + (5*e_yc^2)/4)) + (e_xc^2 + e_yc^2)^(1/2))*(delta_B + 1)*(2*cos(u_c - atan2(e_yc, e_xc) + (13*sin(3*u_c - 3*atan2(e_yc, e_xc))*(e_xc^2 + e_yc^2)^(3/2))/12 + sin(u_c - atan2(e_yc, e_xc))*(2*(e_xc^2 + e_yc^2)^(1/2) - (e_xc^2 + e_yc^2)^(3/2)/4) + sin(2*u_c - 2*atan2(e_yc, e_xc))*((5*e_xc^2)/4 + (5*e_yc^2)/4))*(e_xc^2 + e_yc^2)^(1/2) + e_xc^2 + e_yc^2 + 1)^(1/2))/(a_c^2*(e_xc^2 + e_yc^2)^(1/2)*(-mu/(a_c*(e_xc^2 + e_yc^2 - 1)))^(3/2)*(e_xc^2 + e_yc^2 - 1)^3) + (2*B_c*e_xc*e_yc*mu*rho*sin(u_c - atan2(e_yc, e_xc) + (13*sin(3*u_c - 3*atan2(e_yc, e_xc))*(e_xc^2 + e_yc^2)^(3/2))/12 + sin(u_c - atan2(e_yc, e_xc))*(2*(e_xc^2 + e_yc^2)^(1/2) - (e_xc^2 + e_yc^2)^(3/2)/4) + sin(2*u_c - 2*atan2(e_yc, e_xc))*((5*e_xc^2)/4 + (5*e_yc^2)/4))*(delta_B + 1)*(2*cos(u_c - atan2(e_yc, e_xc) + (13*sin(3*u_c - 3*atan2(e_yc, e_xc))*(e_xc^2 + e_yc^2)^(3/2))/12 + sin(u_c - atan2(e_yc, e_xc))*(2*(e_xc^2 + e_yc^2)^(1/2) - (e_xc^2 + e_yc^2)^(3/2)/4) + sin(2*u_c - 2*atan2(e_yc, e_xc))*((5*e_xc^2)/4 + (5*e_yc^2)/4))*(e_xc^2 + e_yc^2)^(1/2) + e_xc^2 + e_yc^2 + 1)^(1/2))/(a_c*(e_xc^2 + e_yc^2)^(1/2)*(-mu/(a_c*(e_xc^2 + e_yc^2 - 1)))^(1/2)*(e_xc^2 + e_yc^2 - 1)^2) + (B_c*e_xc*e_yc*mu*rho*sin(u_c - atan2(e_yc, e_xc) + (13*sin(3*u_c - 3*atan2(e_yc, e_xc))*(e_xc^2 + e_yc^2)^(3/2))/12 + sin(u_c - atan2(e_yc, e_xc))*(2*(e_xc^2 + e_yc^2)^(1/2) - (e_xc^2 + e_yc^2)^(3/2)/4) + sin(2*u_c - 2*atan2(e_yc, e_xc))*((5*e_xc^2)/4 + (5*e_yc^2)/4))*(delta_B + 1)*(2*cos(u_c - atan2(e_yc, e_xc) + (13*sin(3*u_c - 3*atan2(e_yc, e_xc))*(e_xc^2 + e_yc^2)^(3/2))/12 + sin(u_c - atan2(e_yc, e_xc))*(2*(e_xc^2 + e_yc^2)^(1/2) - (e_xc^2 + e_yc^2)^(3/2)/4) + sin(2*u_c - 2*atan2(e_yc, e_xc))*((5*e_xc^2)/4 + (5*e_yc^2)/4))*(e_xc^2 + e_yc^2)^(1/2) + e_xc^2 + e_yc^2 + 1)^(1/2))/(a_c*(e_xc^2 + e_yc^2)^(3/2)*(-mu/(a_c*(e_xc^2 + e_yc^2 - 1)))^(1/2)*(e_xc^2 + e_yc^2 - 1)) - (B_c*e_yc*mu*rho*sin(u_c - atan2(e_yc, e_xc) + (13*sin(3*u_c - 3*atan2(e_yc, e_xc))*(e_xc^2 + e_yc^2)^(3/2))/12 + sin(u_c - atan2(e_yc, e_xc))*(2*(e_xc^2 + e_yc^2)^(1/2) - (e_xc^2 + e_yc^2)^(3/2)/4) + sin(2*u_c - 2*atan2(e_yc, e_xc))*((5*e_xc^2)/4 + (5*e_yc^2)/4))*(delta_B + 1)*(2*e_xc + (2*e_xc*cos(u_c - atan2(e_yc, e_xc) + (13*sin(3*u_c - 3*atan2(e_yc, e_xc))*(e_xc^2 + e_yc^2)^(3/2))/12 + sin(u_c - atan2(e_yc, e_xc))*(2*(e_xc^2 + e_yc^2)^(1/2) - (e_xc^2 + e_yc^2)^(3/2)/4) + sin(2*u_c - 2*atan2(e_yc, e_xc))*((5*e_xc^2)/4 + (5*e_yc^2)/4)))/(e_xc^2 + e_yc^2)^(1/2) - 2*sin(u_c - atan2(e_yc, e_xc) + (13*sin(3*u_c - 3*atan2(e_yc, e_xc))*(e_xc^2 + e_yc^2)^(3/2))/12 + sin(u_c - atan2(e_yc, e_xc))*(2*(e_xc^2 + e_yc^2)^(1/2) - (e_xc^2 + e_yc^2)^(3/2)/4) + sin(2*u_c - 2*atan2(e_yc, e_xc))*((5*e_xc^2)/4 + (5*e_yc^2)/4))*(e_xc^2 + e_yc^2)^(1/2)*(e_yc/(e_xc^2 + e_yc^2) + sin(u_c - atan2(e_yc, e_xc))*((2*e_xc)/(e_xc^2 + e_yc^2)^(1/2) - (3*e_xc*(e_xc^2 + e_yc^2)^(1/2))/4) + (5*e_xc*sin(2*u_c - 2*atan2(e_yc, e_xc)))/2 + (13*e_yc*cos(3*u_c - 3*atan2(e_yc, e_xc))*(e_xc^2 + e_yc^2)^(1/2))/4 + (13*e_xc*sin(3*u_c - 3*atan2(e_yc, e_xc))*(e_xc^2 + e_yc^2)^(1/2))/4 + (e_yc*cos(u_c - atan2(e_yc, e_xc))*(2*(e_xc^2 + e_yc^2)^(1/2) - (e_xc^2 + e_yc^2)^(3/2)/4))/(e_xc^2 + e_yc^2) + (2*e_yc*cos(2*u_c - 2*atan2(e_yc, e_xc))*((5*e_xc^2)/4 + (5*e_yc^2)/4))/(e_xc^2 + e_yc^2))))/(2*a_c*(e_xc^2 + e_yc^2)^(1/2)*(-mu/(a_c*(e_xc^2 + e_yc^2 - 1)))^(1/2)*(e_xc^2 + e_yc^2 - 1)*(2*cos(u_c - atan2(e_yc, e_xc) + (13*sin(3*u_c - 3*atan2(e_yc, e_xc))*(e_xc^2 + e_yc^2)^(3/2))/12 + sin(u_c - atan2(e_yc, e_xc))*(2*(e_xc^2 + e_yc^2)^(1/2) - (e_xc^2 + e_yc^2)^(3/2)/4) + sin(2*u_c - 2*atan2(e_yc, e_xc))*((5*e_xc^2)/4 + (5*e_yc^2)/4))*(e_xc^2 + e_yc^2)^(1/2) + e_xc^2 + e_yc^2 + 1)^(1/2)) + (B_c*e_xc*e_yc*mu^2*rho*sin(u_c - atan2(e_yc, e_xc) + (13*sin(3*u_c - 3*atan2(e_yc, e_xc))*(e_xc^2 + e_yc^2)^(3/2))/12 + sin(u_c - atan2(e_yc, e_xc))*(2*(e_xc^2 + e_yc^2)^(1/2) - (e_xc^2 + e_yc^2)^(3/2)/4) + sin(2*u_c - 2*atan2(e_yc, e_xc))*((5*e_xc^2)/4 + (5*e_yc^2)/4))*(delta_B + 1)*(2*cos(u_c - atan2(e_yc, e_xc) + (13*sin(3*u_c - 3*atan2(e_yc, e_xc))*(e_xc^2 + e_yc^2)^(3/2))/12 + sin(u_c - atan2(e_yc, e_xc))*(2*(e_xc^2 + e_yc^2)^(1/2) - (e_xc^2 + e_yc^2)^(3/2)/4) + sin(2*u_c - 2*atan2(e_yc, e_xc))*((5*e_xc^2)/4 + (5*e_yc^2)/4))*(e_xc^2 + e_yc^2)^(1/2) + e_xc^2 + e_yc^2 + 1)^(1/2))/(a_c^2*(e_xc^2 + e_yc^2)^(1/2)*(-mu/(a_c*(e_xc^2 + e_yc^2 - 1)))^(3/2)*(e_xc^2 + e_yc^2 - 1)^3) - (B_c*e_yc*mu*rho*cos(u_c - atan2(e_yc, e_xc) + (13*sin(3*u_c - 3*atan2(e_yc, e_xc))*(e_xc^2 + e_yc^2)^(3/2))/12 + sin(u_c - atan2(e_yc, e_xc))*(2*(e_xc^2 + e_yc^2)^(1/2) - (e_xc^2 + e_yc^2)^(3/2)/4) + sin(2*u_c - 2*atan2(e_yc, e_xc))*((5*e_xc^2)/4 + (5*e_yc^2)/4))*(delta_B + 1)*(2*cos(u_c - atan2(e_yc, e_xc) + (13*sin(3*u_c - 3*atan2(e_yc, e_xc))*(e_xc^2 + e_yc^2)^(3/2))/12 + sin(u_c - atan2(e_yc, e_xc))*(2*(e_xc^2 + e_yc^2)^(1/2) - (e_xc^2 + e_yc^2)^(3/2)/4) + sin(2*u_c - 2*atan2(e_yc, e_xc))*((5*e_xc^2)/4 + (5*e_yc^2)/4))*(e_xc^2 + e_yc^2)^(1/2) + e_xc^2 + e_yc^2 + 1)^(1/2)*(e_yc/(e_xc^2 + e_yc^2) + sin(u_c - atan2(e_yc, e_xc))*((2*e_xc)/(e_xc^2 + e_yc^2)^(1/2) - (3*e_xc*(e_xc^2 + e_yc^2)^(1/2))/4) + (5*e_xc*sin(2*u_c - 2*atan2(e_yc, e_xc)))/2 + (13*e_yc*cos(3*u_c - 3*atan2(e_yc, e_xc))*(e_xc^2 + e_yc^2)^(1/2))/4 + (13*e_xc*sin(3*u_c - 3*atan2(e_yc, e_xc))*(e_xc^2 + e_yc^2)^(1/2))/4 + (e_yc*cos(u_c - atan2(e_yc, e_xc))*(2*(e_xc^2 + e_yc^2)^(1/2) - (e_xc^2 + e_yc^2)^(3/2)/4))/(e_xc^2 + e_yc^2) + (2*e_yc*cos(2*u_c - 2*atan2(e_yc, e_xc))*((5*e_xc^2)/4 + (5*e_yc^2)/4))/(e_xc^2 + e_yc^2)))/(a_c*(e_xc^2 + e_yc^2)^(1/2)*(-mu/(a_c*(e_xc^2 + e_yc^2 - 1)))^(1/2)*(e_xc^2 + e_yc^2 - 1)) + (B_c*e_xc*mu*rho*(cos(u_c - atan2(e_yc, e_xc) + (13*sin(3*u_c - 3*atan2(e_yc, e_xc))*(e_xc^2 + e_yc^2)^(3/2))/12 + sin(u_c - atan2(e_yc, e_xc))*(2*(e_xc^2 + e_yc^2)^(1/2) - (e_xc^2 + e_yc^2)^(3/2)/4) + sin(2*u_c - 2*atan2(e_yc, e_xc))*((5*e_xc^2)/4 + (5*e_yc^2)/4)) + (e_xc^2 + e_yc^2)^(1/2))*(delta_B + 1)*(2*e_xc + (2*e_xc*cos(u_c - atan2(e_yc, e_xc) + (13*sin(3*u_c - 3*atan2(e_yc, e_xc))*(e_xc^2 + e_yc^2)^(3/2))/12 + sin(u_c - atan2(e_yc, e_xc))*(2*(e_xc^2 + e_yc^2)^(1/2) - (e_xc^2 + e_yc^2)^(3/2)/4) + sin(2*u_c - 2*atan2(e_yc, e_xc))*((5*e_xc^2)/4 + (5*e_yc^2)/4)))/(e_xc^2 + e_yc^2)^(1/2) - 2*sin(u_c - atan2(e_yc, e_xc) + (13*sin(3*u_c - 3*atan2(e_yc, e_xc))*(e_xc^2 + e_yc^2)^(3/2))/12 + sin(u_c - atan2(e_yc, e_xc))*(2*(e_xc^2 + e_yc^2)^(1/2) - (e_xc^2 + e_yc^2)^(3/2)/4) + sin(2*u_c - 2*atan2(e_yc, e_xc))*((5*e_xc^2)/4 + (5*e_yc^2)/4))*(e_xc^2 + e_yc^2)^(1/2)*(e_yc/(e_xc^2 + e_yc^2) + sin(u_c - atan2(e_yc, e_xc))*((2*e_xc)/(e_xc^2 + e_yc^2)^(1/2) - (3*e_xc*(e_xc^2 + e_yc^2)^(1/2))/4) + (5*e_xc*sin(2*u_c - 2*atan2(e_yc, e_xc)))/2 + (13*e_yc*cos(3*u_c - 3*atan2(e_yc, e_xc))*(e_xc^2 + e_yc^2)^(1/2))/4 + (13*e_xc*sin(3*u_c - 3*atan2(e_yc, e_xc))*(e_xc^2 + e_yc^2)^(1/2))/4 + (e_yc*cos(u_c - atan2(e_yc, e_xc))*(2*(e_xc^2 + e_yc^2)^(1/2) - (e_xc^2 + e_yc^2)^(3/2)/4))/(e_xc^2 + e_yc^2) + (2*e_yc*cos(2*u_c - 2*atan2(e_yc, e_xc))*((5*e_xc^2)/4 + (5*e_yc^2)/4))/(e_xc^2 + e_yc^2))))/(2*a_c*(e_xc^2 + e_yc^2)^(1/2)*(-mu/(a_c*(e_xc^2 + e_yc^2 - 1)))^(1/2)*(e_xc^2 + e_yc^2 - 1)*(2*cos(u_c - atan2(e_yc, e_xc) + (13*sin(3*u_c - 3*atan2(e_yc, e_xc))*(e_xc^2 + e_yc^2)^(3/2))/12 + sin(u_c - atan2(e_yc, e_xc))*(2*(e_xc^2 + e_yc^2)^(1/2) - (e_xc^2 + e_yc^2)^(3/2)/4) + sin(2*u_c - 2*atan2(e_yc, e_xc))*((5*e_xc^2)/4 + (5*e_yc^2)/4))*(e_xc^2 + e_yc^2)^(1/2) + e_xc^2 + e_yc^2 + 1)^(1/2));
% A_drag(3,4) = (2*B_c*e_yc^2*mu*rho*sin(u_c - atan2(e_yc, e_xc) + (13*sin(3*u_c - 3*atan2(e_yc, e_xc))*(e_xc^2 + e_yc^2)^(3/2))/12 + sin(u_c - atan2(e_yc, e_xc))*(2*(e_xc^2 + e_yc^2)^(1/2) - (e_xc^2 + e_yc^2)^(3/2)/4) + sin(2*u_c - 2*atan2(e_yc, e_xc))*((5*e_xc^2)/4 + (5*e_yc^2)/4))*(delta_B + 1)*(2*cos(u_c - atan2(e_yc, e_xc) + (13*sin(3*u_c - 3*atan2(e_yc, e_xc))*(e_xc^2 + e_yc^2)^(3/2))/12 + sin(u_c - atan2(e_yc, e_xc))*(2*(e_xc^2 + e_yc^2)^(1/2) - (e_xc^2 + e_yc^2)^(3/2)/4) + sin(2*u_c - 2*atan2(e_yc, e_xc))*((5*e_xc^2)/4 + (5*e_yc^2)/4))*(e_xc^2 + e_yc^2)^(1/2) + e_xc^2 + e_yc^2 + 1)^(1/2))/(a_c*(e_xc^2 + e_yc^2)^(1/2)*(-mu/(a_c*(e_xc^2 + e_yc^2 - 1)))^(1/2)*(e_xc^2 + e_yc^2 - 1)^2) - (B_c*mu*rho*sin(u_c - atan2(e_yc, e_xc) + (13*sin(3*u_c - 3*atan2(e_yc, e_xc))*(e_xc^2 + e_yc^2)^(3/2))/12 + sin(u_c - atan2(e_yc, e_xc))*(2*(e_xc^2 + e_yc^2)^(1/2) - (e_xc^2 + e_yc^2)^(3/2)/4) + sin(2*u_c - 2*atan2(e_yc, e_xc))*((5*e_xc^2)/4 + (5*e_yc^2)/4))*(delta_B + 1)*(2*cos(u_c - atan2(e_yc, e_xc) + (13*sin(3*u_c - 3*atan2(e_yc, e_xc))*(e_xc^2 + e_yc^2)^(3/2))/12 + sin(u_c - atan2(e_yc, e_xc))*(2*(e_xc^2 + e_yc^2)^(1/2) - (e_xc^2 + e_yc^2)^(3/2)/4) + sin(2*u_c - 2*atan2(e_yc, e_xc))*((5*e_xc^2)/4 + (5*e_yc^2)/4))*(e_xc^2 + e_yc^2)^(1/2) + e_xc^2 + e_yc^2 + 1)^(1/2))/(a_c*(e_xc^2 + e_yc^2)^(1/2)*(-mu/(a_c*(e_xc^2 + e_yc^2 - 1)))^(1/2)*(e_xc^2 + e_yc^2 - 1)) + (B_c*e_yc^2*mu*rho*sin(u_c - atan2(e_yc, e_xc) + (13*sin(3*u_c - 3*atan2(e_yc, e_xc))*(e_xc^2 + e_yc^2)^(3/2))/12 + sin(u_c - atan2(e_yc, e_xc))*(2*(e_xc^2 + e_yc^2)^(1/2) - (e_xc^2 + e_yc^2)^(3/2)/4) + sin(2*u_c - 2*atan2(e_yc, e_xc))*((5*e_xc^2)/4 + (5*e_yc^2)/4))*(delta_B + 1)*(2*cos(u_c - atan2(e_yc, e_xc) + (13*sin(3*u_c - 3*atan2(e_yc, e_xc))*(e_xc^2 + e_yc^2)^(3/2))/12 + sin(u_c - atan2(e_yc, e_xc))*(2*(e_xc^2 + e_yc^2)^(1/2) - (e_xc^2 + e_yc^2)^(3/2)/4) + sin(2*u_c - 2*atan2(e_yc, e_xc))*((5*e_xc^2)/4 + (5*e_yc^2)/4))*(e_xc^2 + e_yc^2)^(1/2) + e_xc^2 + e_yc^2 + 1)^(1/2))/(a_c*(e_xc^2 + e_yc^2)^(3/2)*(-mu/(a_c*(e_xc^2 + e_yc^2 - 1)))^(1/2)*(e_xc^2 + e_yc^2 - 1)) + (B_c*e_yc^2*mu^2*rho*sin(u_c - atan2(e_yc, e_xc) + (13*sin(3*u_c - 3*atan2(e_yc, e_xc))*(e_xc^2 + e_yc^2)^(3/2))/12 + sin(u_c - atan2(e_yc, e_xc))*(2*(e_xc^2 + e_yc^2)^(1/2) - (e_xc^2 + e_yc^2)^(3/2)/4) + sin(2*u_c - 2*atan2(e_yc, e_xc))*((5*e_xc^2)/4 + (5*e_yc^2)/4))*(delta_B + 1)*(2*cos(u_c - atan2(e_yc, e_xc) + (13*sin(3*u_c - 3*atan2(e_yc, e_xc))*(e_xc^2 + e_yc^2)^(3/2))/12 + sin(u_c - atan2(e_yc, e_xc))*(2*(e_xc^2 + e_yc^2)^(1/2) - (e_xc^2 + e_yc^2)^(3/2)/4) + sin(2*u_c - 2*atan2(e_yc, e_xc))*((5*e_xc^2)/4 + (5*e_yc^2)/4))*(e_xc^2 + e_yc^2)^(1/2) + e_xc^2 + e_yc^2 + 1)^(1/2))/(a_c^2*(e_xc^2 + e_yc^2)^(1/2)*(-mu/(a_c*(e_xc^2 + e_yc^2 - 1)))^(3/2)*(e_xc^2 + e_yc^2 - 1)^3) + (B_c*e_xc*mu*rho*(delta_B + 1)*(e_yc/(e_xc^2 + e_yc^2)^(1/2) + sin(u_c - atan2(e_yc, e_xc) + (13*sin(3*u_c - 3*atan2(e_yc, e_xc))*(e_xc^2 + e_yc^2)^(3/2))/12 + sin(u_c - atan2(e_yc, e_xc))*(2*(e_xc^2 + e_yc^2)^(1/2) - (e_xc^2 + e_yc^2)^(3/2)/4) + sin(2*u_c - 2*atan2(e_yc, e_xc))*((5*e_xc^2)/4 + (5*e_yc^2)/4))*(e_xc/(e_xc^2 + e_yc^2) - sin(u_c - atan2(e_yc, e_xc))*((2*e_yc)/(e_xc^2 + e_yc^2)^(1/2) - (3*e_yc*(e_xc^2 + e_yc^2)^(1/2))/4) - (5*e_yc*sin(2*u_c - 2*atan2(e_yc, e_xc)))/2 + (13*e_xc*cos(3*u_c - 3*atan2(e_yc, e_xc))*(e_xc^2 + e_yc^2)^(1/2))/4 - (13*e_yc*sin(3*u_c - 3*atan2(e_yc, e_xc))*(e_xc^2 + e_yc^2)^(1/2))/4 + (e_xc*cos(u_c - atan2(e_yc, e_xc))*(2*(e_xc^2 + e_yc^2)^(1/2) - (e_xc^2 + e_yc^2)^(3/2)/4))/(e_xc^2 + e_yc^2) + (2*e_xc*cos(2*u_c - 2*atan2(e_yc, e_xc))*((5*e_xc^2)/4 + (5*e_yc^2)/4))/(e_xc^2 + e_yc^2)))*(2*cos(u_c - atan2(e_yc, e_xc) + (13*sin(3*u_c - 3*atan2(e_yc, e_xc))*(e_xc^2 + e_yc^2)^(3/2))/12 + sin(u_c - atan2(e_yc, e_xc))*(2*(e_xc^2 + e_yc^2)^(1/2) - (e_xc^2 + e_yc^2)^(3/2)/4) + sin(2*u_c - 2*atan2(e_yc, e_xc))*((5*e_xc^2)/4 + (5*e_yc^2)/4))*(e_xc^2 + e_yc^2)^(1/2) + e_xc^2 + e_yc^2 + 1)^(1/2))/(a_c*(e_xc^2 + e_yc^2)^(1/2)*(-mu/(a_c*(e_xc^2 + e_yc^2 - 1)))^(1/2)*(e_xc^2 + e_yc^2 - 1)) - (B_c*e_yc*mu*rho*sin(u_c - atan2(e_yc, e_xc) + (13*sin(3*u_c - 3*atan2(e_yc, e_xc))*(e_xc^2 + e_yc^2)^(3/2))/12 + sin(u_c - atan2(e_yc, e_xc))*(2*(e_xc^2 + e_yc^2)^(1/2) - (e_xc^2 + e_yc^2)^(3/2)/4) + sin(2*u_c - 2*atan2(e_yc, e_xc))*((5*e_xc^2)/4 + (5*e_yc^2)/4))*(delta_B + 1)*(2*e_yc + (2*e_yc*cos(u_c - atan2(e_yc, e_xc) + (13*sin(3*u_c - 3*atan2(e_yc, e_xc))*(e_xc^2 + e_yc^2)^(3/2))/12 + sin(u_c - atan2(e_yc, e_xc))*(2*(e_xc^2 + e_yc^2)^(1/2) - (e_xc^2 + e_yc^2)^(3/2)/4) + sin(2*u_c - 2*atan2(e_yc, e_xc))*((5*e_xc^2)/4 + (5*e_yc^2)/4)))/(e_xc^2 + e_yc^2)^(1/2) + 2*sin(u_c - atan2(e_yc, e_xc) + (13*sin(3*u_c - 3*atan2(e_yc, e_xc))*(e_xc^2 + e_yc^2)^(3/2))/12 + sin(u_c - atan2(e_yc, e_xc))*(2*(e_xc^2 + e_yc^2)^(1/2) - (e_xc^2 + e_yc^2)^(3/2)/4) + sin(2*u_c - 2*atan2(e_yc, e_xc))*((5*e_xc^2)/4 + (5*e_yc^2)/4))*(e_xc^2 + e_yc^2)^(1/2)*(e_xc/(e_xc^2 + e_yc^2) - sin(u_c - atan2(e_yc, e_xc))*((2*e_yc)/(e_xc^2 + e_yc^2)^(1/2) - (3*e_yc*(e_xc^2 + e_yc^2)^(1/2))/4) - (5*e_yc*sin(2*u_c - 2*atan2(e_yc, e_xc)))/2 + (13*e_xc*cos(3*u_c - 3*atan2(e_yc, e_xc))*(e_xc^2 + e_yc^2)^(1/2))/4 - (13*e_yc*sin(3*u_c - 3*atan2(e_yc, e_xc))*(e_xc^2 + e_yc^2)^(1/2))/4 + (e_xc*cos(u_c - atan2(e_yc, e_xc))*(2*(e_xc^2 + e_yc^2)^(1/2) - (e_xc^2 + e_yc^2)^(3/2)/4))/(e_xc^2 + e_yc^2) + (2*e_xc*cos(2*u_c - 2*atan2(e_yc, e_xc))*((5*e_xc^2)/4 + (5*e_yc^2)/4))/(e_xc^2 + e_yc^2))))/(2*a_c*(e_xc^2 + e_yc^2)^(1/2)*(-mu/(a_c*(e_xc^2 + e_yc^2 - 1)))^(1/2)*(e_xc^2 + e_yc^2 - 1)*(2*cos(u_c - atan2(e_yc, e_xc) + (13*sin(3*u_c - 3*atan2(e_yc, e_xc))*(e_xc^2 + e_yc^2)^(3/2))/12 + sin(u_c - atan2(e_yc, e_xc))*(2*(e_xc^2 + e_yc^2)^(1/2) - (e_xc^2 + e_yc^2)^(3/2)/4) + sin(2*u_c - 2*atan2(e_yc, e_xc))*((5*e_xc^2)/4 + (5*e_yc^2)/4))*(e_xc^2 + e_yc^2)^(1/2) + e_xc^2 + e_yc^2 + 1)^(1/2)) - (2*B_c*e_xc*e_yc*mu*rho*(cos(u_c - atan2(e_yc, e_xc) + (13*sin(3*u_c - 3*atan2(e_yc, e_xc))*(e_xc^2 + e_yc^2)^(3/2))/12 + sin(u_c - atan2(e_yc, e_xc))*(2*(e_xc^2 + e_yc^2)^(1/2) - (e_xc^2 + e_yc^2)^(3/2)/4) + sin(2*u_c - 2*atan2(e_yc, e_xc))*((5*e_xc^2)/4 + (5*e_yc^2)/4)) + (e_xc^2 + e_yc^2)^(1/2))*(delta_B + 1)*(2*cos(u_c - atan2(e_yc, e_xc) + (13*sin(3*u_c - 3*atan2(e_yc, e_xc))*(e_xc^2 + e_yc^2)^(3/2))/12 + sin(u_c - atan2(e_yc, e_xc))*(2*(e_xc^2 + e_yc^2)^(1/2) - (e_xc^2 + e_yc^2)^(3/2)/4) + sin(2*u_c - 2*atan2(e_yc, e_xc))*((5*e_xc^2)/4 + (5*e_yc^2)/4))*(e_xc^2 + e_yc^2)^(1/2) + e_xc^2 + e_yc^2 + 1)^(1/2))/(a_c*(e_xc^2 + e_yc^2)^(1/2)*(-mu/(a_c*(e_xc^2 + e_yc^2 - 1)))^(1/2)*(e_xc^2 + e_yc^2 - 1)^2) - (B_c*e_xc*e_yc*mu*rho*(cos(u_c - atan2(e_yc, e_xc) + (13*sin(3*u_c - 3*atan2(e_yc, e_xc))*(e_xc^2 + e_yc^2)^(3/2))/12 + sin(u_c - atan2(e_yc, e_xc))*(2*(e_xc^2 + e_yc^2)^(1/2) - (e_xc^2 + e_yc^2)^(3/2)/4) + sin(2*u_c - 2*atan2(e_yc, e_xc))*((5*e_xc^2)/4 + (5*e_yc^2)/4)) + (e_xc^2 + e_yc^2)^(1/2))*(delta_B + 1)*(2*cos(u_c - atan2(e_yc, e_xc) + (13*sin(3*u_c - 3*atan2(e_yc, e_xc))*(e_xc^2 + e_yc^2)^(3/2))/12 + sin(u_c - atan2(e_yc, e_xc))*(2*(e_xc^2 + e_yc^2)^(1/2) - (e_xc^2 + e_yc^2)^(3/2)/4) + sin(2*u_c - 2*atan2(e_yc, e_xc))*((5*e_xc^2)/4 + (5*e_yc^2)/4))*(e_xc^2 + e_yc^2)^(1/2) + e_xc^2 + e_yc^2 + 1)^(1/2))/(a_c*(e_xc^2 + e_yc^2)^(3/2)*(-mu/(a_c*(e_xc^2 + e_yc^2 - 1)))^(1/2)*(e_xc^2 + e_yc^2 - 1)) + (B_c*e_yc*mu*rho*cos(u_c - atan2(e_yc, e_xc) + (13*sin(3*u_c - 3*atan2(e_yc, e_xc))*(e_xc^2 + e_yc^2)^(3/2))/12 + sin(u_c - atan2(e_yc, e_xc))*(2*(e_xc^2 + e_yc^2)^(1/2) - (e_xc^2 + e_yc^2)^(3/2)/4) + sin(2*u_c - 2*atan2(e_yc, e_xc))*((5*e_xc^2)/4 + (5*e_yc^2)/4))*(delta_B + 1)*(2*cos(u_c - atan2(e_yc, e_xc) + (13*sin(3*u_c - 3*atan2(e_yc, e_xc))*(e_xc^2 + e_yc^2)^(3/2))/12 + sin(u_c - atan2(e_yc, e_xc))*(2*(e_xc^2 + e_yc^2)^(1/2) - (e_xc^2 + e_yc^2)^(3/2)/4) + sin(2*u_c - 2*atan2(e_yc, e_xc))*((5*e_xc^2)/4 + (5*e_yc^2)/4))*(e_xc^2 + e_yc^2)^(1/2) + e_xc^2 + e_yc^2 + 1)^(1/2)*(e_xc/(e_xc^2 + e_yc^2) - sin(u_c - atan2(e_yc, e_xc))*((2*e_yc)/(e_xc^2 + e_yc^2)^(1/2) - (3*e_yc*(e_xc^2 + e_yc^2)^(1/2))/4) - (5*e_yc*sin(2*u_c - 2*atan2(e_yc, e_xc)))/2 + (13*e_xc*cos(3*u_c - 3*atan2(e_yc, e_xc))*(e_xc^2 + e_yc^2)^(1/2))/4 - (13*e_yc*sin(3*u_c - 3*atan2(e_yc, e_xc))*(e_xc^2 + e_yc^2)^(1/2))/4 + (e_xc*cos(u_c - atan2(e_yc, e_xc))*(2*(e_xc^2 + e_yc^2)^(1/2) - (e_xc^2 + e_yc^2)^(3/2)/4))/(e_xc^2 + e_yc^2) + (2*e_xc*cos(2*u_c - 2*atan2(e_yc, e_xc))*((5*e_xc^2)/4 + (5*e_yc^2)/4))/(e_xc^2 + e_yc^2)))/(a_c*(e_xc^2 + e_yc^2)^(1/2)*(-mu/(a_c*(e_xc^2 + e_yc^2 - 1)))^(1/2)*(e_xc^2 + e_yc^2 - 1)) + (B_c*e_xc*mu*rho*(cos(u_c - atan2(e_yc, e_xc) + (13*sin(3*u_c - 3*atan2(e_yc, e_xc))*(e_xc^2 + e_yc^2)^(3/2))/12 + sin(u_c - atan2(e_yc, e_xc))*(2*(e_xc^2 + e_yc^2)^(1/2) - (e_xc^2 + e_yc^2)^(3/2)/4) + sin(2*u_c - 2*atan2(e_yc, e_xc))*((5*e_xc^2)/4 + (5*e_yc^2)/4)) + (e_xc^2 + e_yc^2)^(1/2))*(delta_B + 1)*(2*e_yc + (2*e_yc*cos(u_c - atan2(e_yc, e_xc) + (13*sin(3*u_c - 3*atan2(e_yc, e_xc))*(e_xc^2 + e_yc^2)^(3/2))/12 + sin(u_c - atan2(e_yc, e_xc))*(2*(e_xc^2 + e_yc^2)^(1/2) - (e_xc^2 + e_yc^2)^(3/2)/4) + sin(2*u_c - 2*atan2(e_yc, e_xc))*((5*e_xc^2)/4 + (5*e_yc^2)/4)))/(e_xc^2 + e_yc^2)^(1/2) + 2*sin(u_c - atan2(e_yc, e_xc) + (13*sin(3*u_c - 3*atan2(e_yc, e_xc))*(e_xc^2 + e_yc^2)^(3/2))/12 + sin(u_c - atan2(e_yc, e_xc))*(2*(e_xc^2 + e_yc^2)^(1/2) - (e_xc^2 + e_yc^2)^(3/2)/4) + sin(2*u_c - 2*atan2(e_yc, e_xc))*((5*e_xc^2)/4 + (5*e_yc^2)/4))*(e_xc^2 + e_yc^2)^(1/2)*(e_xc/(e_xc^2 + e_yc^2) - sin(u_c - atan2(e_yc, e_xc))*((2*e_yc)/(e_xc^2 + e_yc^2)^(1/2) - (3*e_yc*(e_xc^2 + e_yc^2)^(1/2))/4) - (5*e_yc*sin(2*u_c - 2*atan2(e_yc, e_xc)))/2 + (13*e_xc*cos(3*u_c - 3*atan2(e_yc, e_xc))*(e_xc^2 + e_yc^2)^(1/2))/4 - (13*e_yc*sin(3*u_c - 3*atan2(e_yc, e_xc))*(e_xc^2 + e_yc^2)^(1/2))/4 + (e_xc*cos(u_c - atan2(e_yc, e_xc))*(2*(e_xc^2 + e_yc^2)^(1/2) - (e_xc^2 + e_yc^2)^(3/2)/4))/(e_xc^2 + e_yc^2) + (2*e_xc*cos(2*u_c - 2*atan2(e_yc, e_xc))*((5*e_xc^2)/4 + (5*e_yc^2)/4))/(e_xc^2 + e_yc^2))))/(2*a_c*(e_xc^2 + e_yc^2)^(1/2)*(-mu/(a_c*(e_xc^2 + e_yc^2 - 1)))^(1/2)*(e_xc^2 + e_yc^2 - 1)*(2*cos(u_c - atan2(e_yc, e_xc) + (13*sin(3*u_c - 3*atan2(e_yc, e_xc))*(e_xc^2 + e_yc^2)^(3/2))/12 + sin(u_c - atan2(e_yc, e_xc))*(2*(e_xc^2 + e_yc^2)^(1/2) - (e_xc^2 + e_yc^2)^(3/2)/4) + sin(2*u_c - 2*atan2(e_yc, e_xc))*((5*e_xc^2)/4 + (5*e_yc^2)/4))*(e_xc^2 + e_yc^2)^(1/2) + e_xc^2 + e_yc^2 + 1)^(1/2)) - (B_c*e_xc*e_yc*mu^2*rho*(cos(u_c - atan2(e_yc, e_xc) + (13*sin(3*u_c - 3*atan2(e_yc, e_xc))*(e_xc^2 + e_yc^2)^(3/2))/12 + sin(u_c - atan2(e_yc, e_xc))*(2*(e_xc^2 + e_yc^2)^(1/2) - (e_xc^2 + e_yc^2)^(3/2)/4) + sin(2*u_c - 2*atan2(e_yc, e_xc))*((5*e_xc^2)/4 + (5*e_yc^2)/4)) + (e_xc^2 + e_yc^2)^(1/2))*(delta_B + 1)*(2*cos(u_c - atan2(e_yc, e_xc) + (13*sin(3*u_c - 3*atan2(e_yc, e_xc))*(e_xc^2 + e_yc^2)^(3/2))/12 + sin(u_c - atan2(e_yc, e_xc))*(2*(e_xc^2 + e_yc^2)^(1/2) - (e_xc^2 + e_yc^2)^(3/2)/4) + sin(2*u_c - 2*atan2(e_yc, e_xc))*((5*e_xc^2)/4 + (5*e_yc^2)/4))*(e_xc^2 + e_yc^2)^(1/2) + e_xc^2 + e_yc^2 + 1)^(1/2))/(a_c^2*(e_xc^2 + e_yc^2)^(1/2)*(-mu/(a_c*(e_xc^2 + e_yc^2 - 1)))^(3/2)*(e_xc^2 + e_yc^2 - 1)^3);
% A_drag(3,5) = 0;
% A_drag(3,6) = (B_c*e_xc*mu*rho*sin(u_c - atan2(e_yc, e_xc) + (13*sin(3*u_c - 3*atan2(e_yc, e_xc))*(e_xc^2 + e_yc^2)^(3/2))/12 + sin(u_c - atan2(e_yc, e_xc))*(2*(e_xc^2 + e_yc^2)^(1/2) - (e_xc^2 + e_yc^2)^(3/2)/4) + sin(2*u_c - 2*atan2(e_yc, e_xc))*((5*e_xc^2)/4 + (5*e_yc^2)/4))*(cos(u_c - atan2(e_yc, e_xc) + (13*sin(3*u_c - 3*atan2(e_yc, e_xc))*(e_xc^2 + e_yc^2)^(3/2))/12 + sin(u_c - atan2(e_yc, e_xc))*(2*(e_xc^2 + e_yc^2)^(1/2) - (e_xc^2 + e_yc^2)^(3/2)/4) + sin(2*u_c - 2*atan2(e_yc, e_xc))*((5*e_xc^2)/4 + (5*e_yc^2)/4)) + (e_xc^2 + e_yc^2)^(1/2))*(delta_B + 1)*(1/tan(i_c) + (2*cos(2*u_c - 2*atan2(e_yc, e_xc))*((5*e_xc^2)/4 + (5*e_yc^2)/4))/tan(i_c) + (13*cos(3*u_c - 3*atan2(e_yc, e_xc))*(e_xc^2 + e_yc^2)^(3/2))/(4*tan(i_c)) + (cos(u_c - atan2(e_yc, e_xc))*(2*(e_xc^2 + e_yc^2)^(1/2) - (e_xc^2 + e_yc^2)^(3/2)/4))/tan(i_c)))/(a_c*(-mu/(a_c*(e_xc^2 + e_yc^2 - 1)))^(1/2)*(e_xc^2 + e_yc^2 - 1)*(2*cos(u_c - atan2(e_yc, e_xc) + (13*sin(3*u_c - 3*atan2(e_yc, e_xc))*(e_xc^2 + e_yc^2)^(3/2))/12 + sin(u_c - atan2(e_yc, e_xc))*(2*(e_xc^2 + e_yc^2)^(1/2) - (e_xc^2 + e_yc^2)^(3/2)/4) + sin(2*u_c - 2*atan2(e_yc, e_xc))*((5*e_xc^2)/4 + (5*e_yc^2)/4))*(e_xc^2 + e_yc^2)^(1/2) + e_xc^2 + e_yc^2 + 1)^(1/2)) - (B_c*e_yc*mu*rho*sin(u_c - atan2(e_yc, e_xc) + (13*sin(3*u_c - 3*atan2(e_yc, e_xc))*(e_xc^2 + e_yc^2)^(3/2))/12 + sin(u_c - atan2(e_yc, e_xc))*(2*(e_xc^2 + e_yc^2)^(1/2) - (e_xc^2 + e_yc^2)^(3/2)/4) + sin(2*u_c - 2*atan2(e_yc, e_xc))*((5*e_xc^2)/4 + (5*e_yc^2)/4))^2*(delta_B + 1)*(1/tan(i_c) + (2*cos(2*u_c - 2*atan2(e_yc, e_xc))*((5*e_xc^2)/4 + (5*e_yc^2)/4))/tan(i_c) + (13*cos(3*u_c - 3*atan2(e_yc, e_xc))*(e_xc^2 + e_yc^2)^(3/2))/(4*tan(i_c)) + (cos(u_c - atan2(e_yc, e_xc))*(2*(e_xc^2 + e_yc^2)^(1/2) - (e_xc^2 + e_yc^2)^(3/2)/4))/tan(i_c)))/(a_c*(-mu/(a_c*(e_xc^2 + e_yc^2 - 1)))^(1/2)*(e_xc^2 + e_yc^2 - 1)*(2*cos(u_c - atan2(e_yc, e_xc) + (13*sin(3*u_c - 3*atan2(e_yc, e_xc))*(e_xc^2 + e_yc^2)^(3/2))/12 + sin(u_c - atan2(e_yc, e_xc))*(2*(e_xc^2 + e_yc^2)^(1/2) - (e_xc^2 + e_yc^2)^(3/2)/4) + sin(2*u_c - 2*atan2(e_yc, e_xc))*((5*e_xc^2)/4 + (5*e_yc^2)/4))*(e_xc^2 + e_yc^2)^(1/2) + e_xc^2 + e_yc^2 + 1)^(1/2)) + (B_c*e_yc*mu*rho*cos(u_c - atan2(e_yc, e_xc) + (13*sin(3*u_c - 3*atan2(e_yc, e_xc))*(e_xc^2 + e_yc^2)^(3/2))/12 + sin(u_c - atan2(e_yc, e_xc))*(2*(e_xc^2 + e_yc^2)^(1/2) - (e_xc^2 + e_yc^2)^(3/2)/4) + sin(2*u_c - 2*atan2(e_yc, e_xc))*((5*e_xc^2)/4 + (5*e_yc^2)/4))*(delta_B + 1)*(2*cos(u_c - atan2(e_yc, e_xc) + (13*sin(3*u_c - 3*atan2(e_yc, e_xc))*(e_xc^2 + e_yc^2)^(3/2))/12 + sin(u_c - atan2(e_yc, e_xc))*(2*(e_xc^2 + e_yc^2)^(1/2) - (e_xc^2 + e_yc^2)^(3/2)/4) + sin(2*u_c - 2*atan2(e_yc, e_xc))*((5*e_xc^2)/4 + (5*e_yc^2)/4))*(e_xc^2 + e_yc^2)^(1/2) + e_xc^2 + e_yc^2 + 1)^(1/2)*(1/tan(i_c) + (2*cos(2*u_c - 2*atan2(e_yc, e_xc))*((5*e_xc^2)/4 + (5*e_yc^2)/4))/tan(i_c) + (13*cos(3*u_c - 3*atan2(e_yc, e_xc))*(e_xc^2 + e_yc^2)^(3/2))/(4*tan(i_c)) + (cos(u_c - atan2(e_yc, e_xc))*(2*(e_xc^2 + e_yc^2)^(1/2) - (e_xc^2 + e_yc^2)^(3/2)/4))/tan(i_c)))/(a_c*(e_xc^2 + e_yc^2)^(1/2)*(-mu/(a_c*(e_xc^2 + e_yc^2 - 1)))^(1/2)*(e_xc^2 + e_yc^2 - 1)) + (B_c*e_xc*mu*rho*sin(u_c - atan2(e_yc, e_xc) + (13*sin(3*u_c - 3*atan2(e_yc, e_xc))*(e_xc^2 + e_yc^2)^(3/2))/12 + sin(u_c - atan2(e_yc, e_xc))*(2*(e_xc^2 + e_yc^2)^(1/2) - (e_xc^2 + e_yc^2)^(3/2)/4) + sin(2*u_c - 2*atan2(e_yc, e_xc))*((5*e_xc^2)/4 + (5*e_yc^2)/4))*(delta_B + 1)*(2*cos(u_c - atan2(e_yc, e_xc) + (13*sin(3*u_c - 3*atan2(e_yc, e_xc))*(e_xc^2 + e_yc^2)^(3/2))/12 + sin(u_c - atan2(e_yc, e_xc))*(2*(e_xc^2 + e_yc^2)^(1/2) - (e_xc^2 + e_yc^2)^(3/2)/4) + sin(2*u_c - 2*atan2(e_yc, e_xc))*((5*e_xc^2)/4 + (5*e_yc^2)/4))*(e_xc^2 + e_yc^2)^(1/2) + e_xc^2 + e_yc^2 + 1)^(1/2)*(1/tan(i_c) + (2*cos(2*u_c - 2*atan2(e_yc, e_xc))*((5*e_xc^2)/4 + (5*e_yc^2)/4))/tan(i_c) + (13*cos(3*u_c - 3*atan2(e_yc, e_xc))*(e_xc^2 + e_yc^2)^(3/2))/(4*tan(i_c)) + (cos(u_c - atan2(e_yc, e_xc))*(2*(e_xc^2 + e_yc^2)^(1/2) - (e_xc^2 + e_yc^2)^(3/2)/4))/tan(i_c)))/(a_c*(e_xc^2 + e_yc^2)^(1/2)*(-mu/(a_c*(e_xc^2 + e_yc^2 - 1)))^(1/2)*(e_xc^2 + e_yc^2 - 1));
% A_drag(3,7) = (B_c*e_xc*mu*rho*(cos(u_c - atan2(e_yc, e_xc) + (13*sin(3*u_c - 3*atan2(e_yc, e_xc))*(e_xc^2 + e_yc^2)^(3/2))/12 + sin(u_c - atan2(e_yc, e_xc))*(2*(e_xc^2 + e_yc^2)^(1/2) - (e_xc^2 + e_yc^2)^(3/2)/4) + sin(2*u_c - 2*atan2(e_yc, e_xc))*((5*e_xc^2)/4 + (5*e_yc^2)/4)) + (e_xc^2 + e_yc^2)^(1/2))*(2*cos(u_c - atan2(e_yc, e_xc) + (13*sin(3*u_c - 3*atan2(e_yc, e_xc))*(e_xc^2 + e_yc^2)^(3/2))/12 + sin(u_c - atan2(e_yc, e_xc))*(2*(e_xc^2 + e_yc^2)^(1/2) - (e_xc^2 + e_yc^2)^(3/2)/4) + sin(2*u_c - 2*atan2(e_yc, e_xc))*((5*e_xc^2)/4 + (5*e_yc^2)/4))*(e_xc^2 + e_yc^2)^(1/2) + e_xc^2 + e_yc^2 + 1)^(1/2))/(a_c*(e_xc^2 + e_yc^2)^(1/2)*(-mu/(a_c*(e_xc^2 + e_yc^2 - 1)))^(1/2)*(e_xc^2 + e_yc^2 - 1)) - (B_c*e_yc*mu*rho*sin(u_c - atan2(e_yc, e_xc) + (13*sin(3*u_c - 3*atan2(e_yc, e_xc))*(e_xc^2 + e_yc^2)^(3/2))/12 + sin(u_c - atan2(e_yc, e_xc))*(2*(e_xc^2 + e_yc^2)^(1/2) - (e_xc^2 + e_yc^2)^(3/2)/4) + sin(2*u_c - 2*atan2(e_yc, e_xc))*((5*e_xc^2)/4 + (5*e_yc^2)/4))*(2*cos(u_c - atan2(e_yc, e_xc) + (13*sin(3*u_c - 3*atan2(e_yc, e_xc))*(e_xc^2 + e_yc^2)^(3/2))/12 + sin(u_c - atan2(e_yc, e_xc))*(2*(e_xc^2 + e_yc^2)^(1/2) - (e_xc^2 + e_yc^2)^(3/2)/4) + sin(2*u_c - 2*atan2(e_yc, e_xc))*((5*e_xc^2)/4 + (5*e_yc^2)/4))*(e_xc^2 + e_yc^2)^(1/2) + e_xc^2 + e_yc^2 + 1)^(1/2))/(a_c*(e_xc^2 + e_yc^2)^(1/2)*(-mu/(a_c*(e_xc^2 + e_yc^2 - 1)))^(1/2)*(e_xc^2 + e_yc^2 - 1));
% A_drag(4,1) = - (B_c*e_xc*mu^2*rho*sin(u_c - atan2(e_yc, e_xc) + (13*sin(3*u_c - 3*atan2(e_yc, e_xc))*(e_xc^2 + e_yc^2)^(3/2))/12 + sin(u_c - atan2(e_yc, e_xc))*(2*(e_xc^2 + e_yc^2)^(1/2) - (e_xc^2 + e_yc^2)^(3/2)/4) + sin(2*u_c - 2*atan2(e_yc, e_xc))*((5*e_xc^2)/4 + (5*e_yc^2)/4))*(delta_B + 1)*(2*cos(u_c - atan2(e_yc, e_xc) + (13*sin(3*u_c - 3*atan2(e_yc, e_xc))*(e_xc^2 + e_yc^2)^(3/2))/12 + sin(u_c - atan2(e_yc, e_xc))*(2*(e_xc^2 + e_yc^2)^(1/2) - (e_xc^2 + e_yc^2)^(3/2)/4) + sin(2*u_c - 2*atan2(e_yc, e_xc))*((5*e_xc^2)/4 + (5*e_yc^2)/4))*(e_xc^2 + e_yc^2)^(1/2) + e_xc^2 + e_yc^2 + 1)^(1/2))/(2*a_c^2*(e_xc^2 + e_yc^2)^(1/2)*(-mu/(a_c*(e_xc^2 + e_yc^2 - 1)))^(3/2)*(e_xc^2 + e_yc^2 - 1)^2) - (B_c*e_yc*mu*rho*(cos(u_c - atan2(e_yc, e_xc) + (13*sin(3*u_c - 3*atan2(e_yc, e_xc))*(e_xc^2 + e_yc^2)^(3/2))/12 + sin(u_c - atan2(e_yc, e_xc))*(2*(e_xc^2 + e_yc^2)^(1/2) - (e_xc^2 + e_yc^2)^(3/2)/4) + sin(2*u_c - 2*atan2(e_yc, e_xc))*((5*e_xc^2)/4 + (5*e_yc^2)/4)) + (e_xc^2 + e_yc^2)^(1/2))*(delta_B + 1)*(2*cos(u_c - atan2(e_yc, e_xc) + (13*sin(3*u_c - 3*atan2(e_yc, e_xc))*(e_xc^2 + e_yc^2)^(3/2))/12 + sin(u_c - atan2(e_yc, e_xc))*(2*(e_xc^2 + e_yc^2)^(1/2) - (e_xc^2 + e_yc^2)^(3/2)/4) + sin(2*u_c - 2*atan2(e_yc, e_xc))*((5*e_xc^2)/4 + (5*e_yc^2)/4))*(e_xc^2 + e_yc^2)^(1/2) + e_xc^2 + e_yc^2 + 1)^(1/2))/(a_c*(e_xc^2 + e_yc^2)^(1/2)*(-mu/(a_c*(e_xc^2 + e_yc^2 - 1)))^(1/2)*(e_xc^2 + e_yc^2 - 1)) - (B_c*e_yc*mu^2*rho*(cos(u_c - atan2(e_yc, e_xc) + (13*sin(3*u_c - 3*atan2(e_yc, e_xc))*(e_xc^2 + e_yc^2)^(3/2))/12 + sin(u_c - atan2(e_yc, e_xc))*(2*(e_xc^2 + e_yc^2)^(1/2) - (e_xc^2 + e_yc^2)^(3/2)/4) + sin(2*u_c - 2*atan2(e_yc, e_xc))*((5*e_xc^2)/4 + (5*e_yc^2)/4)) + (e_xc^2 + e_yc^2)^(1/2))*(delta_B + 1)*(2*cos(u_c - atan2(e_yc, e_xc) + (13*sin(3*u_c - 3*atan2(e_yc, e_xc))*(e_xc^2 + e_yc^2)^(3/2))/12 + sin(u_c - atan2(e_yc, e_xc))*(2*(e_xc^2 + e_yc^2)^(1/2) - (e_xc^2 + e_yc^2)^(3/2)/4) + sin(2*u_c - 2*atan2(e_yc, e_xc))*((5*e_xc^2)/4 + (5*e_yc^2)/4))*(e_xc^2 + e_yc^2)^(1/2) + e_xc^2 + e_yc^2 + 1)^(1/2))/(2*a_c^2*(e_xc^2 + e_yc^2)^(1/2)*(-mu/(a_c*(e_xc^2 + e_yc^2 - 1)))^(3/2)*(e_xc^2 + e_yc^2 - 1)^2) - (B_c*e_xc*mu*rho*sin(u_c - atan2(e_yc, e_xc) + (13*sin(3*u_c - 3*atan2(e_yc, e_xc))*(e_xc^2 + e_yc^2)^(3/2))/12 + sin(u_c - atan2(e_yc, e_xc))*(2*(e_xc^2 + e_yc^2)^(1/2) - (e_xc^2 + e_yc^2)^(3/2)/4) + sin(2*u_c - 2*atan2(e_yc, e_xc))*((5*e_xc^2)/4 + (5*e_yc^2)/4))*(delta_B + 1)*(2*cos(u_c - atan2(e_yc, e_xc) + (13*sin(3*u_c - 3*atan2(e_yc, e_xc))*(e_xc^2 + e_yc^2)^(3/2))/12 + sin(u_c - atan2(e_yc, e_xc))*(2*(e_xc^2 + e_yc^2)^(1/2) - (e_xc^2 + e_yc^2)^(3/2)/4) + sin(2*u_c - 2*atan2(e_yc, e_xc))*((5*e_xc^2)/4 + (5*e_yc^2)/4))*(e_xc^2 + e_yc^2)^(1/2) + e_xc^2 + e_yc^2 + 1)^(1/2))/(a_c*(e_xc^2 + e_yc^2)^(1/2)*(-mu/(a_c*(e_xc^2 + e_yc^2 - 1)))^(1/2)*(e_xc^2 + e_yc^2 - 1));
% A_drag(4,2) = (B_c*e_xc*mu*rho*cos(u_c - atan2(e_yc, e_xc) + (13*sin(3*u_c - 3*atan2(e_yc, e_xc))*(e_xc^2 + e_yc^2)^(3/2))/12 + sin(u_c - atan2(e_yc, e_xc))*(2*(e_xc^2 + e_yc^2)^(1/2) - (e_xc^2 + e_yc^2)^(3/2)/4) + sin(2*u_c - 2*atan2(e_yc, e_xc))*((5*e_xc^2)/4 + (5*e_yc^2)/4))*(delta_B + 1)*(2*cos(u_c - atan2(e_yc, e_xc) + (13*sin(3*u_c - 3*atan2(e_yc, e_xc))*(e_xc^2 + e_yc^2)^(3/2))/12 + sin(u_c - atan2(e_yc, e_xc))*(2*(e_xc^2 + e_yc^2)^(1/2) - (e_xc^2 + e_yc^2)^(3/2)/4) + sin(2*u_c - 2*atan2(e_yc, e_xc))*((5*e_xc^2)/4 + (5*e_yc^2)/4))*(e_xc^2 + e_yc^2)^(1/2) + e_xc^2 + e_yc^2 + 1)^(1/2)*((13*cos(3*u_c - 3*atan2(e_yc, e_xc))*(e_xc^2 + e_yc^2)^(3/2))/4 + cos(u_c - atan2(e_yc, e_xc))*(2*(e_xc^2 + e_yc^2)^(1/2) - (e_xc^2 + e_yc^2)^(3/2)/4) + 2*cos(2*u_c - 2*atan2(e_yc, e_xc))*((5*e_xc^2)/4 + (5*e_yc^2)/4) + 1))/(a_c*(e_xc^2 + e_yc^2)^(1/2)*(-mu/(a_c*(e_xc^2 + e_yc^2 - 1)))^(1/2)*(e_xc^2 + e_yc^2 - 1)) - (B_c*e_yc*mu*rho*sin(u_c - atan2(e_yc, e_xc) + (13*sin(3*u_c - 3*atan2(e_yc, e_xc))*(e_xc^2 + e_yc^2)^(3/2))/12 + sin(u_c - atan2(e_yc, e_xc))*(2*(e_xc^2 + e_yc^2)^(1/2) - (e_xc^2 + e_yc^2)^(3/2)/4) + sin(2*u_c - 2*atan2(e_yc, e_xc))*((5*e_xc^2)/4 + (5*e_yc^2)/4))*(delta_B + 1)*(2*cos(u_c - atan2(e_yc, e_xc) + (13*sin(3*u_c - 3*atan2(e_yc, e_xc))*(e_xc^2 + e_yc^2)^(3/2))/12 + sin(u_c - atan2(e_yc, e_xc))*(2*(e_xc^2 + e_yc^2)^(1/2) - (e_xc^2 + e_yc^2)^(3/2)/4) + sin(2*u_c - 2*atan2(e_yc, e_xc))*((5*e_xc^2)/4 + (5*e_yc^2)/4))*(e_xc^2 + e_yc^2)^(1/2) + e_xc^2 + e_yc^2 + 1)^(1/2)*((13*cos(3*u_c - 3*atan2(e_yc, e_xc))*(e_xc^2 + e_yc^2)^(3/2))/4 + cos(u_c - atan2(e_yc, e_xc))*(2*(e_xc^2 + e_yc^2)^(1/2) - (e_xc^2 + e_yc^2)^(3/2)/4) + 2*cos(2*u_c - 2*atan2(e_yc, e_xc))*((5*e_xc^2)/4 + (5*e_yc^2)/4) + 1))/(a_c*(e_xc^2 + e_yc^2)^(1/2)*(-mu/(a_c*(e_xc^2 + e_yc^2 - 1)))^(1/2)*(e_xc^2 + e_yc^2 - 1)) - (B_c*e_yc*mu*rho*sin(u_c - atan2(e_yc, e_xc) + (13*sin(3*u_c - 3*atan2(e_yc, e_xc))*(e_xc^2 + e_yc^2)^(3/2))/12 + sin(u_c - atan2(e_yc, e_xc))*(2*(e_xc^2 + e_yc^2)^(1/2) - (e_xc^2 + e_yc^2)^(3/2)/4) + sin(2*u_c - 2*atan2(e_yc, e_xc))*((5*e_xc^2)/4 + (5*e_yc^2)/4))*(cos(u_c - atan2(e_yc, e_xc) + (13*sin(3*u_c - 3*atan2(e_yc, e_xc))*(e_xc^2 + e_yc^2)^(3/2))/12 + sin(u_c - atan2(e_yc, e_xc))*(2*(e_xc^2 + e_yc^2)^(1/2) - (e_xc^2 + e_yc^2)^(3/2)/4) + sin(2*u_c - 2*atan2(e_yc, e_xc))*((5*e_xc^2)/4 + (5*e_yc^2)/4)) + (e_xc^2 + e_yc^2)^(1/2))*(delta_B + 1)*((13*cos(3*u_c - 3*atan2(e_yc, e_xc))*(e_xc^2 + e_yc^2)^(3/2))/4 + cos(u_c - atan2(e_yc, e_xc))*(2*(e_xc^2 + e_yc^2)^(1/2) - (e_xc^2 + e_yc^2)^(3/2)/4) + 2*cos(2*u_c - 2*atan2(e_yc, e_xc))*((5*e_xc^2)/4 + (5*e_yc^2)/4) + 1))/(a_c*(-mu/(a_c*(e_xc^2 + e_yc^2 - 1)))^(1/2)*(e_xc^2 + e_yc^2 - 1)*(2*cos(u_c - atan2(e_yc, e_xc) + (13*sin(3*u_c - 3*atan2(e_yc, e_xc))*(e_xc^2 + e_yc^2)^(3/2))/12 + sin(u_c - atan2(e_yc, e_xc))*(2*(e_xc^2 + e_yc^2)^(1/2) - (e_xc^2 + e_yc^2)^(3/2)/4) + sin(2*u_c - 2*atan2(e_yc, e_xc))*((5*e_xc^2)/4 + (5*e_yc^2)/4))*(e_xc^2 + e_yc^2)^(1/2) + e_xc^2 + e_yc^2 + 1)^(1/2)) - (B_c*e_xc*mu*rho*sin(u_c - atan2(e_yc, e_xc) + (13*sin(3*u_c - 3*atan2(e_yc, e_xc))*(e_xc^2 + e_yc^2)^(3/2))/12 + sin(u_c - atan2(e_yc, e_xc))*(2*(e_xc^2 + e_yc^2)^(1/2) - (e_xc^2 + e_yc^2)^(3/2)/4) + sin(2*u_c - 2*atan2(e_yc, e_xc))*((5*e_xc^2)/4 + (5*e_yc^2)/4))^2*(delta_B + 1)*((13*cos(3*u_c - 3*atan2(e_yc, e_xc))*(e_xc^2 + e_yc^2)^(3/2))/4 + cos(u_c - atan2(e_yc, e_xc))*(2*(e_xc^2 + e_yc^2)^(1/2) - (e_xc^2 + e_yc^2)^(3/2)/4) + 2*cos(2*u_c - 2*atan2(e_yc, e_xc))*((5*e_xc^2)/4 + (5*e_yc^2)/4) + 1))/(a_c*(-mu/(a_c*(e_xc^2 + e_yc^2 - 1)))^(1/2)*(e_xc^2 + e_yc^2 - 1)*(2*cos(u_c - atan2(e_yc, e_xc) + (13*sin(3*u_c - 3*atan2(e_yc, e_xc))*(e_xc^2 + e_yc^2)^(3/2))/12 + sin(u_c - atan2(e_yc, e_xc))*(2*(e_xc^2 + e_yc^2)^(1/2) - (e_xc^2 + e_yc^2)^(3/2)/4) + sin(2*u_c - 2*atan2(e_yc, e_xc))*((5*e_xc^2)/4 + (5*e_yc^2)/4))*(e_xc^2 + e_yc^2)^(1/2) + e_xc^2 + e_yc^2 + 1)^(1/2));
% A_drag(4,3) = (B_c*mu*rho*sin(u_c - atan2(e_yc, e_xc) + (13*sin(3*u_c - 3*atan2(e_yc, e_xc))*(e_xc^2 + e_yc^2)^(3/2))/12 + sin(u_c - atan2(e_yc, e_xc))*(2*(e_xc^2 + e_yc^2)^(1/2) - (e_xc^2 + e_yc^2)^(3/2)/4) + sin(2*u_c - 2*atan2(e_yc, e_xc))*((5*e_xc^2)/4 + (5*e_yc^2)/4))*(delta_B + 1)*(2*cos(u_c - atan2(e_yc, e_xc) + (13*sin(3*u_c - 3*atan2(e_yc, e_xc))*(e_xc^2 + e_yc^2)^(3/2))/12 + sin(u_c - atan2(e_yc, e_xc))*(2*(e_xc^2 + e_yc^2)^(1/2) - (e_xc^2 + e_yc^2)^(3/2)/4) + sin(2*u_c - 2*atan2(e_yc, e_xc))*((5*e_xc^2)/4 + (5*e_yc^2)/4))*(e_xc^2 + e_yc^2)^(1/2) + e_xc^2 + e_yc^2 + 1)^(1/2))/(a_c*(e_xc^2 + e_yc^2)^(1/2)*(-mu/(a_c*(e_xc^2 + e_yc^2 - 1)))^(1/2)*(e_xc^2 + e_yc^2 - 1)) - (2*B_c*e_xc^2*mu*rho*sin(u_c - atan2(e_yc, e_xc) + (13*sin(3*u_c - 3*atan2(e_yc, e_xc))*(e_xc^2 + e_yc^2)^(3/2))/12 + sin(u_c - atan2(e_yc, e_xc))*(2*(e_xc^2 + e_yc^2)^(1/2) - (e_xc^2 + e_yc^2)^(3/2)/4) + sin(2*u_c - 2*atan2(e_yc, e_xc))*((5*e_xc^2)/4 + (5*e_yc^2)/4))*(delta_B + 1)*(2*cos(u_c - atan2(e_yc, e_xc) + (13*sin(3*u_c - 3*atan2(e_yc, e_xc))*(e_xc^2 + e_yc^2)^(3/2))/12 + sin(u_c - atan2(e_yc, e_xc))*(2*(e_xc^2 + e_yc^2)^(1/2) - (e_xc^2 + e_yc^2)^(3/2)/4) + sin(2*u_c - 2*atan2(e_yc, e_xc))*((5*e_xc^2)/4 + (5*e_yc^2)/4))*(e_xc^2 + e_yc^2)^(1/2) + e_xc^2 + e_yc^2 + 1)^(1/2))/(a_c*(e_xc^2 + e_yc^2)^(1/2)*(-mu/(a_c*(e_xc^2 + e_yc^2 - 1)))^(1/2)*(e_xc^2 + e_yc^2 - 1)^2) - (B_c*e_xc^2*mu*rho*sin(u_c - atan2(e_yc, e_xc) + (13*sin(3*u_c - 3*atan2(e_yc, e_xc))*(e_xc^2 + e_yc^2)^(3/2))/12 + sin(u_c - atan2(e_yc, e_xc))*(2*(e_xc^2 + e_yc^2)^(1/2) - (e_xc^2 + e_yc^2)^(3/2)/4) + sin(2*u_c - 2*atan2(e_yc, e_xc))*((5*e_xc^2)/4 + (5*e_yc^2)/4))*(delta_B + 1)*(2*cos(u_c - atan2(e_yc, e_xc) + (13*sin(3*u_c - 3*atan2(e_yc, e_xc))*(e_xc^2 + e_yc^2)^(3/2))/12 + sin(u_c - atan2(e_yc, e_xc))*(2*(e_xc^2 + e_yc^2)^(1/2) - (e_xc^2 + e_yc^2)^(3/2)/4) + sin(2*u_c - 2*atan2(e_yc, e_xc))*((5*e_xc^2)/4 + (5*e_yc^2)/4))*(e_xc^2 + e_yc^2)^(1/2) + e_xc^2 + e_yc^2 + 1)^(1/2))/(a_c*(e_xc^2 + e_yc^2)^(3/2)*(-mu/(a_c*(e_xc^2 + e_yc^2 - 1)))^(1/2)*(e_xc^2 + e_yc^2 - 1)) - (B_c*e_xc^2*mu^2*rho*sin(u_c - atan2(e_yc, e_xc) + (13*sin(3*u_c - 3*atan2(e_yc, e_xc))*(e_xc^2 + e_yc^2)^(3/2))/12 + sin(u_c - atan2(e_yc, e_xc))*(2*(e_xc^2 + e_yc^2)^(1/2) - (e_xc^2 + e_yc^2)^(3/2)/4) + sin(2*u_c - 2*atan2(e_yc, e_xc))*((5*e_xc^2)/4 + (5*e_yc^2)/4))*(delta_B + 1)*(2*cos(u_c - atan2(e_yc, e_xc) + (13*sin(3*u_c - 3*atan2(e_yc, e_xc))*(e_xc^2 + e_yc^2)^(3/2))/12 + sin(u_c - atan2(e_yc, e_xc))*(2*(e_xc^2 + e_yc^2)^(1/2) - (e_xc^2 + e_yc^2)^(3/2)/4) + sin(2*u_c - 2*atan2(e_yc, e_xc))*((5*e_xc^2)/4 + (5*e_yc^2)/4))*(e_xc^2 + e_yc^2)^(1/2) + e_xc^2 + e_yc^2 + 1)^(1/2))/(a_c^2*(e_xc^2 + e_yc^2)^(1/2)*(-mu/(a_c*(e_xc^2 + e_yc^2 - 1)))^(3/2)*(e_xc^2 + e_yc^2 - 1)^3) + (B_c*e_yc*mu*rho*(delta_B + 1)*(e_xc/(e_xc^2 + e_yc^2)^(1/2) - sin(u_c - atan2(e_yc, e_xc) + (13*sin(3*u_c - 3*atan2(e_yc, e_xc))*(e_xc^2 + e_yc^2)^(3/2))/12 + sin(u_c - atan2(e_yc, e_xc))*(2*(e_xc^2 + e_yc^2)^(1/2) - (e_xc^2 + e_yc^2)^(3/2)/4) + sin(2*u_c - 2*atan2(e_yc, e_xc))*((5*e_xc^2)/4 + (5*e_yc^2)/4))*(e_yc/(e_xc^2 + e_yc^2) + sin(u_c - atan2(e_yc, e_xc))*((2*e_xc)/(e_xc^2 + e_yc^2)^(1/2) - (3*e_xc*(e_xc^2 + e_yc^2)^(1/2))/4) + (5*e_xc*sin(2*u_c - 2*atan2(e_yc, e_xc)))/2 + (13*e_yc*cos(3*u_c - 3*atan2(e_yc, e_xc))*(e_xc^2 + e_yc^2)^(1/2))/4 + (13*e_xc*sin(3*u_c - 3*atan2(e_yc, e_xc))*(e_xc^2 + e_yc^2)^(1/2))/4 + (e_yc*cos(u_c - atan2(e_yc, e_xc))*(2*(e_xc^2 + e_yc^2)^(1/2) - (e_xc^2 + e_yc^2)^(3/2)/4))/(e_xc^2 + e_yc^2) + (2*e_yc*cos(2*u_c - 2*atan2(e_yc, e_xc))*((5*e_xc^2)/4 + (5*e_yc^2)/4))/(e_xc^2 + e_yc^2)))*(2*cos(u_c - atan2(e_yc, e_xc) + (13*sin(3*u_c - 3*atan2(e_yc, e_xc))*(e_xc^2 + e_yc^2)^(3/2))/12 + sin(u_c - atan2(e_yc, e_xc))*(2*(e_xc^2 + e_yc^2)^(1/2) - (e_xc^2 + e_yc^2)^(3/2)/4) + sin(2*u_c - 2*atan2(e_yc, e_xc))*((5*e_xc^2)/4 + (5*e_yc^2)/4))*(e_xc^2 + e_yc^2)^(1/2) + e_xc^2 + e_yc^2 + 1)^(1/2))/(a_c*(e_xc^2 + e_yc^2)^(1/2)*(-mu/(a_c*(e_xc^2 + e_yc^2 - 1)))^(1/2)*(e_xc^2 + e_yc^2 - 1)) + (B_c*e_xc*mu*rho*sin(u_c - atan2(e_yc, e_xc) + (13*sin(3*u_c - 3*atan2(e_yc, e_xc))*(e_xc^2 + e_yc^2)^(3/2))/12 + sin(u_c - atan2(e_yc, e_xc))*(2*(e_xc^2 + e_yc^2)^(1/2) - (e_xc^2 + e_yc^2)^(3/2)/4) + sin(2*u_c - 2*atan2(e_yc, e_xc))*((5*e_xc^2)/4 + (5*e_yc^2)/4))*(delta_B + 1)*(2*e_xc + (2*e_xc*cos(u_c - atan2(e_yc, e_xc) + (13*sin(3*u_c - 3*atan2(e_yc, e_xc))*(e_xc^2 + e_yc^2)^(3/2))/12 + sin(u_c - atan2(e_yc, e_xc))*(2*(e_xc^2 + e_yc^2)^(1/2) - (e_xc^2 + e_yc^2)^(3/2)/4) + sin(2*u_c - 2*atan2(e_yc, e_xc))*((5*e_xc^2)/4 + (5*e_yc^2)/4)))/(e_xc^2 + e_yc^2)^(1/2) - 2*sin(u_c - atan2(e_yc, e_xc) + (13*sin(3*u_c - 3*atan2(e_yc, e_xc))*(e_xc^2 + e_yc^2)^(3/2))/12 + sin(u_c - atan2(e_yc, e_xc))*(2*(e_xc^2 + e_yc^2)^(1/2) - (e_xc^2 + e_yc^2)^(3/2)/4) + sin(2*u_c - 2*atan2(e_yc, e_xc))*((5*e_xc^2)/4 + (5*e_yc^2)/4))*(e_xc^2 + e_yc^2)^(1/2)*(e_yc/(e_xc^2 + e_yc^2) + sin(u_c - atan2(e_yc, e_xc))*((2*e_xc)/(e_xc^2 + e_yc^2)^(1/2) - (3*e_xc*(e_xc^2 + e_yc^2)^(1/2))/4) + (5*e_xc*sin(2*u_c - 2*atan2(e_yc, e_xc)))/2 + (13*e_yc*cos(3*u_c - 3*atan2(e_yc, e_xc))*(e_xc^2 + e_yc^2)^(1/2))/4 + (13*e_xc*sin(3*u_c - 3*atan2(e_yc, e_xc))*(e_xc^2 + e_yc^2)^(1/2))/4 + (e_yc*cos(u_c - atan2(e_yc, e_xc))*(2*(e_xc^2 + e_yc^2)^(1/2) - (e_xc^2 + e_yc^2)^(3/2)/4))/(e_xc^2 + e_yc^2) + (2*e_yc*cos(2*u_c - 2*atan2(e_yc, e_xc))*((5*e_xc^2)/4 + (5*e_yc^2)/4))/(e_xc^2 + e_yc^2))))/(2*a_c*(e_xc^2 + e_yc^2)^(1/2)*(-mu/(a_c*(e_xc^2 + e_yc^2 - 1)))^(1/2)*(e_xc^2 + e_yc^2 - 1)*(2*cos(u_c - atan2(e_yc, e_xc) + (13*sin(3*u_c - 3*atan2(e_yc, e_xc))*(e_xc^2 + e_yc^2)^(3/2))/12 + sin(u_c - atan2(e_yc, e_xc))*(2*(e_xc^2 + e_yc^2)^(1/2) - (e_xc^2 + e_yc^2)^(3/2)/4) + sin(2*u_c - 2*atan2(e_yc, e_xc))*((5*e_xc^2)/4 + (5*e_yc^2)/4))*(e_xc^2 + e_yc^2)^(1/2) + e_xc^2 + e_yc^2 + 1)^(1/2)) - (2*B_c*e_xc*e_yc*mu*rho*(cos(u_c - atan2(e_yc, e_xc) + (13*sin(3*u_c - 3*atan2(e_yc, e_xc))*(e_xc^2 + e_yc^2)^(3/2))/12 + sin(u_c - atan2(e_yc, e_xc))*(2*(e_xc^2 + e_yc^2)^(1/2) - (e_xc^2 + e_yc^2)^(3/2)/4) + sin(2*u_c - 2*atan2(e_yc, e_xc))*((5*e_xc^2)/4 + (5*e_yc^2)/4)) + (e_xc^2 + e_yc^2)^(1/2))*(delta_B + 1)*(2*cos(u_c - atan2(e_yc, e_xc) + (13*sin(3*u_c - 3*atan2(e_yc, e_xc))*(e_xc^2 + e_yc^2)^(3/2))/12 + sin(u_c - atan2(e_yc, e_xc))*(2*(e_xc^2 + e_yc^2)^(1/2) - (e_xc^2 + e_yc^2)^(3/2)/4) + sin(2*u_c - 2*atan2(e_yc, e_xc))*((5*e_xc^2)/4 + (5*e_yc^2)/4))*(e_xc^2 + e_yc^2)^(1/2) + e_xc^2 + e_yc^2 + 1)^(1/2))/(a_c*(e_xc^2 + e_yc^2)^(1/2)*(-mu/(a_c*(e_xc^2 + e_yc^2 - 1)))^(1/2)*(e_xc^2 + e_yc^2 - 1)^2) - (B_c*e_xc*e_yc*mu*rho*(cos(u_c - atan2(e_yc, e_xc) + (13*sin(3*u_c - 3*atan2(e_yc, e_xc))*(e_xc^2 + e_yc^2)^(3/2))/12 + sin(u_c - atan2(e_yc, e_xc))*(2*(e_xc^2 + e_yc^2)^(1/2) - (e_xc^2 + e_yc^2)^(3/2)/4) + sin(2*u_c - 2*atan2(e_yc, e_xc))*((5*e_xc^2)/4 + (5*e_yc^2)/4)) + (e_xc^2 + e_yc^2)^(1/2))*(delta_B + 1)*(2*cos(u_c - atan2(e_yc, e_xc) + (13*sin(3*u_c - 3*atan2(e_yc, e_xc))*(e_xc^2 + e_yc^2)^(3/2))/12 + sin(u_c - atan2(e_yc, e_xc))*(2*(e_xc^2 + e_yc^2)^(1/2) - (e_xc^2 + e_yc^2)^(3/2)/4) + sin(2*u_c - 2*atan2(e_yc, e_xc))*((5*e_xc^2)/4 + (5*e_yc^2)/4))*(e_xc^2 + e_yc^2)^(1/2) + e_xc^2 + e_yc^2 + 1)^(1/2))/(a_c*(e_xc^2 + e_yc^2)^(3/2)*(-mu/(a_c*(e_xc^2 + e_yc^2 - 1)))^(1/2)*(e_xc^2 + e_yc^2 - 1)) + (B_c*e_xc*mu*rho*cos(u_c - atan2(e_yc, e_xc) + (13*sin(3*u_c - 3*atan2(e_yc, e_xc))*(e_xc^2 + e_yc^2)^(3/2))/12 + sin(u_c - atan2(e_yc, e_xc))*(2*(e_xc^2 + e_yc^2)^(1/2) - (e_xc^2 + e_yc^2)^(3/2)/4) + sin(2*u_c - 2*atan2(e_yc, e_xc))*((5*e_xc^2)/4 + (5*e_yc^2)/4))*(delta_B + 1)*(2*cos(u_c - atan2(e_yc, e_xc) + (13*sin(3*u_c - 3*atan2(e_yc, e_xc))*(e_xc^2 + e_yc^2)^(3/2))/12 + sin(u_c - atan2(e_yc, e_xc))*(2*(e_xc^2 + e_yc^2)^(1/2) - (e_xc^2 + e_yc^2)^(3/2)/4) + sin(2*u_c - 2*atan2(e_yc, e_xc))*((5*e_xc^2)/4 + (5*e_yc^2)/4))*(e_xc^2 + e_yc^2)^(1/2) + e_xc^2 + e_yc^2 + 1)^(1/2)*(e_yc/(e_xc^2 + e_yc^2) + sin(u_c - atan2(e_yc, e_xc))*((2*e_xc)/(e_xc^2 + e_yc^2)^(1/2) - (3*e_xc*(e_xc^2 + e_yc^2)^(1/2))/4) + (5*e_xc*sin(2*u_c - 2*atan2(e_yc, e_xc)))/2 + (13*e_yc*cos(3*u_c - 3*atan2(e_yc, e_xc))*(e_xc^2 + e_yc^2)^(1/2))/4 + (13*e_xc*sin(3*u_c - 3*atan2(e_yc, e_xc))*(e_xc^2 + e_yc^2)^(1/2))/4 + (e_yc*cos(u_c - atan2(e_yc, e_xc))*(2*(e_xc^2 + e_yc^2)^(1/2) - (e_xc^2 + e_yc^2)^(3/2)/4))/(e_xc^2 + e_yc^2) + (2*e_yc*cos(2*u_c - 2*atan2(e_yc, e_xc))*((5*e_xc^2)/4 + (5*e_yc^2)/4))/(e_xc^2 + e_yc^2)))/(a_c*(e_xc^2 + e_yc^2)^(1/2)*(-mu/(a_c*(e_xc^2 + e_yc^2 - 1)))^(1/2)*(e_xc^2 + e_yc^2 - 1)) + (B_c*e_yc*mu*rho*(cos(u_c - atan2(e_yc, e_xc) + (13*sin(3*u_c - 3*atan2(e_yc, e_xc))*(e_xc^2 + e_yc^2)^(3/2))/12 + sin(u_c - atan2(e_yc, e_xc))*(2*(e_xc^2 + e_yc^2)^(1/2) - (e_xc^2 + e_yc^2)^(3/2)/4) + sin(2*u_c - 2*atan2(e_yc, e_xc))*((5*e_xc^2)/4 + (5*e_yc^2)/4)) + (e_xc^2 + e_yc^2)^(1/2))*(delta_B + 1)*(2*e_xc + (2*e_xc*cos(u_c - atan2(e_yc, e_xc) + (13*sin(3*u_c - 3*atan2(e_yc, e_xc))*(e_xc^2 + e_yc^2)^(3/2))/12 + sin(u_c - atan2(e_yc, e_xc))*(2*(e_xc^2 + e_yc^2)^(1/2) - (e_xc^2 + e_yc^2)^(3/2)/4) + sin(2*u_c - 2*atan2(e_yc, e_xc))*((5*e_xc^2)/4 + (5*e_yc^2)/4)))/(e_xc^2 + e_yc^2)^(1/2) - 2*sin(u_c - atan2(e_yc, e_xc) + (13*sin(3*u_c - 3*atan2(e_yc, e_xc))*(e_xc^2 + e_yc^2)^(3/2))/12 + sin(u_c - atan2(e_yc, e_xc))*(2*(e_xc^2 + e_yc^2)^(1/2) - (e_xc^2 + e_yc^2)^(3/2)/4) + sin(2*u_c - 2*atan2(e_yc, e_xc))*((5*e_xc^2)/4 + (5*e_yc^2)/4))*(e_xc^2 + e_yc^2)^(1/2)*(e_yc/(e_xc^2 + e_yc^2) + sin(u_c - atan2(e_yc, e_xc))*((2*e_xc)/(e_xc^2 + e_yc^2)^(1/2) - (3*e_xc*(e_xc^2 + e_yc^2)^(1/2))/4) + (5*e_xc*sin(2*u_c - 2*atan2(e_yc, e_xc)))/2 + (13*e_yc*cos(3*u_c - 3*atan2(e_yc, e_xc))*(e_xc^2 + e_yc^2)^(1/2))/4 + (13*e_xc*sin(3*u_c - 3*atan2(e_yc, e_xc))*(e_xc^2 + e_yc^2)^(1/2))/4 + (e_yc*cos(u_c - atan2(e_yc, e_xc))*(2*(e_xc^2 + e_yc^2)^(1/2) - (e_xc^2 + e_yc^2)^(3/2)/4))/(e_xc^2 + e_yc^2) + (2*e_yc*cos(2*u_c - 2*atan2(e_yc, e_xc))*((5*e_xc^2)/4 + (5*e_yc^2)/4))/(e_xc^2 + e_yc^2))))/(2*a_c*(e_xc^2 + e_yc^2)^(1/2)*(-mu/(a_c*(e_xc^2 + e_yc^2 - 1)))^(1/2)*(e_xc^2 + e_yc^2 - 1)*(2*cos(u_c - atan2(e_yc, e_xc) + (13*sin(3*u_c - 3*atan2(e_yc, e_xc))*(e_xc^2 + e_yc^2)^(3/2))/12 + sin(u_c - atan2(e_yc, e_xc))*(2*(e_xc^2 + e_yc^2)^(1/2) - (e_xc^2 + e_yc^2)^(3/2)/4) + sin(2*u_c - 2*atan2(e_yc, e_xc))*((5*e_xc^2)/4 + (5*e_yc^2)/4))*(e_xc^2 + e_yc^2)^(1/2) + e_xc^2 + e_yc^2 + 1)^(1/2)) - (B_c*e_xc*e_yc*mu^2*rho*(cos(u_c - atan2(e_yc, e_xc) + (13*sin(3*u_c - 3*atan2(e_yc, e_xc))*(e_xc^2 + e_yc^2)^(3/2))/12 + sin(u_c - atan2(e_yc, e_xc))*(2*(e_xc^2 + e_yc^2)^(1/2) - (e_xc^2 + e_yc^2)^(3/2)/4) + sin(2*u_c - 2*atan2(e_yc, e_xc))*((5*e_xc^2)/4 + (5*e_yc^2)/4)) + (e_xc^2 + e_yc^2)^(1/2))*(delta_B + 1)*(2*cos(u_c - atan2(e_yc, e_xc) + (13*sin(3*u_c - 3*atan2(e_yc, e_xc))*(e_xc^2 + e_yc^2)^(3/2))/12 + sin(u_c - atan2(e_yc, e_xc))*(2*(e_xc^2 + e_yc^2)^(1/2) - (e_xc^2 + e_yc^2)^(3/2)/4) + sin(2*u_c - 2*atan2(e_yc, e_xc))*((5*e_xc^2)/4 + (5*e_yc^2)/4))*(e_xc^2 + e_yc^2)^(1/2) + e_xc^2 + e_yc^2 + 1)^(1/2))/(a_c^2*(e_xc^2 + e_yc^2)^(1/2)*(-mu/(a_c*(e_xc^2 + e_yc^2 - 1)))^(3/2)*(e_xc^2 + e_yc^2 - 1)^3);
